simulink model "FeedBack_Linearization"  (R2021b)
(part 7 of 9)

et595 = ct{386};
et596 = ct{387};
et597 = ct{388};
et598 = ct{389};
et599 = ct{390};
et600 = ct{391};
et601 = ct{392};
et602 = ct{393};
et603 = ct{394};
et604 = ct{395};
et605 = ct{396};
et606 = ct{397};
et607 = ct{398};
et608 = ct{399};
et609 = ct{400};
et610 = ct{401};
et611 = ct{402};
et612 = ct{403};
et613 = ct{404};
et614 = ct{405};
et615 = ct{406};
et616 = ct{407};
et617 = ct{408};
et618 = ct{409};
et619 = ct{410};
et620 = ct{411};
et621 = ct{412};
et622 = ct{413};
et623 = ct{414};
et624 = ct{415};
et625 = ct{416};
et626 = ct{417};
et627 = ct{418};
et628 = ct{419};
et629 = ct{420};
et630 = ct{421};
et631 = ct{422};
et632 = ct{423};
et633 = ct{424};
et634 = ct{425};
et635 = ct{426};
et636 = ct{427};
et637 = ct{428};
et638 = ct{429};
et639 = ct{430};
et640 = ct{431};
et641 = ct{432};
et642 = ct{433};
et643 = ct{434};
et644 = ct{435};
et645 = ct{436};
et646 = ct{437};
et647 = ct{438};
et648 = ct{439};
et649 = ct{440};
et650 = ct{441};
et651 = ct{442};
et652 = ct{443};
et653 = ct{444};
et654 = ct{445};
et655 = ct{446};
et656 = ct{447};
t10 = ct{448};
t1001 = ct{449};
t1012 = ct{450};
t1015 = ct{451};
t1016 = ct{452};
t1017 = ct{453};
t1018 = ct{454};
t1020 = ct{455};
t1021 = ct{456};
t1022 = ct{457};
t1023 = ct{458};
t1024 = ct{459};
t1025 = ct{460};
t1034 = ct{461};
t1036 = ct{462};
t1040 = ct{463};
t1041 = ct{464};
t1051 = ct{465};
t1052 = ct{466};
t1053 = ct{467};
t1054 = ct{468};
t1055 = ct{469};
t1056 = ct{470};
t1059 = ct{471};
t1060 = ct{472};
t1066 = ct{473};
t1067 = ct{474};
t1069 = ct{475};
t107 = ct{476};
t1070 = ct{477};
t1072 = ct{478};
t1075 = ct{479};
t1077 = ct{480};
t1079 = ct{481};
t1081 = ct{482};
t1088 = ct{483};
t1093 = ct{484};
t1094 = ct{485};
t1096 = ct{486};
t1097 = ct{487};
t11 = ct{488};
t1110 = ct{489};
t1113 = ct{490};
t1114 = ct{491};
t1115 = ct{492};
t1123 = ct{493};
t1125 = ct{494};
t1126 = ct{495};
t1128 = ct{496};
t1130 = ct{497};
t1132 = ct{498};
t1136 = ct{499};
t1137 = ct{500};
t114 = ct{501};
t1159 = ct{502};
t1161 = ct{503};
t1172 = ct{504};
t1175 = ct{505};
t1178 = ct{506};
t1179 = ct{507};
t1189 = ct{508};
t1190 = ct{509};
t12 = ct{510};
t1206 = ct{511};
t1207 = ct{512};
t1209 = ct{513};
t1211 = ct{514};
t1212 = ct{515};
t1213 = ct{516};
t1214 = ct{517};
t1215 = ct{518};
t1218 = ct{519};
t1219 = ct{520};
t122 = ct{521};
t1220 = ct{522};
t1226 = ct{523};
t1231 = ct{524};
t1256 = ct{525};
t1267 = ct{526};
t1268 = ct{527};
t1269 = ct{528};
t1273 = ct{529};
t1286 = ct{530};
t1295 = ct{531};
t1296 = ct{532};
t1299 = ct{533};
t13 = ct{534};
t130 = ct{535};
t1304 = ct{536};
t1312 = ct{537};
t1313 = ct{538};
t1315 = ct{539};
t1329 = ct{540};
t1330 = ct{541};
t1339 = ct{542};
t1347 = ct{543};
t1350 = ct{544};
t1351 = ct{545};
t1352 = ct{546};
t1360 = ct{547};
t1368 = ct{548};
t1369 = ct{549};
t1374 = ct{550};
t1375 = ct{551};
t1386 = ct{552};
t1387 = ct{553};
t1389 = ct{554};
t139 = ct{555};
t1391 = ct{556};
t14 = ct{557};
t1424 = ct{558};
t1431 = ct{559};
t1435 = ct{560};
t1441 = ct{561};
t1456 = ct{562};
t1462 = ct{563};
t1467 = ct{564};
t1487 = ct{565};
t1489 = ct{566};
t149 = ct{567};
t1497 = ct{568};
t1498 = ct{569};
t15 = ct{570};
t1506 = ct{571};
t1515 = ct{572};
t1516 = ct{573};
t152 = ct{574};
t1526 = ct{575};
t1528 = ct{576};
t1529 = ct{577};
t1543 = ct{578};
t1546 = ct{579};
t1553 = ct{580};
t1554 = ct{581};
t1569 = ct{582};
t1574 = ct{583};
t1577 = ct{584};
t1578 = ct{585};
t1579 = ct{586};
t1581 = ct{587};
t1582 = ct{588};
t1591 = ct{589};
t160 = ct{590};
t1601 = ct{591};
t1603 = ct{592};
t1604 = ct{593};
t1605 = ct{594};
t1616 = ct{595};
t1622 = ct{596};
t1625 = ct{597};
t1633 = ct{598};
t1635 = ct{599};
t1636 = ct{600};
t1638 = ct{601};
t1643 = ct{602};
t1644 = ct{603};
t1648 = ct{604};
t1649 = ct{605};
t165 = ct{606};
t1654 = ct{607};
t1655 = ct{608};
t1657 = ct{609};
t1658 = ct{610};
t1660 = ct{611};
t1661 = ct{612};
t1662 = ct{613};
t1667 = ct{614};
t1668 = ct{615};
t1672 = ct{616};
t1675 = ct{617};
t1679 = ct{618};
t1681 = ct{619};
t1682 = ct{620};
t1685 = ct{621};
t1686 = ct{622};
t1687 = ct{623};
t1688 = ct{624};
t1697 = ct{625};
t17 = ct{626};
t1700 = ct{627};
t1701 = ct{628};
t1702 = ct{629};
t1707 = ct{630};
t1710 = ct{631};
t1711 = ct{632};
t1715 = ct{633};
t1717 = ct{634};
t1718 = ct{635};
t1719 = ct{636};
t1720 = ct{637};
t1721 = ct{638};
t1723 = ct{639};
t1726 = ct{640};
t1729 = ct{641};
t1734 = ct{642};
t1736 = ct{643};
t1738 = ct{644};
t1742 = ct{645};
t1745 = ct{646};
t1746 = ct{647};
t1748 = ct{648};
t1749 = ct{649};
t1750 = ct{650};
t1751 = ct{651};
t1753 = ct{652};
t1755 = ct{653};
t1760 = ct{654};
t1762 = ct{655};
t1765 = ct{656};
t1766 = ct{657};
t1769 = ct{658};
t1770 = ct{659};
t1771 = ct{660};
t1772 = ct{661};
t1774 = ct{662};
t1776 = ct{663};
t1778 = ct{664};
t1779 = ct{665};
t1791 = ct{666};
t1792 = ct{667};
t1795 = ct{668};
t1798 = ct{669};
t1799 = ct{670};
t180 = ct{671};
t1800 = ct{672};
t1801 = ct{673};
t1802 = ct{674};
t1804 = ct{675};
t1805 = ct{676};
t1806 = ct{677};
t1811 = ct{678};
t1812 = ct{679};
t1814 = ct{680};
t1816 = ct{681};
t1817 = ct{682};
t1819 = ct{683};
t182 = ct{684};
t1822 = ct{685};
t1823 = ct{686};
t1830 = ct{687};
t1836 = ct{688};
t1839 = ct{689};
t1840 = ct{690};
t1842 = ct{691};
t1843 = ct{692};
t1846 = ct{693};
t1849 = ct{694};
t1851 = ct{695};
t1852 = ct{696};
t1853 = ct{697};
t1856 = ct{698};
t1859 = ct{699};
t186 = ct{700};
t1860 = ct{701};
t1861 = ct{702};
t1863 = ct{703};
t1865 = ct{704};
t1866 = ct{705};
t1867 = ct{706};
t1872 = ct{707};
t1873 = ct{708};
t1874 = ct{709};
t1875 = ct{710};
t1876 = ct{711};
t1880 = ct{712};
t1881 = ct{713};
t1883 = ct{714};
t1886 = ct{715};
t1888 = ct{716};
t1889 = ct{717};
t189 = ct{718};
t1890 = ct{719};
t1893 = ct{720};
t1896 = ct{721};
t1898 = ct{722};
t1902 = ct{723};
t1905 = ct{724};
t1908 = ct{725};
t1911 = ct{726};
t1914 = ct{727};
t1917 = ct{728};
t1919 = ct{729};
t1924 = ct{730};
t1927 = ct{731};
t1928 = ct{732};
t1931 = ct{733};
t1932 = ct{734};
t1934 = ct{735};
t1940 = ct{736};
t1942 = ct{737};
t1950 = ct{738};
t1951 = ct{739};
t1953 = ct{740};
t1957 = ct{741};
t1959 = ct{742};
t1960 = ct{743};
t1962 = ct{744};
t1963 = ct{745};
t1969 = ct{746};
t1976 = ct{747};
t1985 = ct{748};
t1993 = ct{749};
t2 = ct{750};
t2000 = ct{751};
t2001 = ct{752};
t2002 = ct{753};
t2003 = ct{754};
t2006 = ct{755};
t2008 = ct{756};
t2010 = ct{757};
t2018 = ct{758};
t2022 = ct{759};
t2026 = ct{760};
t2035 = ct{761};
t2036 = ct{762};
t2041 = ct{763};
t2042 = ct{764};
t2044 = ct{765};
t2046 = ct{766};
t2051 = ct{767};
t2056 = ct{768};
t2058 = ct{769};
t2065 = ct{770};
t2066 = ct{771};
t2071 = ct{772};
t2072 = ct{773};
t2073 = ct{774};
t2074 = ct{775};
t2075 = ct{776};
t2076 = ct{777};
t208 = ct{778};
t2080 = ct{779};
t2081 = ct{780};
t2085 = ct{781};
t2088 = ct{782};
t2089 = ct{783};
t2090 = ct{784};
t2095 = ct{785};
t2096 = ct{786};
t2108 = ct{787};
t2109 = ct{788};
t2111 = ct{789};
t2115 = ct{790};
t2119 = ct{791};
t2125 = ct{792};
t2130 = ct{793};
t2139 = ct{794};
t2147 = ct{795};
t2148 = ct{796};
t2149 = ct{797};
t2151 = ct{798};
t2152 = ct{799};
t2163 = ct{800};
t2164 = ct{801};
t2165 = ct{802};
t2171 = ct{803};
t2173 = ct{804};
t2177 = ct{805};
t2179 = ct{806};
t2180 = ct{807};
t2181 = ct{808};
t2182 = ct{809};
t2183 = ct{810};
t2184 = ct{811};
t2187 = ct{812};
t2196 = ct{813};
t2198 = ct{814};
t2203 = ct{815};
t2205 = ct{816};
t2206 = ct{817};
t2207 = ct{818};
t2208 = ct{819};
t221 = ct{820};
t2212 = ct{821};
t2215 = ct{822};
t2217 = ct{823};
t2219 = ct{824};
t2220 = ct{825};
t2224 = ct{826};
t2227 = ct{827};
t2228 = ct{828};
t223 = ct{829};
t2231 = ct{830};
t2240 = ct{831};
t2246 = ct{832};
t2253 = ct{833};
t2256 = ct{834};
t2258 = ct{835};
t2259 = ct{836};
t2261 = ct{837};
t2262 = ct{838};
t2263 = ct{839};
t2264 = ct{840};
t2266 = ct{841};
t2269 = ct{842};
t2289 = ct{843};
t2296 = ct{844};
t23 = ct{845};
t230 = ct{846};
t2300 = ct{847};
t2301 = ct{848};
t2315 = ct{849};
t2323 = ct{850};
t2326 = ct{851};
t2330 = ct{852};
t234 = ct{853};
t2341 = ct{854};
t2343 = ct{855};
t235 = ct{856};
t2350 = ct{857};
t2351 = ct{858};
t2352 = ct{859};
t2356 = ct{860};
t2357 = ct{861};
t2359 = ct{862};
t236 = ct{863};
t2360 = ct{864};
t2363 = ct{865};
t2365 = ct{866};
t2369 = ct{867};
t237 = ct{868};
t2370 = ct{869};
t2372 = ct{870};
t2374 = ct{871};
t2375 = ct{872};
t2376 = ct{873};
t2379 = ct{874};
t238 = ct{875};
t2380 = ct{876};
t2382 = ct{877};
t2383 = ct{878};
t2384 = ct{879};
t2385 = ct{880};
t2387 = ct{881};
t2388 = ct{882};
t239 = ct{883};
t2392 = ct{884};
t2393 = ct{885};
t2395 = ct{886};
t2399 = ct{887};
t24 = ct{888};
t2400 = ct{889};
t2402 = ct{890};
t2404 = ct{891};
t2407 = ct{892};
t2411 = ct{893};
t2418 = ct{894};
t2429 = ct{895};
t243 = ct{896};
t2435 = ct{897};
t2439 = ct{898};
t244 = ct{899};
t2444 = ct{900};
t2445 = ct{901};
t2447 = ct{902};
t2455 = ct{903};
t2456 = ct{904};
t2460 = ct{905};
t2462 = ct{906};
t2463 = ct{907};
t2466 = ct{908};
t2467 = ct{909};
t2477 = ct{910};
t2482 = ct{911};
t2483 = ct{912};
t2488 = ct{913};
t2496 = ct{914};
t25 = ct{915};
t2501 = ct{916};
t2503 = ct{917};
t2507 = ct{918};
t2513 = ct{919};
t2514 = ct{920};
t2516 = ct{921};
t252 = ct{922};
t2521 = ct{923};
t2522 = ct{924};
t2523 = ct{925};
t253 = ct{926};
t2533 = ct{927};
t2536 = ct{928};
t2537 = ct{929};
t254 = ct{930};
t2541 = ct{931};
t2554 = ct{932};
t2558 = ct{933};
t2560 = ct{934};
t2561 = ct{935};
t2563 = ct{936};
t2569 = ct{937};
t2570 = ct{938};
t2571 = ct{939};
t2576 = ct{940};
t2581 = ct{941};
t2584 = ct{942};
t2585 = ct{943};
t2587 = ct{944};
t259 = ct{945};
t2590 = ct{946};
t2591 = ct{947};
t26 = ct{948};
t2601 = ct{949};
t2602 = ct{950};
t2604 = ct{951};
t2609 = ct{952};
t2610 = ct{953};
t2611 = ct{954};
t2612 = ct{955};
t2613 = ct{956};
t2614 = ct{957};
t2615 = ct{958};
t2617 = ct{959};
t2618 = ct{960};
t2620 = ct{961};
t2621 = ct{962};
t2624 = ct{963};
t2627 = ct{964};
t2631 = ct{965};
t2634 = ct{966};
t2635 = ct{967};
t2637 = ct{968};
t2638 = ct{969};
t2647 = ct{970};
t2648 = ct{971};
t2651 = ct{972};
t2652 = ct{973};
t2653 = ct{974};
t2654 = ct{975};
t2655 = ct{976};
t2656 = ct{977};
t2659 = ct{978};
t2661 = ct{979};
t2662 = ct{980};
t2663 = ct{981};
t2664 = ct{982};
t2667 = ct{983};
t2670 = ct{984};
t2671 = ct{985};
t2672 = ct{986};
t2674 = ct{987};
t2675 = ct{988};
t2677 = ct{989};
t2679 = ct{990};
t268 = ct{991};
t2684 = ct{992};
t2687 = ct{993};
t2689 = ct{994};
t269 = ct{995};
t2690 = ct{996};
t2691 = ct{997};
t2692 = ct{998};
t2693 = ct{999};
t2697 = ct{1000};
t2698 = ct{1001};
t2699 = ct{1002};
t27 = ct{1003};
t2700 = ct{1004};
t2701 = ct{1005};
t2703 = ct{1006};
t2707 = ct{1007};
t2708 = ct{1008};
t2710 = ct{1009};
t2711 = ct{1010};
t2714 = ct{1011};
t2720 = ct{1012};
t2721 = ct{1013};
t2722 = ct{1014};
t2723 = ct{1015};
t2726 = ct{1016};
t2727 = ct{1017};
t2728 = ct{1018};
t2729 = ct{1019};
t2732 = ct{1020};
t2734 = ct{1021};
t2735 = ct{1022};
t2737 = ct{1023};
t2738 = ct{1024};
t2739 = ct{1025};
t2740 = ct{1026};
t2741 = ct{1027};
t2742 = ct{1028};
t2743 = ct{1029};
t2744 = ct{1030};
t2747 = ct{1031};
t2751 = ct{1032};
t2753 = ct{1033};
t2754 = ct{1034};
t2756 = ct{1035};
t2765 = ct{1036};
t2781 = ct{1037};
t2783 = ct{1038};
t2788 = ct{1039};
t2789 = ct{1040};
t279 = ct{1041};
t2790 = ct{1042};
t2792 = ct{1043};
t2795 = ct{1044};
t2796 = ct{1045};
t2797 = ct{1046};
t2798 = ct{1047};
t2799 = ct{1048};
t28 = ct{1049};
t280 = ct{1050};
t2801 = ct{1051};
t2803 = ct{1052};
t2804 = ct{1053};
t2807 = ct{1054};
t2810 = ct{1055};
t2811 = ct{1056};
t2813 = ct{1057};
t2814 = ct{1058};
t2816 = ct{1059};
t2817 = ct{1060};
t2818 = ct{1061};
t2823 = ct{1062};
t2825 = ct{1063};
t2828 = ct{1064};
t2829 = ct{1065};
t2832 = ct{1066};
t2837 = ct{1067};
t2838 = ct{1068};
t2839 = ct{1069};
t284 = ct{1070};
t2840 = ct{1071};
t2841 = ct{1072};
t2842 = ct{1073};
t2844 = ct{1074};
t2854 = ct{1075};
t2857 = ct{1076};
t2861 = ct{1077};
t2864 = ct{1078};
t2868 = ct{1079};
t287 = ct{1080};
t2883 = ct{1081};
t2884 = ct{1082};
t2891 = ct{1083};
t29 = ct{1084};
t290 = ct{1085};
t2900 = ct{1086};
t2907 = ct{1087};
t2914 = ct{1088};
t2922 = ct{1089};
t2923 = ct{1090};
t2925 = ct{1091};
t293 = ct{1092};
t2930 = ct{1093};
t2931 = ct{1094};
t2935 = ct{1095};
t2936 = ct{1096};
t2939 = ct{1097};
t2941 = ct{1098};
t2942 = ct{1099};
t2943 = ct{1100};
t2944 = ct{1101};
t2945 = ct{1102};
t2946 = ct{1103};
t2948 = ct{1104};
t2949 = ct{1105};
t295 = ct{1106};
t2950 = ct{1107};
t2953 = ct{1108};
t2954 = ct{1109};
t2955 = ct{1110};
t2956 = ct{1111};
t2957 = ct{1112};
t296 = ct{1113};
t2960 = ct{1114};
t2961 = ct{1115};
t2962 = ct{1116};
t297 = ct{1117};
t2972 = ct{1118};
t2974 = ct{1119};
t298 = ct{1120};
t2989 = ct{1121};
t2991 = ct{1122};
t2996 = ct{1123};
t2997 = ct{1124};
t2998 = ct{1125};
t2999 = ct{1126};
t3 = ct{1127};
t30 = ct{1128};
t3008 = ct{1129};
t3009 = ct{1130};
t301 = ct{1131};
t3011 = ct{1132};
t3020 = ct{1133};
t3031 = ct{1134};
t3035 = ct{1135};
t3038 = ct{1136};
t3039 = ct{1137};
t3040 = ct{1138};
t3041 = ct{1139};
t3042 = ct{1140};
t3045 = ct{1141};
t3047 = ct{1142};
t3048 = ct{1143};
t3051 = ct{1144};
t3052 = ct{1145};
t3060 = ct{1146};
t3066 = ct{1147};
t3067 = ct{1148};
t3071 = ct{1149};
t3075 = ct{1150};
t3076 = ct{1151};
t3082 = ct{1152};
t3083 = ct{1153};
t3085 = ct{1154};
t3086 = ct{1155};
t3088 = ct{1156};
t3092 = ct{1157};
t3097 = ct{1158};
t3098 = ct{1159};
t3099 = ct{1160};
t31 = ct{1161};
t3104 = ct{1162};
t3107 = ct{1163};
t3112 = ct{1164};
t3113 = ct{1165};
t3120 = ct{1166};
t3121 = ct{1167};
t3122 = ct{1168};
t3124 = ct{1169};
t3126 = ct{1170};
t3128 = ct{1171};
t3130 = ct{1172};
t3131 = ct{1173};
t3132 = ct{1174};
t3133 = ct{1175};
t3140 = ct{1176};
t3141 = ct{1177};
t3142 = ct{1178};
t3143 = ct{1179};
t3148 = ct{1180};
t3152 = ct{1181};
t3153 = ct{1182};
t3154 = ct{1183};
t3155 = ct{1184};
t3159 = ct{1185};
t3161 = ct{1186};
t3162 = ct{1187};
t3163 = ct{1188};
t3165 = ct{1189};
t3166 = ct{1190};
t3168 = ct{1191};
t317 = ct{1192};
t3170 = ct{1193};
t3171 = ct{1194};
t3172 = ct{1195};
t3175 = ct{1196};
t3179 = ct{1197};
t318 = ct{1198};
t3181 = ct{1199};
t3186 = ct{1200};
t319 = ct{1201};
t3190 = ct{1202};
t3192 = ct{1203};
t3193 = ct{1204};
t3194 = ct{1205};
t3195 = ct{1206};
t3196 = ct{1207};
t32 = ct{1208};
t320 = ct{1209};
t3201 = ct{1210};
t3202 = ct{1211};
t3203 = ct{1212};
t3204 = ct{1213};
t3205 = ct{1214};
t3215 = ct{1215};
t3226 = ct{1216};
t3229 = ct{1217};
t3232 = ct{1218};
t3235 = ct{1219};
t3238 = ct{1220};
t3246 = ct{1221};
t3248 = ct{1222};
t3249 = ct{1223};
t3252 = ct{1224};
t3253 = ct{1225};
t3255 = ct{1226};
t3257 = ct{1227};
t3260 = ct{1228};
t3261 = ct{1229};
t3262 = ct{1230};
t3263 = ct{1231};
t3264 = ct{1232};
t3268 = ct{1233};
t3269 = ct{1234};
t3272 = ct{1235};
t3273 = ct{1236};
t3277 = ct{1237};
t3279 = ct{1238};
t3280 = ct{1239};
t3284 = ct{1240};
t3288 = ct{1241};
t3289 = ct{1242};
t329 = ct{1243};
t3290 = ct{1244};
t3291 = ct{1245};
t3292 = ct{1246};
t3293 = ct{1247};
t3294 = ct{1248};
t3295 = ct{1249};
t3296 = ct{1250};
t33 = ct{1251};
t330 = ct{1252};
t3301 = ct{1253};
t331 = ct{1254};
t3311 = ct{1255};
t3312 = ct{1256};
t3313 = ct{1257};
t3315 = ct{1258};
t3316 = ct{1259};
t3321 = ct{1260};
t3324 = ct{1261};
t3336 = ct{1262};
t3340 = ct{1263};
t3342 = ct{1264};
t3356 = ct{1265};
t3357 = ct{1266};
t3358 = ct{1267};
t3359 = ct{1268};
t3360 = ct{1269};
t3361 = ct{1270};
t3362 = ct{1271};
t3363 = ct{1272};
t3364 = ct{1273};
t3365 = ct{1274};
t3366 = ct{1275};
t3369 = ct{1276};
t3372 = ct{1277};
t3375 = ct{1278};
t3377 = ct{1279};
t3382 = ct{1280};
t3384 = ct{1281};
t3386 = ct{1282};
t3388 = ct{1283};
t3392 = ct{1284};
t3393 = ct{1285};
t3395 = ct{1286};
t3397 = ct{1287};
t3398 = ct{1288};
t34 = ct{1289};
t3400 = ct{1290};
t3402 = ct{1291};
t3403 = ct{1292};
t3406 = ct{1293};
t3407 = ct{1294};
t3411 = ct{1295};
t3413 = ct{1296};
t3414 = ct{1297};
t3417 = ct{1298};
t3418 = ct{1299};
t342 = ct{1300};
t3421 = ct{1301};
t3422 = ct{1302};
t3424 = ct{1303};
t3426 = ct{1304};
t3429 = ct{1305};
t3433 = ct{1306};
t3436 = ct{1307};
t3437 = ct{1308};
t3438 = ct{1309};
t3440 = ct{1310};
t3443 = ct{1311};
t3444 = ct{1312};
t3452 = ct{1313};
t346 = ct{1314};
t3460 = ct{1315};
t3468 = ct{1316};
t3470 = ct{1317};
t3476 = ct{1318};
t3479 = ct{1319};
t3480 = ct{1320};
t3481 = ct{1321};
t3482 = ct{1322};
t3483 = ct{1323};
t3486 = ct{1324};
t3488 = ct{1325};
t3489 = ct{1326};
t349 = ct{1327};
t3490 = ct{1328};
t3491 = ct{1329};
t3492 = ct{1330};
t3495 = ct{1331};
t3498 = ct{1332};
t35 = ct{1333};
t3502 = ct{1334};
t3504 = ct{1335};
t3506 = ct{1336};
t3514 = ct{1337};
t3526 = ct{1338};
t3527 = ct{1339};
t3528 = ct{1340};
t3535 = ct{1341};
t3536 = ct{1342};
t3537 = ct{1343};
t3538 = ct{1344};
t3540 = ct{1345};
t3542 = ct{1346};
t3544 = ct{1347};
t3546 = ct{1348};
t3547 = ct{1349};
t3551 = ct{1350};
t3555 = ct{1351};
t3556 = ct{1352};
t3559 = ct{1353};
t3561 = ct{1354};
t36 = ct{1355};
t3610 = ct{1356};
t3617 = ct{1357};
t3618 = ct{1358};
t3619 = ct{1359};
t3620 = ct{1360};
t3625 = ct{1361};
t3626 = ct{1362};
t3627 = ct{1363};
t3628 = ct{1364};
t3640 = ct{1365};
t3641 = ct{1366};
t3642 = ct{1367};
t3643 = ct{1368};
t3644 = ct{1369};
t3645 = ct{1370};
t3646 = ct{1371};
t3648 = ct{1372};
t3649 = ct{1373};
t3651 = ct{1374};
t3652 = ct{1375};
t3653 = ct{1376};
t3654 = ct{1377};
t3655 = ct{1378};
t3658 = ct{1379};
t3660 = ct{1380};
t3661 = ct{1381};
t3662 = ct{1382};
t3663 = ct{1383};
t3664 = ct{1384};
t3665 = ct{1385};
t3666 = ct{1386};
t3667 = ct{1387};
t3668 = ct{1388};
t3669 = ct{1389};
t3670 = ct{1390};
t3671 = ct{1391};
t3672 = ct{1392};
t3673 = ct{1393};
t3674 = ct{1394};
t3679 = ct{1395};
t3685 = ct{1396};
t37 = ct{1397};
t3720 = ct{1398};
t3751 = ct{1399};
t3776 = ct{1400};
t3779 = ct{1401};
t3780 = ct{1402};
t3781 = ct{1403};
t3782 = ct{1404};
t3783 = ct{1405};
t3784 = ct{1406};
t3786 = ct{1407};
t3788 = ct{1408};
t3789 = ct{1409};
t3790 = ct{1410};
t3796 = ct{1411};
t3798 = ct{1412};
t3811 = ct{1413};
t3812 = ct{1414};
t3816 = ct{1415};
t3818 = ct{1416};
t3820 = ct{1417};
t3821 = ct{1418};
t3823 = ct{1419};
t3824 = ct{1420};
t3825 = ct{1421};
t3826 = ct{1422};
t3828 = ct{1423};
t3829 = ct{1424};
t3833 = ct{1425};
t3835 = ct{1426};
t3838 = ct{1427};
t3839 = ct{1428};
t3840 = ct{1429};
t3841 = ct{1430};
t3842 = ct{1431};
t3843 = ct{1432};
t3844 = ct{1433};
t3845 = ct{1434};
t39 = ct{1435};
t4 = ct{1436};
t40 = ct{1437};
t431 = ct{1438};
t433 = ct{1439};
t436 = ct{1440};
t448 = ct{1441};
t45 = ct{1442};
t451 = ct{1443};
t452 = ct{1444};
t455 = ct{1445};
t456 = ct{1446};
t457 = ct{1447};
t458 = ct{1448};
t46 = ct{1449};
t460 = ct{1450};
t461 = ct{1451};
t463 = ct{1452};
t469 = ct{1453};
t49 = ct{1454};
t5 = ct{1455};
t50 = ct{1456};
t51 = ct{1457};
t512 = ct{1458};
t515 = ct{1459};
t516 = ct{1460};
t517 = ct{1461};
t518 = ct{1462};
t522 = ct{1463};
t523 = ct{1464};
t525 = ct{1465};
t527 = ct{1466};
t528 = ct{1467};
t529 = ct{1468};
t530 = ct{1469};
t535 = ct{1470};
t536 = ct{1471};
t537 = ct{1472};
t542 = ct{1473};
t547 = ct{1474};
t548 = ct{1475};
t55 = ct{1476};
t554 = ct{1477};
t567 = ct{1478};
t568 = ct{1479};
t569 = ct{1480};
t57 = ct{1481};
t570 = ct{1482};
t571 = ct{1483};
t572 = ct{1484};
t573 = ct{1485};
t574 = ct{1486};
t58 = ct{1487};
t580 = ct{1488};
t581 = ct{1489};
t583 = ct{1490};
t6 = ct{1491};
t600 = ct{1492};
t601 = ct{1493};
t602 = ct{1494};
t603 = ct{1495};
t604 = ct{1496};
t605 = ct{1497};
t606 = ct{1498};
t607 = ct{1499};
t608 = ct{1500};
t609 = ct{1501};
t61 = ct{1502};
t612 = ct{1503};
t613 = ct{1504};
t614 = ct{1505};
t615 = ct{1506};
t616 = ct{1507};
t617 = ct{1508};
t618 = ct{1509};
t619 = ct{1510};
t621 = ct{1511};
t624 = ct{1512};
t626 = ct{1513};
t629 = ct{1514};
t631 = ct{1515};
t632 = ct{1516};
t633 = ct{1517};
t634 = ct{1518};
t635 = ct{1519};
t637 = ct{1520};
t639 = ct{1521};
t640 = ct{1522};
t642 = ct{1523};
t643 = ct{1524};
t644 = ct{1525};
t646 = ct{1526};
t647 = ct{1527};
t648 = ct{1528};
t649 = ct{1529};
t650 = ct{1530};
t651 = ct{1531};
t652 = ct{1532};
t653 = ct{1533};
t654 = ct{1534};
t656 = ct{1535};
t657 = ct{1536};
t660 = ct{1537};
t661 = ct{1538};
t662 = ct{1539};
t663 = ct{1540};
t664 = ct{1541};
t665 = ct{1542};
t667 = ct{1543};
t67 = ct{1544};
t673 = ct{1545};
t676 = ct{1546};
t677 = ct{1547};
t678 = ct{1548};
t685 = ct{1549};
t687 = ct{1550};
t689 = ct{1551};
t69 = ct{1552};
t691 = ct{1553};
t692 = ct{1554};
t693 = ct{1555};
t694 = ct{1556};
t696 = ct{1557};
t697 = ct{1558};
t698 = ct{1559};
t7 = ct{1560};
t70 = ct{1561};
t702 = ct{1562};
t703 = ct{1563};
t704 = ct{1564};
t705 = ct{1565};
t708 = ct{1566};
t71 = ct{1567};
t72 = ct{1568};
t721 = ct{1569};
t725 = ct{1570};
t726 = ct{1571};
t729 = ct{1572};
t73 = ct{1573};
t730 = ct{1574};
t731 = ct{1575};
t735 = ct{1576};
t743 = ct{1577};
t754 = ct{1578};
t755 = ct{1579};
t756 = ct{1580};
t76 = ct{1581};
t760 = ct{1582};
t762 = ct{1583};
t77 = ct{1584};
t773 = ct{1585};
t774 = ct{1586};
t776 = ct{1587};
t777 = ct{1588};
t778 = ct{1589};
t786 = ct{1590};
t788 = ct{1591};
t79 = ct{1592};
t791 = ct{1593};
t792 = ct{1594};
t795 = ct{1595};
t796 = ct{1596};
t797 = ct{1597};
t8 = ct{1598};
t800 = ct{1599};
t805 = ct{1600};
t806 = ct{1601};
t813 = ct{1602};
t815 = ct{1603};
t817 = ct{1604};
t818 = ct{1605};
t819 = ct{1606};
t82 = ct{1607};
t827 = ct{1608};
t831 = ct{1609};
t835 = ct{1610};
t836 = ct{1611};
t838 = ct{1612};
t839 = ct{1613};
t84 = ct{1614};
t840 = ct{1615};
t841 = ct{1616};
t842 = ct{1617};
t843 = ct{1618};
t846 = ct{1619};
t847 = ct{1620};
t85 = ct{1621};
t853 = ct{1622};
t855 = ct{1623};
t857 = ct{1624};
t859 = ct{1625};
t86 = ct{1626};
t860 = ct{1627};
t863 = ct{1628};
t864 = ct{1629};
t866 = ct{1630};
t870 = ct{1631};
t871 = ct{1632};
t876 = ct{1633};
t877 = ct{1634};
t878 = ct{1635};
t88 = ct{1636};
t880 = ct{1637};
t881 = ct{1638};
t882 = ct{1639};
t884 = ct{1640};
t885 = ct{1641};
t888 = ct{1642};
t889 = ct{1643};
t89 = ct{1644};
t891 = ct{1645};
t896 = ct{1646};
t898 = ct{1647};
t899 = ct{1648};
t9 = ct{1649};
t90 = ct{1650};
t902 = ct{1651};
t907 = ct{1652};
t908 = ct{1653};
t91 = ct{1654};
t911 = ct{1655};
t92 = ct{1656};
t921 = ct{1657};
t926 = ct{1658};
t927 = ct{1659};
t928 = ct{1660};
t930 = ct{1661};
t932 = ct{1662};
t933 = ct{1663};
t935 = ct{1664};
t939 = ct{1665};
t940 = ct{1666};
t942 = ct{1667};
t948 = ct{1668};
t949 = ct{1669};
t952 = ct{1670};
t958 = ct{1671};
t959 = ct{1672};
t966 = ct{1673};
t969 = ct{1674};
t974 = ct{1675};
t975 = ct{1676};
t982 = ct{1677};
t983 = ct{1678};
t984 = ct{1679};
t987 = ct{1680};
t988 = ct{1681};
t992 = ct{1682};
t994 = ct{1683};
et657 = t1295.*t1823.*4.466636216449161e-20+t959.*t2163.*4.466636216449161e-20-t633.*t2816.*9.999999999999998e-6;
et658 = t831.*t2631.*(-9.999999999999998e-6)+t632.*t2832.*9.999999999999998e-6;
et659 = (t243-t786).*(t639-t1128-t2181+dq5.*t13.*(t86-t652)).*(-1.2e-4)-t1070.*(t90-t615).*4.466636216449161e-20;
et660 = t2149.*(t92-t663).*1.2e-4-t2610.*(t88-t617).*9.999999999999998e-6;
et661 = t2828.*(t252-t791).*1.2e-4+t2609.*(t653-t838).*1.2e-4;
et662 = -t3393+t3468-t2343.*(t884+t1578-t2180+t14.*(t639-t1128-t2181+dq5.*t13.*(t86-t652))).*2.900000000000001e-4+t2854.*(t1529+t15.*(t92-t663)).*2.9e-4;
et663 = t3470.*(t1386+t7.*(t88-t617)).*2.900000000000001e-4+t3312.*(t1745+t8.*(t252-t791)).*2.900000000000001e-4;
et664 = t1296.*t3336.*2.9e-4+t1649.*t3619.*2.9e-4;
et665 = t1654.*t3618.*(-2.9e-4)+t2601.*t3120.*2.9e-4;
et666 = t2654.*t3124.*2.9e-4-t2323.*t3617.*2.94e-3;
et667 = t2326.*t3620.*2.94e-3+t2576.*(t1755-t3128+t15.*(t284+t287+t290-t329-t805-t1951)+dq7.*t8.*(t252-t791)).*2.94e-3;
et668 = t2075.*(t958-t2263+dq7.*t1601+t15.*(t642+t896-t1137-t2220)).*(-2.94e-3)+t2074.*(t1036+t1771-t2690+t15.*(t755+t1012-t1905-t2692)).*2.900000000000001e-4;
et669 = t2627.*(t1034-t1750+t2691+t8.*(t755+t1012-t1905-t2692)).*2.94e-3-t2036.*(t631-t885+t1132-t2224).*2.900000000000001e-4;
et670 = t2429+t2672.*(t614+t13.*(t86-t652))-t940.*t2832+t959.*t2816+t2196.*(t90-t615)-t2659.*(t653-t838);
et671 = (-t2447-t2783-t2839+t2841+t3126+t3143+t3232+t2165.*(t92-t663).*1.2e-4+t2828.*(t653-t838).*1.2e-4).*(-1.0./2.0);
et672 = t1296.*(t1529+t15.*(t92-t663)).*(-1.089e-2)-t2075.*(t8.*(t92-t663)+t15.*(t621-t864)).*2.9e-4;
et673 = t1207.*t2036.*2.2e-4+t1654.*t2601.*1.089e-2;
et674 = t1649.*t2654.*(-1.089e-2)+t2074.*t2343.*2.2e-4;
et675 = t2323.*t2576.*(-2.9e-4)+t2326.*t2627.*2.9e-4;
et676 = (t1386+t7.*(t88-t617)).*(t1745+t8.*(t252-t791)).*2.2e-4;
et677 = t2944+t3186-t3205+t1649.*(t878-t1582+t2184+t7.*(t639-t1128-t2181+dq5.*t13.*(t86-t652))).*4.000000000000028e-5+t2196.*(t665+t7.*(t90-t615)).*2.81e-3;
et678 = t3104.*(t614+t13.*(t86-t652)).*(-5.0e-5)+t3099.*(t1386+t7.*(t88-t617)).*4.000000000000028e-5;
et679 = t1685.*t2816.*(-2.81e-3)+t1681.*t2832.*2.81e-3;
et680 = t2000.*t2610.*2.81e-3-t2035.*t2631.*2.81e-3;
et681 = (t243-t786).*(t884+t1578-t2180+t14.*(t639-t1128-t2181+dq5.*t13.*(t86-t652))).*5.0e-5-t3312.*(t252-t791).*5.0e-5;
et682 = t3098.*(t653-t838).*(-5.0e-5)+t817.*(t631-t885+t1132-t2224).*5.0e-5;
et683 = t1296.*(t642+t896-t1137-t2220).*(-4.000000000000028e-5)+t2074.*(t755+t1012-t1873-t2664).*4.000000000000028e-5;
et684 = t1654.*(t1487+t2219-t2864+dq6.*t7.*(t88-t617)).*4.000000000000028e-5;
et685 = (t3104.*(t614+t13.*(t86-t652))-(t243-t786).*(t884+t1578-t2180+t14.*(t639-t1128-t2181+dq5.*t13.*(t86-t652)))+t2854.*(t92-t663)+t3312.*(t252-t791)+t3098.*(t653-t838)-t817.*(t631-t885+t1132-t2224)).*(et230+et231).*(-1.0./2.0)+t3776.*(et232+et233).*3.38795-((t3618.*(t1745+t8.*(t252-t791))-t3313.*(t8.*(t92-t663)+t15.*(t621-t864))+t2036.*t3336-t2343.*t3619-t2576.*t3438+t2627.*(t1034-t1750+t2667+t8.*(t755+t1012-t1873-t2664))).*(et234+et235))./2.0;
et686 = t3610.*(et236+et237+et238+et239+et240+et241+et242+et243+et244).*(-1.0./2.0)-((t3342+t2343.*(t884+t1578-t2180+t14.*(t639-t1128-t2181+dq5.*t13.*(t86-t652)))-t3470.*(t1386+t7.*(t88-t617))-t3312.*(t1745+t8.*(t252-t791))-t2074.*(t1036+t1771-t2690+t15.*(t755+t1012-t1905-t2692))+t2036.*(t631-t885+t1132-t2224)).*(et245+et246))./2.0+et247.*et248;
et687 = t3820.*(t2000.*(t284+t287+t290-t329-t805-t1951)+t2035.*t2671-(t243-t786).*(t878-t1582+t2184+t7.*(t639-t1128-t2181+dq5.*t13.*(t86-t652)))+t2177.*(t621-t864)-t817.*(t642+t896-t1137-t2220)-(t252-t791).*(t1487+t2219-t2864+dq6.*t7.*(t88-t617))).*(-1.0./2.0)-(t3666.*(et249+et250+et251+et252+et253))./2.0-(t3364.*(et254+et255+et256+et257+et258))./2.0+et259.*et260;
et688 = t702.*(t24.*1.16152294893368e-19+t23.*t27.*1.16152294893368e-19+t26.*t27.*1.16152294893368e-19).*(-1.0./2.0)-(t3192.*(et261+et262+et263+et264+et265+et266+et267+et268))./2.0;
et689 = t3779.*(et269+et270).*(3.41e+2./1.0e+2)-t3786.*(et271+et272).*(3.41e+2./1.0e+2)-t3784.*(et273+et274).*(3.41e+2./1.0e+2)+(t3192.*(et275+et276+et277+et278+et279+et280+et281+et282+et283+et284+et285))./2.0-((t573.*t817+t831.*(t243-t786)+(t88-t617).*(t252-t791)).*(et286+et287+et288))./2.0-t3823.*(et289+et290).*3.38795-(et291+et292).*(t221.*(2.1e+1./5.0e+1)+t223.*(2.1e+1./5.0e+1)-t542+t547+t548-t554+t580+t581+t583+t800+t1424+t1726+t1856+t1898+t1934+t2042+t2198+t2231+t2253+t2558+t2581+t2587+t2602+t2991+t2997+t3066+t3075+t3082+t3495+t3498).*3.38795-(t1866.*(et293+et294+et295+et296+et297+et298+et299+et300+et301+et302+et303+et304+et305))./2.0;
et690 = (t1866.*(et306+et307+et308+et309+et310+et311+et312+et313))./2.0-((t3031+t2165.*(t92-t663)+t2828.*(t653-t838)).*(et314+et315+et316+et317+et318+et319+et320))./2.0-t3641.*(et321+et322).*2.61155-t3640.*(et323+et324).*2.61155+((t2854.*(t1529+t15.*(t92-t663))+t1296.*t3336+t1649.*t3619-t1654.*t3618+t2601.*t3120+t2654.*t3124).*(et325+et326))./2.0-t3796.*(et327+et328+et329).*3.5432e-1-(t3272.*(et330+et331+et332+et333+et334+et335+et336))./2.0+(t3476.*(t182+t23.*t72+t26.*t72))./2.0+(t624.*(t1736+t23.*t1717+t26.*t1717))./2.0+(t1025.*(t1751+t23.*t1723+t26.*t1723))./2.0+(t1256.*(t2018+t23.*t2010+t26.*t2010))./2.0;
et691 = t3821.*(et337+et338).*3.5432e-1+(t2384.*(et339+et340+et341+et342+et343+et344+et345+et346))./2.0-(t3826.*(-t573.*t574+t676.*t831+t677.*(t88-t617)))./2.0+(t3788.*(t2356-t607.*t2196+t633.*t2816+t831.*t2631-t632.*t2832+t2610.*(t88-t617)))./2.0-t3776.*(et347+et348).*3.38795+(t3841.*(t1649.*(t614+t13.*(t86-t652))+t1296.*(t92-t663)-t1654.*(t653-t838)))./2.0+(t3546.*(et349+et350+et351+et352+et353))./2.0-t3679.*(et354+et355).*2.61155+((-t2961+t3358+t3312.*(t653-t838)).*(et356+et357+et358+et359+et360+et361+et362+et363+et364))./2.0;
et692 = t3670.*(et365+et366+et367).*(3.41e+2./1.0e+2)-t3671.*(et368+et369+et370).*(3.41e+2./1.0e+2)+((t3124.*(t614+t13.*(t86-t652))+t1296.*t2196-t1654.*t2816+t1649.*t2832+t2854.*(t92-t663)+t3120.*(t653-t838)).*(et371+et372))./2.0-((-t940.*(t614+t13.*(t86-t652))+t959.*(t653-t838)+(t90-t615).*(t92-t663)).*(et373+et374+et375))./2.0;
et693 = t3672.*(t2.*t3.*3.9348e-1+t10.*t29.*2.25e-3-t10.*t31.*3.492e-2).*(-2.4552);
et694 = t3673.*(t3.*t9.*3.9348e-1+t10.*t32.*2.25e-3-t10.*t35.*3.492e-2).*2.4552-(t2533.*(et376+et377+et378+et379+et380+et381+et382+et383))./2.0+(t3783.*(et384+et385+et386+et387+et388))./2.0+((t859-t1791+t1066.*(t86-t652)).*(et389+et390+et391+et392+et393+et394+et395+et396+et397+et398+et399))./2.0;
et695 = t3372.*(et400+et401+et402+et403+et404).*(-1.0./2.0)-(t3838.*(et405+et406+et407+et408+et409))./2.0-((t859-t1791+t1066.*(t86-t652)).*(et410+et411+et412+et413+et414+et415+et416+et417))./2.0+(t2384.*(et418+et419+et420+et421+et422+et423+et424+et425+et426+et427+et428+et429+et430))./2.0-(t3828.*(et431+et432+et433+et434+et435))./2.0+((-t3113+t3418+t2654.*(t884+t1578-t2180+t14.*(t639-t1128-t2181+dq5.*t13.*(t86-t652)))).*(et436+et437+et438+et439+et440+et441+et442+et443))./2.0-(t3788.*(t2356-(t88-t617).*(t284+t287+t290-t329-t805-t1951)+t817.*t1070+t831.*t2671-t2147.*(t243-t786)-t2163.*(t252-t791)))./2.0;
et696 = (t1842+t632.*(t639-t1128-t2181+dq5.*t13.*(t86-t652))+t607.*t2165-t1206.*t1896-t1295.*t1852-t633.*t2828).*(et444+et445).*(-1.0./2.0)-t3790.*(et446+et447).*3.38795+(t3060.*(et448+et449+et450+et451+et452+et453+et454+et455))./2.0+((t2407+t2563+t3085-t3092-t3122+t2147.*(t639-t1128-t2181+dq5.*t13.*(t86-t652))).*(et456+et457+et458+et459+et460))./2.0-((t2056-t2360-t2788-t2807+t3051+t2962.*(t88-t617)).*(et461+et462+et463+et464+et465))./2.0;
et697 = t3641.*(t469+t530+t888.*2.0e-4+t899.*5.267999999999999e-2+t1299+t1347+t1350+t1351+t1389+t1391+t1431+t1441+t1543+t1546+t1605).*2.61155;
et698 = t3640.*(t535+t536+t880.*2.0e-4+t889.*5.267999999999999e-2+t1312+t1313+t1315+t1352+t1467+t1497+t1498+t1506+t1553+t1554+t1577).*2.61155+(t3272.*(et466+et467+et468+et469+et470+et471+et472))./2.0;
et699 = (t3313.*(t8.*(t92-t663)+t15.*(t621-t864))+t2323.*t3617-t2326.*t3620-t2576.*(t1755-t3128+t15.*(t284+t287+t290-t329-t805-t1951)+dq7.*t8.*(t252-t791))+t2075.*(t958-t2263+dq7.*t1601+t15.*(t642+t896-t1137-t2220))-t2627.*(t1034-t1750+t2691+t8.*(t755+t1012-t1905-t2692))).*(et473+et474).*(-1.0./2.0)+((t3140+t3489+t3720+t2832.*(t884+t1578-t2180+t14.*(t639-t1128-t2181+dq5.*t13.*(t86-t652)))+t3436.*(t92-t663)+t3685.*(t653-t838)).*(et475+et476+et477+et478+et479))./2.0-(t3789.*(et480+et481+et482+et483+et484+et485+et486+et487))./2.0;
et700 = (t2326.*(t884+t1578-t2180+t14.*(t639-t1128-t2181+dq5.*t13.*(t86-t652)))+t2854.*(t1529+t15.*(t92-t663))-t2323.*t3312+t2601.*t3098+t2654.*t3104-t2075.*(t631-t885+t1132-t2224)).*(et488+et489).*(-1.0./2.0)+(t3824.*(t572.*t632-t604.*t633+t10.*t11.*t607))./2.0+(t3782.*(et490+et491+et492+et493+et494+et495+et496+et497))./2.0+et498.*et499+et500.*et501+((t3377+t2074.*(t878-t1582+t2184+t7.*(t639-t1128-t2181+dq5.*t13.*(t86-t652)))+t1207.*(t642+t896-t1137-t2220)).*(et502+et503+et504+et505+et506+et507+et508+et509))./2.0;
et701 = (-t2961+t3358+t3312.*(t653-t838)).*(et510+et511+et512+et513+et514+et515+et516+et517+et518).*(-1.0./2.0)+(t3443.*(dq1.*t10.*t23+dq1.*t10.*t26))./2.0+((t607.*t827-t633.*t1206+t632.*t1295).*(et519+et520+et521))./2.0+t3798.*(et522+et523).*3.5432e-1-t3833.*(et524+et525).*3.5432e-1+((t2370-t2949+t2816.*(t88-t617)).*(et526+et527+et528+et529+et530+et531+et532+et533))./2.0;
et702 = t3818.*(-t2999+t1649.*(t878-t1582+t2184+t7.*(t639-t1128-t2181+dq5.*t13.*(t86-t652)))+t3099.*(t1386+t7.*(t88-t617))-t1296.*(t642+t896-t1137-t2220)+t2074.*(t755+t1012-t1873-t2664)+t1654.*(t1487+t2219-t2864+dq6.*t7.*(t88-t617))).*(-1.0./2.0)-(t3476.*(t182+t2.*t3.*t568+t9.*t10.*t567-t3.*t9.*t600+t2.*t10.*t601))./2.0-(t2756.*(et534+et535))./2.0-(t3825.*(t3.*t11.*t606+t10.*t35.*t815+t10.*t31.*(t86-t652)))./2.0;
et703 = (t2817+t3324+t3433.*(t614+t13.*(t86-t652))+t2832.*(t639-t1128-t2181+dq5.*t13.*(t86-t652))+t2974.*(t92-t663)+t3422.*(t653-t838)).*(et536+et537+et538+et539).*(-1.0./2.0)-(t3668.*(-t11.*t208+t107.*t604+t139.*t572+t114.*t604+t149.*t572+t301.*t572+t342.*t604+t4.*t11.*t69-t10.*t32.*t1040+t10.*t29.*t1066+dq3.*t3.*t10.*t25-dq3.*t3.*t10.*t28))./2.0-((t24+t23.*t27+t26.*t27).*(et540+et541+et542+et543+et544+et545))./2.0-((t3502+t3544-t3547+t2972.*(t621-t864)+t2196.*(t642+t896-t1137-t2220)+t2816.*(t1487+t2219-t2864+dq6.*t7.*(t88-t617))).*(et546+et547+et548+et549+et550))./2.0;
et704 = (t436-t448-t452+t460+t537+t796+t1097-t1644-t1875+t1890-t2065+t2205+t2227+t2523-t2537-t2560+t2989+t14.*(t639-t1128-t2181+dq5.*t13.*(t86-t652)).*2.019e-2+dq5.*t6.*(t86-t652).*2.75e-2).*(et551+et552).*(-3.38795)-(t3060.*(et553+et554+et555+et556+et557+et558+et559+et560+et561+et562+et563))./2.0;
et705 = t3842.*(t817.*(t621-t864)-t2000.*(t252-t791)+t2035.*(t243-t786)).*(-1.0./2.0)-(t2533.*(et564+et565+et566+et567+et568+et569+et570+et571+et572+et573+et574+et575+et576))./2.0-(t624.*(et577+et578+et579))./2.0+et580.*et581+et582.*et583+t3781.*(et584+et585).*2.61155+t3780.*(et586+et587).*2.61155-t3798.*(et588+et589).*3.5432e-1-(t3839.*(et590+et591+et592+et593+et594))./2.0+et595.*et596+(t3669.*(t234+t571.*t600+t568.*t605-t10.*t32.*t567-t10.*t29.*t601))./2.0+(t3667.*(-t10.*t569+t3.*t603+t9.*t10.*t818+t2.*t10.*t842-t3.*t9.*t1040+t2.*t3.*t1066))./2.0;
et706 = (t3668.*(t572.*t840+t604.*t841-t10.*t11.*t570+t3.*t11.*t602+t10.*t31.*t1020+t10.*t35.*t1067))./2.0+((-t3113+t3418+t2654.*(t884+t1578-t2180+t14.*(t639-t1128-t2181+dq5.*t13.*(t86-t652)))).*(et597+et598+et599+et600+et601+et602+et603+et604))./2.0-((t1880+t1206.*t1860+t940.*t2147+t1295.*t1823+t959.*t2163-t1070.*(t90-t615)).*(et605+et606))./2.0-(t1256.*(et607+et608+et609+et610))./2.0-(t3840.*(-t1207.*(t665+t7.*(t90-t615))+t1685.*(t1386+t7.*(t88-t617))+t1681.*t2074))./2.0-(t3845.*(t1207.*t2036+t2074.*t2343+(t1386+t7.*(t88-t617)).*(t1745+t8.*(t252-t791))))./2.0;
et707 = (t436-t448-t452+t460+t537+t796+t1097-t1644-t1875+t1890-t2065+t2205+t2227+t2523-t2537-t2560+t2989+t14.*(t639-t1128-t2181+dq5.*t13.*(t86-t652)).*2.019e-2+dq5.*t6.*(t86-t652).*2.75e-2).*(et611+et612).*3.38795-(t3440.*(t9.*t568+t2.*t600))./2.0+(t2943.*(et613+et614+et615+et616+et617))./2.0;
et708 = (t3377+t2074.*(t878-t1582+t2184+t7.*(t639-t1128-t2181+dq5.*t13.*(t86-t652)))+t1207.*(t642+t896-t1137-t2220)).*(et618+et619+et620+et621+et622+et623+et624+et625).*(-1.0./2.0)-t3796.*(et626+et627).*3.5432e-1+((t3342-(t1386+t7.*(t88-t617)).*(t1753+t2661+t3107-dq7.*t15.*(t252-t791))-t1649.*t3620+t1654.*t3617+t2074.*t3460+t1296.*(t958-t2263+dq7.*t1601+t15.*(t642+t896-t1137-t2220))).*(et628+et629))./2.0-((t2370-t2949+t2816.*(t88-t617)).*(et630+et631+et632+et633+et634+et635+et636+et637))./2.0-(t1025.*(et638+et639+et640))./2.0;
et709 = (t3811.*(-t10.*t29.*t572+t10.*t32.*t604+t3.*t4.*t10.*t11))./2.0-t3670.*(et641+et642).*(3.41e+2./1.0e+2)+t3671.*(et643+et644).*(3.41e+2./1.0e+2)-(t3667.*(t10.*t51.*-2.0+dq3.*t4.*t24+t10.*t23.*t51.*2.0+t10.*t26.*t51.*2.0+dq3.*t4.*t23.*t27+dq3.*t4.*t26.*t27))./2.0;
et710 = t3252.*(t10.*3.9348e-1-t3.*t4.*2.25e-3+t3.*t11.*3.492e-2).*2.4552+(t3782.*(et645+et646+et647+et648+et649+et650+et651+et652))./2.0+(t3843.*(t1296.*(t1529+t15.*(t92-t663))-t1654.*t2601+t1649.*t2654))./2.0;
et711 = (t3818.*(-t2999-t1681.*(t884+t1578-t2180+t14.*(t639-t1128-t2181+dq5.*t13.*(t86-t652)))+t3121.*(t1386+t7.*(t88-t617))+t1685.*t3312+(t665+t7.*(t90-t615)).*(t631-t885+t1132-t2224)+t2074.*(t755+t1012-t1905-t2692)))./2.0-(t3669.*(t234+t37.*t571+t46.*t605+t49.*t605+t186.*t571-dq3.*t11.*t27-t2.*t3.*t1020-t3.*t9.*t1067))./2.0+(t3844.*(t2075.*(t8.*(t92-t663)+t15.*(t621-t864))+t2323.*t2576-t2326.*t2627))./2.0-t3835.*(et653+et654).*3.5432e-1;
et712 = t3820.*(t2196.*(t665+t7.*(t90-t615))-t1685.*t2816+t1681.*t2832+t2000.*t2610-t2035.*t2631-t2177.*(t621-t864)).*(-1.0./2.0)-((t3031+t2165.*(t92-t663)+t2828.*(t653-t838)).*(et655+et656+et657+et658+et659+et660+et661))./2.0-(t3789.*(et662+et663+et664+et665+et666+et667+et668+et669))./2.0;
et713 = t2296.*(t24.*8.909980864224564e-21+t23.*t27.*8.909980864224564e-21+t26.*t27.*8.909980864224564e-21).*(-1.0./2.0)-(t3812.*(t11.*t24+t11.*t23.*t27+t11.*t26.*t27))./2.0;
et714 = t3816.*(t4.*t27+t3.*t9.*t571-t2.*t3.*t605).*(-1.0./2.0)-t3249.*(t2.*t3.*1.6669e-1-t2.*t10.*7.669999999999999e-3).*4.50275;
et715 = t3248.*(t3.*t9.*1.6669e-1-t9.*t10.*7.669999999999999e-3).*(-4.50275)+et670.*et671-(t3829.*(et672+et673+et674+et675+et676))./2.0-(t3610.*(et677+et678+et679+et680+et681+et682+et683+et684))./2.0;
et716 = t17.*cos(t1021).*sin(t1021).*1.2537630455875e-1;
et717 = -t3291+t3365.*2.900000000000001e-4+t3527+t3642+t3654-t3662-t3665+t2654.*(t884+t1578-t2180+t14.*(t639-t1128-t2181+dq5.*t13.*(t86-t652))).*2.9e-4;
et718 = t3336.*(t8.*(t92-t663)+t15.*(t621-t864)).*2.94e-3;
et719 = t731.*1.9738e-1+t756-t1051.*2.324e-2-t1054.*3.466000000000001e-2+t1081.*1.9738e-1;
et720 = t1883.*(-2.324e-2)+t8.*(t735-t1077).*3.466000000000001e-2;
et721 = t2392.*(t1386+t7.*(t88-t617)).*2.900000000000001e-4+t1655.*(t8.*(t92-t663)+t15.*(t621-t864)).*2.94e-3;
et722 = t1207.*t1686.*(-2.900000000000001e-4)+t1778.*t2601.*2.9e-4;
et723 = t1729.*t2654.*2.9e-4-t2074.*t2382.*2.900000000000001e-4;
et724 = t2383.*t2576.*2.94e-3+t2376.*t2627.*2.94e-3;
et725 = (t1529+t15.*(t92-t663)).*(t254-t729).*2.9e-4;
et726 = t2687.*(t614+t13.*(t86-t652)).*4.466636216449161e-20+t152.*t827.*2.840000000000012e-3;
et727 = t160.*t827.*2.840000000000012e-3+t165.*t827.*2.840000000000012e-3;
et728 = t678.*t1070.*(-1.0e-5)+t708.*t1206.*2.840000000000012e-3;
et729 = t637.*t1295.*2.840000000000012e-3-t1079.*t1206.*2.840000000000012e-3;
et730 = t1126.*t1295.*(-2.840000000000012e-3)-t573.*t1863.*1.0e-5;
et731 = t634.*t2196.*4.466636216449161e-20+t1023.*t2147.*1.0e-5;
et732 = t1022.*t2163.*(-1.0e-5)-t831.*t2707.*1.0e-5;
et733 = t1041.*t2816.*(-4.466636216449161e-20)-t1893.*(t92-t663).*4.466636216449161e-20+t2723.*(t88-t617).*1.0e-5;
et734 = t2832.*(t643-t662).*4.466636216449161e-20+t2722.*(t653-t838).*4.466636216449161e-20;
et735 = t12.*t572.*(t639-t1128-t2181+dq5.*t13.*(t86-t652)).*2.840000000000012e-3+t11.*t36.*t2165.*2.840000000000012e-3;
et736 = t12.*t604.*t2828.*2.840000000000012e-3;
et737 = t2687.*(t614+t13.*(t86-t652)).*1.2e-4+t152.*t827.*4.466636216449161e-20+t160.*t827.*4.466636216449161e-20;
et738 = t165.*t827.*4.466636216449161e-20+t678.*t1070.*9.999999999999998e-6+t708.*t1206.*4.466636216449161e-20;
et739 = t637.*t1295.*4.466636216449161e-20-t1079.*t1206.*4.466636216449161e-20-t1126.*t1295.*4.466636216449161e-20;
et740 = t573.*t1863.*9.999999999999998e-6+t634.*t2196.*1.2e-4;
et741 = t1023.*t2147.*(-9.999999999999998e-6)+t1022.*t2163.*9.999999999999998e-6;
et742 = t831.*t2707.*9.999999999999998e-6-t1041.*t2816.*1.2e-4;
et743 = t1893.*(t92-t663).*(-1.2e-4)-t2723.*(t88-t617).*9.999999999999998e-6;
et744 = t2832.*(t643-t662).*1.2e-4+t2722.*(t653-t838).*1.2e-4;
et745 = t12.*t572.*(t639-t1128-t2181+dq5.*t13.*(t86-t652)).*4.466636216449161e-20+t11.*t36.*t2165.*4.466636216449161e-20+t12.*t604.*t2828.*4.466636216449161e-20;
et746 = -t3289+t3365.*2.2e-4+t3526+t3644+t3655-t3661-t3664+t2654.*(t884+t1578-t2180+t14.*(t639-t1128-t2181+dq5.*t13.*(t86-t652))).*1.089e-2;
et747 = t3336.*(t8.*(t92-t663)+t15.*(t621-t864)).*2.9e-4;
et748 = t2393+t2411+t3.*t602.*7.000000000000001e-5+t567.*t604.*7.000000000000022e-5;
et749 = t572.*t601.*(-7.000000000000022e-5)-t605.*t1020.*7.299999999999999e-4;
et750 = t571.*t1067.*7.299999999999999e-4-t572.*t1066.*7.299999999999999e-4;
et751 = t604.*t1040.*(-7.299999999999999e-4)-dq2.*t11.*t27.*7.000000000000022e-5;
et752 = t10.*t11.*t569.*7.299999999999999e-4-t4.*t10.*t602.*7.299999999999999e-4;
et753 = t2638+t2652+t40.*t606.*1.11e-3-t67.*t606.*1.11e-3;
et754 = t122.*t573.*4.988e-2+t130.*t573.*4.988e-2;
et755 = t180.*t573.*(-4.988e-2)+t626.*t831.*4.988e-2;
et756 = t604.*t1079.*2.24e-3+t572.*t1126.*2.24e-3;
et757 = t831.*t1115.*4.988e-2-t5.*t2350.*4.988e-2;
et758 = t5.*t2369.*4.988e-2-t571.*t2164.*1.11e-3;
et759 = t605.*t2148.*1.11e-3-t667.*(t88-t617).*4.988e-2;
et760 = t1075.*(t88-t617).*(-4.988e-2)-dq4.*t5.*t608.*1.12e-3;
et761 = dq4.*t5.*t635.*(-1.12e-3)-t10.*t28.*t55.*2.24e-3;
et762 = t4.*t10.*t1069.*1.11e-3-t11.*t34.*t1070.*4.988e-2;
et763 = dq4.*t5.*t27.*t28.*(-1.12e-3)-dq3.*t4.*t11.*t12.*t27.*2.24e-3;
et764 = (t1819+t1840+t602.*t606-t604.*t1075-t572.*t1115+t11.*t34.*t569).*(t2388+t2445.*1.11e-3-t2467+t2496-t2693-t2798+t2810+t2829+t1066.*(t86-t652).*1.144e-2);
et765 = -1.0./2.0;
et766 = t525+t528+t529-t855.*1.9738e-1+t1648+t1816+t1817+t1836+t1874.*2.324e-2+t1876.*3.466000000000001e-2+t1919.*1.9738e-1+t1969+t1985;
et767 = t2613.*(-3.466000000000001e-2)+t2615.*2.324e-2;
et768 = t236+t237+t239+t463+t516+t518+t1772+t1962-t1976+t2173-t2614-t2637-t2647+t3009+dq7.*t1601.*2.324e-2+t15.*(t642+t896-t1137-t2220).*2.324e-2+dq7.*t8.*(t92-t663).*3.466000000000001e-2;
et769 = dq7.*t15.*(t621-t864).*3.466000000000001e-2;
et770 = t762.*(-2.019e-2)-t774.*4.9e-4+t778.*2.75e-2+t795+t1113.*2.75e-2;
et771 = t1114.*2.019e-2+t1125.*4.9e-4+t1231+t1643+t1746+t1762+t1766+t2066+t2076+t2115+t2741.*4.9e-4-t2742.*2.019e-2;
et772 = -t3196-t3253-t3262+t3406+t3452+t2074.*(t878-t1582+t2184+t7.*(t639-t1128-t2181+dq5.*t13.*(t86-t652))).*3.0e-5+t2196.*(t621-t864).*5.0e-5;
et773 = t3312.*(t653-t838).*5.000000000000004e-4+t1207.*(t642+t896-t1137-t2220).*3.0e-5;
et774 = t2601.*(t813+t1088+t2739+t7.*(t708-t1079)).*1.089e-2+t2376.*(t884+t1578-t2180+t14.*(t639-t1128-t2181+dq5.*t13.*(t86-t652))).*1.089e-2;
et775 = t2585.*(t1529+t15.*(t92-t663)).*(-1.089e-2)-t3504.*(t1386+t7.*(t88-t617)).*2.2e-4;
et776 = t3086.*(t8.*(t92-t663)+t15.*(t621-t864)).*2.9e-4+t1207.*t3076.*2.2e-4;
et777 = t1686.*t3336.*(-2.9e-4)-t1729.*t3620.*2.2e-4;
et778 = t1778.*t3617.*(-2.2e-4)+t2074.*t3488.*2.2e-4;
et779 = t2383.*t3312.*1.089e-2-t2654.*t3133.*1.089e-2;
et780 = t2382.*t3619.*2.9e-4+t2392.*t3618.*2.9e-4;
et781 = t2576.*t3514.*2.9e-4+t2627.*t3490.*2.9e-4;
et782 = (t254-t729).*(t958-t2263+dq7.*t1601+t15.*(t642+t896-t1137-t2220)).*2.2e-4+t1655.*(t631-t885+t1132-t2224).*1.089e-2;
et783 = t2382.*(t884+t1578-t2180+t14.*(t639-t1128-t2181+dq5.*t13.*(t86-t652))).*2.2e-4-t3506.*(t1386+t7.*(t88-t617)).*2.2e-4;
et784 = t2654.*(-t689+t704+t1159+t1212-t2700).*(-1.089e-2)+(t8.*(t92-t663)+t15.*(t621-t864)).*(t806+t1015-t1917+t2670).*2.9e-4;
et785 = t1207.*t3097.*2.2e-4-t1729.*t3619.*1.089e-2;
et786 = t1778.*t3618.*(-1.089e-2)+t2074.*t3486.*2.2e-4;
et787 = t2392.*t3312.*2.2e-4+t2601.*t3165.*1.089e-2;
et788 = t2376.*t3620.*2.9e-4+t2383.*t3617.*2.9e-4;
et789 = t1655.*(t958-t2263+dq7.*t1601+t15.*(t642+t896-t1137-t2220)).*2.9e-4-t3336.*(t254-t729).*1.089e-2;
et790 = t1686.*(t631-t885+t1132-t2224).*2.2e-4+t2576.*(t1059+t1889-t2744-t3193).*2.9e-4;
et791 = t2627.*(t1060+t1859-t2729+t8.*(-t694+t777+t1161+t1215+t2699)).*2.9e-4+(t1529+t15.*(t92-t663)).*(t295+t297+t298-t331-t760-t1953).*1.089e-2;
et792 = t608.*7.000000000000022e-5+t635.*7.000000000000022e-5;
et793 = t27.*t28.*7.000000000000022e-5-t3.*t4.*t10.*4.999999999999997e-5;
et794 = t9.*t10.*t571.*4.999999999999997e-5-t2.*t10.*t605.*4.999999999999997e-5;
et795 = t1023.*(t884+t1578-t2180+t14.*(t639-t1128-t2181+dq5.*t13.*(t86-t652))).*5.0e-5;
et796 = t1729.*(t878-t1582+t2184+t7.*(t639-t1128-t2181+dq5.*t13.*(t86-t652))).*4.000000000000028e-5-t3133.*(t614+t13.*(t86-t652)).*5.0e-5;
et797 = t2832.*(t650+t7.*(t643-t662)).*2.81e-3+(t653-t838).*(t813+t1088+t2739+t7.*(t708-t1079)).*5.0e-5;
et798 = (t1386+t7.*(t88-t617)).*(t776+t1093-t2737+t14.*(t708-t1079)).*(-4.000000000000028e-5)+t898.*t2196.*2.81e-3;
et799 = t1207.*t2584.*(-4.000000000000028e-5)+t1022.*t3312.*5.0e-5;
et800 = t2000.*t2721.*(-2.81e-3)-t2035.*t2714.*2.81e-3;
et801 = t2074.*(t696+t1094-t2697+t14.*(t637-t1126)).*4.000000000000028e-5-t1830.*(t621-t864).*2.81e-3;
et802 = t2585.*(t92-t663).*(-5.0e-5)+t2816.*(t735-t1077).*2.81e-3;
et803 = t678.*(t631-t885+t1132-t2224).*5.0e-5-t1778.*(t1487+t2219-t2864+dq6.*t7.*(t88-t617)).*4.000000000000028e-5;
et804 = (t254-t729).*(t642+t896-t1137-t2220).*(-4.000000000000028e-5);
et805 = -t3289+t3365.*2.2e-4+t3526+t3644+t3655-t3661-t3664+t2654.*(t884+t1578-t2180+t14.*(t639-t1128-t2181+dq5.*t13.*(t86-t652))).*1.089e-2;
et806 = t3336.*(t8.*(t92-t663)+t15.*(t621-t864)).*2.9e-4;
et807 = t2341+t2445.*4.988e-2-t2463-t2612+t2624-t2796+t2813+t2900+t1066.*(t86-t652).*1.11e-3;
et808 = (t122.*t573+t130.*t573+t346.*t573+t626.*t831+t831.*t1115-t5.*t2350+t5.*t2369-t667.*(t88-t617)-t1075.*(t88-t617)-t11.*t34.*t1070)./2.0;
et809 = t2677-t2679-t602.*t606.*8.8e-4-t573.*t843.*1.12e-3;
et810 = t604.*t1075.*8.8e-4+t572.*t1115.*8.8e-4;
et811 = t12.*t2351.*(-1.12e-3)-t831.*t1770.*1.12e-3;
et812 = t571.*t2163.*3.844e-2-t605.*t2147.*3.844e-2+t12.*t2814;
et813 = t572.*(t637-t1126).*3.844e-2+t604.*(t708-t1079).*3.844e-2;
et814 = t1748.*(t88-t617).*1.12e-3-t11.*t34.*t569.*8.8e-4;
et815 = t10.*t11.*t819.*3.844e-2+t4.*t10.*t1070.*3.844e-2;
et816 = t11.*t36.*t1069.*1.12e-3;
et817 = t604.*t1079.*-2.0-t572.*t1126.*2.0+dq4.*t5.*t608+dq4.*t5.*t635+t10.*t28.*t55.*2.0+dq4.*t5.*t27.*t28+dq3.*t4.*t11.*t12.*t27.*2.0;
et818 = (t2365+t2445.*1.12e-3-t2456+t2536-t2653-t2789+t2803+t2868+t1066.*(t86-t652).*8.8e-4).*(-1.0./2.0);
et819 = t2701-t2703-t602.*t606.*1.144e-2-t573.*t843.*1.11e-3;
et820 = t604.*t1075.*1.144e-2+t572.*t1115.*1.144e-2;
et821 = t12.*t2351.*(-1.11e-3)+t12.*t2372.*1.11e-3;
et822 = t831.*t1770.*(-1.11e-3)+t571.*t2163.*8.8e-4;
et823 = t605.*t2147.*(-8.8e-4)+t572.*(t637-t1126).*8.8e-4;
et824 = t604.*(t708-t1079).*8.8e-4+t1748.*(t88-t617).*1.11e-3;
et825 = t11.*t34.*t569.*(-1.144e-2)+t10.*t11.*t819.*8.8e-4;
et826 = t4.*t10.*t1070.*8.8e-4+t11.*t36.*t1069.*1.11e-3;
et827 = t2679+t2684+t40.*t606.*8.8e-4-t67.*t606.*8.8e-4;
et828 = t122.*t573.*1.12e-3+t130.*t573.*1.12e-3;
et829 = t180.*t573.*(-1.12e-3)+t626.*t831.*1.12e-3;
et830 = t604.*t1079.*7.688e-2+t572.*t1126.*7.688e-2;
et831 = t831.*t1115.*1.12e-3-t5.*t2350.*1.12e-3;
et832 = t571.*t2164.*(-8.8e-4)+t605.*t2148.*8.8e-4+t5.*t2813;
et833 = t667.*(t88-t617).*(-1.12e-3)-t1075.*(t88-t617).*1.12e-3;
et834 = dq4.*t5.*t608.*(-3.844e-2)-dq4.*t5.*t635.*3.844e-2;
et835 = t10.*t28.*t55.*(-7.688e-2)+t4.*t10.*t1069.*8.8e-4;
et836 = t11.*t34.*t1070.*(-1.12e-3)-dq4.*t5.*t27.*t28.*3.844e-2;
et837 = dq3.*t4.*t11.*t12.*t27.*(-7.688e-2);
et838 = t2687.*(t614+t13.*(t86-t652)).*(-9.999999999999998e-6)+t152.*t827.*1.0e-5;
et839 = t160.*t827.*1.0e-5+t165.*t827.*1.0e-5;
et840 = t678.*t1070.*(-2.769999999999999e-3)+t708.*t1206.*1.0e-5;
et841 = t637.*t1295.*1.0e-5-t1079.*t1206.*1.0e-5;
et842 = t1126.*t1295.*(-1.0e-5)-t573.*t1863.*2.769999999999999e-3;
et843 = t634.*t2196.*(-9.999999999999998e-6)+t1023.*t2147.*2.769999999999999e-3;
et844 = t1022.*t2163.*(-2.769999999999999e-3)-t831.*t2707.*2.769999999999999e-3;
et845 = t1041.*t2816.*9.999999999999998e-6+t1893.*(t92-t663).*9.999999999999998e-6;
et846 = t2723.*(t88-t617).*2.769999999999999e-3-t2832.*(t643-t662).*9.999999999999998e-6;
et847 = t2722.*(t653-t838).*(-9.999999999999998e-6)+t12.*t572.*(t639-t1128-t2181+dq5.*t13.*(t86-t652)).*1.0e-5;
et848 = t11.*t36.*t2165.*1.0e-5+t12.*t604.*t2828.*1.0e-5;
et849 = t2601.*(t813+t1088+t2739+t7.*(t708-t1079)).*2.9e-4+t2376.*(t884+t1578-t2180+t14.*(t639-t1128-t2181+dq5.*t13.*(t86-t652))).*2.9e-4;
et850 = t2585.*(t1529+t15.*(t92-t663)).*(-2.9e-4)-t3504.*(t1386+t7.*(t88-t617)).*2.900000000000001e-4;
et851 = t3086.*(t8.*(t92-t663)+t15.*(t621-t864)).*2.94e-3+t1207.*t3076.*2.900000000000001e-4;
et852 = t1686.*t3336.*(-2.94e-3)-t1729.*t3620.*2.900000000000001e-4;
et853 = t1778.*t3617.*(-2.900000000000001e-4)+t2074.*t3488.*2.900000000000001e-4;
et854 = t2383.*t3312.*2.9e-4-t2654.*t3133.*2.9e-4;
et855 = t2382.*t3619.*2.94e-3+t2392.*t3618.*2.94e-3;
et856 = t2576.*t3514.*2.94e-3+t2627.*t3490.*2.94e-3;
et857 = (t254-t729).*(t958-t2263+dq7.*t1601+t15.*(t642+t896-t1137-t2220)).*2.900000000000001e-4+t1655.*(t631-t885+t1132-t2224).*2.9e-4;
et858 = t2382.*(t884+t1578-t2180+t14.*(t639-t1128-t2181+dq5.*t13.*(t86-t652))).*2.900000000000001e-4-t3506.*(t1386+t7.*(t88-t617)).*2.900000000000001e-4;
et859 = t2654.*(-t689+t704+t1159+t1212-t2700).*(-2.9e-4)+(t8.*(t92-t663)+t15.*(t621-t864)).*(t806+t1015-t1917+t2670).*2.94e-3;
et860 = t1207.*t3097.*2.900000000000001e-4-t1729.*t3619.*2.9e-4;
et861 = t1778.*t3618.*(-2.9e-4)+t2074.*t3486.*2.900000000000001e-4;
et862 = t2392.*t3312.*2.900000000000001e-4+t2601.*t3165.*2.9e-4;
et863 = t2376.*t3620.*2.94e-3+t2383.*t3617.*2.94e-3;
et864 = t1655.*(t958-t2263+dq7.*t1601+t15.*(t642+t896-t1137-t2220)).*2.94e-3-t3336.*(t254-t729).*2.9e-4;
et865 = t1686.*(t631-t885+t1132-t2224).*2.900000000000001e-4+t2576.*(t1059+t1889-t2744-t3193).*2.94e-3;
et866 = t2627.*(t1060+t1859-t2729+t8.*(-t694+t777+t1161+t1215+t2699)).*2.94e-3+(t1529+t15.*(t92-t663)).*(t295+t297+t298-t331-t760-t1953).*2.9e-4;
et867 = t2402+t2435+t3.*t602.*4.999999999999997e-5-t567.*t604.*2.19e-3;
et868 = t572.*t601.*2.19e-3+t605.*t1020.*7.000000000000022e-5;
et869 = t571.*t1067.*(-7.000000000000022e-5)+t572.*t1066.*7.000000000000022e-5;
et870 = t604.*t1040.*7.000000000000022e-5+dq2.*t11.*t27.*2.19e-3;
et871 = t10.*t11.*t569.*(-7.000000000000022e-5)+t4.*t10.*t602.*7.000000000000022e-5;
et872 = t1023.*(t884+t1578-t2180+t14.*(t639-t1128-t2181+dq5.*t13.*(t86-t652))).*5.000000000000004e-4;
et873 = t1729.*(t878-t1582+t2184+t7.*(t639-t1128-t2181+dq5.*t13.*(t86-t652))).*(-3.0e-5)-t3133.*(t614+t13.*(t86-t652)).*5.000000000000004e-4;
et874 = t2832.*(t650+t7.*(t643-t662)).*5.0e-5+(t653-t838).*(t813+t1088+t2739+t7.*(t708-t1079)).*5.000000000000004e-4;
et875 = (t1386+t7.*(t88-t617)).*(t776+t1093-t2737+t14.*(t708-t1079)).*3.0e-5+t898.*t2196.*5.0e-5;
et876 = t1207.*t2584.*3.0e-5+t1022.*t3312.*5.000000000000004e-4;
et877 = t2000.*t2721.*(-5.0e-5)-t2035.*t2714.*5.0e-5;
et878 = t2074.*(t696+t1094-t2697+t14.*(t637-t1126)).*(-3.0e-5)-t1830.*(t621-t864).*5.0e-5;
et879 = t2585.*(t92-t663).*(-5.000000000000004e-4)+t2816.*(t735-t1077).*5.0e-5;
et880 = t678.*(t631-t885+t1132-t2224).*5.000000000000004e-4+t1778.*(t1487+t2219-t2864+dq6.*t7.*(t88-t617)).*3.0e-5;
et881 = (t254-t729).*(t642+t896-t1137-t2220).*3.0e-5;
et882 = t573.*t678.*2.769999999999999e-3+t831.*t1023.*2.769999999999999e-3;
et883 = (t614+t13.*(t86-t652)).*(t643-t662).*9.999999999999998e-6+t634.*(t92-t663).*9.999999999999998e-6;
et884 = t1022.*(t88-t617).*(-2.769999999999999e-3)-t1041.*(t653-t838).*9.999999999999998e-6;
et885 = t11.*t36.*t827.*1.0e-5+t12.*t604.*t1206.*1.0e-5;
et886 = t12.*t572.*t1295.*1.0e-5;
et887 = t2392.*(t1386+t7.*(t88-t617)).*2.2e-4+t1655.*(t8.*(t92-t663)+t15.*(t621-t864)).*2.9e-4;
et888 = t1207.*t1686.*(-2.2e-4)+t1778.*t2601.*1.089e-2;
et889 = t1729.*t2654.*1.089e-2-t2074.*t2382.*2.2e-4;
et890 = t2383.*t2576.*2.9e-4+t2376.*t2627.*2.9e-4;
et891 = (t1529+t15.*(t92-t663)).*(t254-t729).*1.089e-2;
et892 = t293.*2.75e-2+t295.*2.019e-2+t296.*2.75e-2+t297.*2.019e-2;
et893 = t298.*2.019e-2+t317.*4.9e-4+t318.*4.9e-4+t320.*4.9e-4;
et894 = t330.*(-2.75e-2)+t525+t528+t529+t1267+t1268+t1304+t1360+t1435+t1591+t1765+t1774+t1950.*4.9e-4-t1953.*2.019e-2;
et895 = t2765+t2818-t2907+t3067+t3215+t3235-t3238-t3246+t3268-t3273+t3375+t3551-t3555+t3433.*(t614+t13.*(t86-t652)).*1.2e-4+t2147.*(t639-t1128-t2181+dq5.*t13.*(t86-t652)).*4.466636216449161e-20;
et896 = t2832.*(t639-t1128-t2181+dq5.*t13.*(t86-t652)).*1.2e-4+t2974.*(t92-t663).*1.2e-4;
et897 = t3422.*(t653-t838).*1.2e-4;
et898 = t689.*(-1.9738e-1)-t743+t1159.*1.9738e-1+t1212.*1.9738e-1+t1273+t1814+t1859.*3.466000000000001e-2+t2071-t2089;
et899 = t2700.*(-1.9738e-1)-t2728.*2.324e-2-t2729.*3.466000000000001e-2-t3148.*2.324e-2;
et900 = t8.*(-t694+t777+t1161+t1215+t2699).*3.466000000000001e-2+dq7.*t8.*(t650+t7.*(t643-t662)).*2.324e-2;
et901 = t795+t1231+t1851+t2088+t2095+t2151+t2395+t2399+t2738.*2.324e-2+t2739.*1.9738e-1+t2740.*3.466000000000001e-2;
et902 = t8.*(t776+t1093-t2737+t14.*(t708-t1079)).*3.466000000000001e-2-t15.*(t776+t1093-t2737+t14.*(t708-t1079)).*2.324e-2+t7.*(t708-t1079).*1.9738e-1;
et903 = t2689.*(t614+t13.*(t86-t652)).*1.2e-4+t1023.*(t639-t1128-t2181+dq5.*t13.*(t86-t652)).*1.2e-4;
et904 = t819.*t827.*4.466636216449161e-20+t634.*t1070.*4.466636216449161e-20+t573.*t1830.*9.999999999999998e-6;
et905 = t678.*t2165.*(-1.2e-4)+t1041.*t2163.*4.466636216449161e-20;
et906 = t831.*t2714.*9.999999999999998e-6+t1022.*t2828.*1.2e-4;
et907 = t1865.*(t92-t663).*(-1.2e-4)+t1206.*(t708-t1079).*4.466636216449161e-20;
et908 = t1295.*(t637-t1126).*4.466636216449161e-20-t2721.*(t88-t617).*9.999999999999998e-6+t2147.*(t643-t662).*4.466636216449161e-20;
et909 = t2720.*(t653-t838).*1.2e-4-t11.*t36.*t2196.*9.999999999999998e-6;
et910 = t12.*t572.*t2832.*(-9.999999999999998e-6)-t12.*t604.*t2816.*9.999999999999998e-6;
et911 = t254.*1.9738e-1+t269-t729.*1.9738e-1+t788.*2.324e-2+t792.*3.466000000000001e-2;
et912 = t974.*3.466000000000001e-2-t975.*2.324e-2;
et913 = -t3196-t3253-t3262+t3406+t3452+t2074.*(t878-t1582+t2184+t7.*(t639-t1128-t2181+dq5.*t13.*(t86-t652))).*3.0e-5+t2196.*(t621-t864).*5.0e-5;
et914 = t3312.*(t653-t838).*5.000000000000004e-4+t1207.*(t642+t896-t1137-t2220).*3.0e-5;
et915 = t1729.*(t614+t13.*(t86-t652)).*3.0e-5-t2074.*(t650+t7.*(t643-t662)).*2.32e-3;
et916 = t898.*t1207.*2.32e-3-t1022.*t2000.*4.000000000000028e-5;
et917 = t1023.*t2035.*(-4.000000000000028e-5)+(t1386+t7.*(t88-t617)).*(t735-t1077).*2.32e-3;
et918 = t678.*(t621-t864).*(-4.000000000000028e-5)+t1778.*(t653-t838).*3.0e-5;
et919 = (t92-t663).*(t254-t729).*3.0e-5;
et920 = t1023.*(t884+t1578-t2180+t14.*(t639-t1128-t2181+dq5.*t13.*(t86-t652))).*3.0e-5;
et921 = t1729.*(t878-t1582+t2184+t7.*(t639-t1128-t2181+dq5.*t13.*(t86-t652))).*(-2.32e-3)-t3133.*(t614+t13.*(t86-t652)).*3.0e-5;
et922 = t2832.*(t650+t7.*(t643-t662)).*(-4.000000000000028e-5)+(t653-t838).*(t813+t1088+t2739+t7.*(t708-t1079)).*3.0e-5;
et923 = (t1386+t7.*(t88-t617)).*(t776+t1093-t2737+t14.*(t708-t1079)).*2.32e-3-t898.*t2196.*4.000000000000028e-5;
et924 = t1207.*t2584.*2.32e-3+t1022.*t3312.*3.0e-5;
et925 = t2000.*t2721.*4.000000000000028e-5+t2035.*t2714.*4.000000000000028e-5;
et926 = t2074.*(t696+t1094-t2697+t14.*(t637-t1126)).*(-2.32e-3)+t1830.*(t621-t864).*4.000000000000028e-5;
et927 = t2585.*(t92-t663).*(-3.0e-5)-t2816.*(t735-t1077).*4.000000000000028e-5;
et928 = t678.*(t631-t885+t1132-t2224).*3.0e-5+t1778.*(t1487+t2219-t2864+dq6.*t7.*(t88-t617)).*2.32e-3;
et929 = (t254-t729).*(t642+t896-t1137-t2220).*2.32e-3;
et930 = t2689.*(t614+t13.*(t86-t652)).*(-9.999999999999998e-6)-t1023.*(t639-t1128-t2181+dq5.*t13.*(t86-t652)).*9.999999999999998e-6;
et931 = t819.*t827.*1.0e-5+t634.*t1070.*1.0e-5;
et932 = t573.*t1830.*(-2.769999999999999e-3)+t678.*t2165.*9.999999999999998e-6;
et933 = t1041.*t2163.*1.0e-5-t831.*t2714.*2.769999999999999e-3;
et934 = t1022.*t2828.*(-9.999999999999998e-6)+t1865.*(t92-t663).*9.999999999999998e-6;
et935 = t1206.*(t708-t1079).*1.0e-5+t1295.*(t637-t1126).*1.0e-5;
et936 = t2721.*(t88-t617).*2.769999999999999e-3+t2147.*(t643-t662).*1.0e-5;
et937 = t2720.*(t653-t838).*(-9.999999999999998e-6)+t11.*t36.*t2196.*2.769999999999999e-3;
et938 = t12.*t572.*t2832.*2.769999999999999e-3+t12.*t604.*t2816.*2.769999999999999e-3;
et939 = t762.*1.9738e-1+t795-t1114.*1.9738e-1+t1231+t1851+t2088+t2095+t2151+t2395+t2399+t2742.*1.9738e-1+t2743.*2.324e-2;
et940 = t2744.*3.466000000000001e-2+t3193.*3.466000000000001e-2-t3194.*2.324e-2;
et941 = t573.*t678.*1.0e-5+t831.*t1023.*1.0e-5;
et942 = (t614+t13.*(t86-t652)).*(t643-t662).*(-4.466636216449161e-20)-t634.*(t92-t663).*4.466636216449161e-20;
et943 = t1022.*(t88-t617).*(-1.0e-5)+t1041.*(t653-t838).*4.466636216449161e-20;
et944 = t11.*t36.*t827.*2.840000000000012e-3+t12.*t604.*t1206.*2.840000000000012e-3;
et945 = t12.*t572.*t1295.*2.840000000000012e-3;
et946 = t1819+t1840+t40.*t606+t189.*t606-t571.*t2164+t605.*t2148+t4.*t10.*t1069;
et947 = (t2388+t2445.*1.11e-3-t2467+t2496-t2693-t2798+t2810+t2829+t1066.*(t86-t652).*1.144e-2)./2.0;
et948 = t279.*5.000000000000001e-5+t280.*5.000000000000001e-5+t293.*2.37e-3+t296.*2.37e-3;
et949 = t319.*(-5.000000000000001e-5)-t330.*2.37e-3+t1175+t1178+t1179+t1189+t1190+t1286+t1339+t1368+t1369+t1456+t1569;
et950 = t1729.*(t614+t13.*(t86-t652)).*5.000000000000004e-4-t2074.*(t650+t7.*(t643-t662)).*3.0e-5;
et951 = t898.*t1207.*3.0e-5+t1022.*t2000.*5.0e-5;
et952 = t1023.*t2035.*5.0e-5+(t1386+t7.*(t88-t617)).*(t735-t1077).*3.0e-5;
et953 = t678.*(t621-t864).*5.0e-5+t1778.*(t653-t838).*5.000000000000004e-4;
et954 = (t92-t663).*(t254-t729).*5.000000000000004e-4;
et955 = t2635-t2638-t602.*t606.*1.11e-3-t573.*t843.*4.988e-2;
et956 = t604.*t1075.*1.11e-3+t572.*t1115.*1.11e-3;
et957 = t12.*t2351.*(-4.988e-2)+t12.*t2372.*4.988e-2;
et958 = t831.*t1770.*(-4.988e-2)+t571.*t2163.*1.12e-3;
et959 = t605.*t2147.*(-1.12e-3)+t572.*(t637-t1126).*1.12e-3;
et960 = t604.*(t708-t1079).*1.12e-3+t1748.*(t88-t617).*4.988e-2;
et961 = t11.*t34.*t569.*(-1.11e-3)+t10.*t11.*t819.*1.12e-3;
et962 = t4.*t10.*t1070.*1.12e-3+t11.*t36.*t1069.*4.988e-2;
et963 = (t614+t13.*(t86-t652)).*(-t689+t704+t1159+t1212-t2700).*5.0e-5-t1023.*(t878-t1582+t2184+t7.*(t639-t1128-t2181+dq5.*t13.*(t86-t652))).*2.81e-3;
et964 = t3166.*(t1386+t7.*(t88-t617)).*4.000000000000028e-5-(t92-t663).*(t295+t297+t298-t331-t760-t1953).*5.0e-5;
et965 = t1207.*t2634.*4.000000000000028e-5+t1729.*t2832.*5.0e-5;
et966 = t1778.*t2816.*5.0e-5+t2000.*t2723.*2.81e-3;
et967 = t2035.*t2707.*2.81e-3+t2196.*(t254-t729).*5.0e-5;
et968 = t1863.*(t621-t864).*2.81e-3-t3165.*(t653-t838).*5.0e-5;
et969 = t3312.*(t735-t1077).*4.000000000000028e-5-t678.*(t642+t896-t1137-t2220).*2.81e-3;
et970 = t898.*(t631-t885+t1132-t2224).*(-4.000000000000028e-5)+t1022.*(t1487+t2219-t2864+dq6.*t7.*(t88-t617)).*2.81e-3;
et971 = t2074.*(-t694+t777+t1161+t1215+t2699).*4.000000000000028e-5+(t650+t7.*(t643-t662)).*(t884+t1578-t2180+t14.*(t639-t1128-t2181+dq5.*t13.*(t86-t652))).*4.000000000000028e-5;
et972 = t12.*t608.*3.844e-2+t12.*t635.*3.844e-2;
et973 = t571.*t815.*8.8e-4-t605.*(t86-t652).*8.8e-4;
et974 = t12.*t27.*t28.*3.844e-2-t11.*t34.*t573.*1.12e-3;
et975 = t4.*t10.*t606.*(-8.8e-4)+t5.*t572.*t831.*1.12e-3;
et976 = t5.*t604.*(t88-t617).*(-1.12e-3);
et977 = t2703+t2708+t40.*t606.*1.144e-2-t67.*t606.*1.144e-2;
et978 = t122.*t573.*1.11e-3+t130.*t573.*1.11e-3;
et979 = t180.*t573.*(-1.11e-3)+t626.*t831.*1.11e-3;
et980 = t604.*t1079.*1.76e-3+t572.*t1126.*1.76e-3;
et981 = t831.*t1115.*1.11e-3-t5.*t2350.*1.11e-3;
et982 = t5.*t2369.*1.11e-3-t571.*t2164.*1.144e-2;
et983 = t605.*t2148.*1.144e-2-t667.*(t88-t617).*1.11e-3;
et984 = t1075.*(t88-t617).*(-1.11e-3)-dq4.*t5.*t608.*8.8e-4;
et985 = dq4.*t5.*t635.*(-8.8e-4)-t10.*t28.*t55.*1.76e-3;
et986 = t4.*t10.*t1069.*1.144e-2-t11.*t34.*t1070.*1.11e-3;
et987 = dq4.*t5.*t27.*t28.*(-8.8e-4)-dq3.*t4.*t11.*t12.*t27.*1.76e-3;
et988 = (t614+t13.*(t86-t652)).*(-t689+t704+t1159+t1212-t2700).*5.000000000000004e-4-t1023.*(t878-t1582+t2184+t7.*(t639-t1128-t2181+dq5.*t13.*(t86-t652))).*5.0e-5;
et989 = t3166.*(t1386+t7.*(t88-t617)).*(-3.0e-5)-(t92-t663).*(t295+t297+t298-t331-t760-t1953).*5.000000000000004e-4;
et990 = t1207.*t2634.*(-3.0e-5)+t1729.*t2832.*5.000000000000004e-4;
et991 = t1778.*t2816.*5.000000000000004e-4+t2000.*t2723.*5.0e-5;
et992 = t2035.*t2707.*5.0e-5+t2196.*(t254-t729).*5.000000000000004e-4;
et993 = t1863.*(t621-t864).*5.0e-5-t3165.*(t653-t838).*5.000000000000004e-4;
et994 = t3312.*(t735-t1077).*(-3.0e-5)-t678.*(t642+t896-t1137-t2220).*5.0e-5;
et995 = t898.*(t631-t885+t1132-t2224).*3.0e-5+t1022.*(t1487+t2219-t2864+dq6.*t7.*(t88-t617)).*5.0e-5;
et996 = t2074.*(-t694+t777+t1161+t1215+t2699).*(-3.0e-5)-(t650+t7.*(t643-t662)).*(t884+t1578-t2180+t14.*(t639-t1128-t2181+dq5.*t13.*(t86-t652))).*3.0e-5;
et997 = t573.*t678.*(-9.999999999999998e-6)-t831.*t1023.*9.999999999999998e-6;
et998 = (t614+t13.*(t86-t652)).*(t643-t662).*(-1.2e-4)-t634.*(t92-t663).*1.2e-4;
et999 = t1022.*(t88-t617).*9.999999999999998e-6+t1041.*(t653-t838).*1.2e-4;
et1000 = t11.*t36.*t827.*4.466636216449161e-20+t12.*t604.*t1206.*4.466636216449161e-20+t12.*t572.*t1295.*4.466636216449161e-20;
et1001 = t84.*(-2.75e-2)+t253.*2.75e-2+t254.*2.019e-2+t259.*4.9e-4-t269;
et1002 = t725.*4.9e-4-t729.*2.019e-2;
et1003 = t2404+t2439+t3.*t602.*2.23e-3-t567.*t604.*4.999999999999997e-5;
et1004 = t572.*t601.*4.999999999999997e-5-t605.*t1020.*7.000000000000001e-5;
et1005 = t571.*t1067.*7.000000000000001e-5-t572.*t1066.*7.000000000000001e-5;
et1006 = t604.*t1040.*(-7.000000000000001e-5)+dq2.*t11.*t27.*4.999999999999997e-5;
et1007 = t10.*t11.*t569.*7.000000000000001e-5-t4.*t10.*t602.*7.000000000000001e-5;
et1008 = t613.*2.75e-2+t730.*2.75e-2+t731.*2.019e-2+t735.*4.9e-4-t756;
et1009 = t1077.*(-4.9e-4)+t1081.*2.019e-2;
et1010 = (t614+t13.*(t86-t652)).*(-t689+t704+t1159+t1212-t2700).*(-3.0e-5)-t1023.*(t878-t1582+t2184+t7.*(t639-t1128-t2181+dq5.*t13.*(t86-t652))).*4.000000000000028e-5;
et1011 = t3166.*(t1386+t7.*(t88-t617)).*2.32e-3+(t92-t663).*(t295+t297+t298-t331-t760-t1953).*3.0e-5;
et1012 = t1207.*t2634.*2.32e-3-t1729.*t2832.*3.0e-5;
et1013 = t1778.*t2816.*(-3.0e-5)+t2000.*t2723.*4.000000000000028e-5;
et1014 = t2035.*t2707.*4.000000000000028e-5-t2196.*(t254-t729).*3.0e-5;
et1015 = t1863.*(t621-t864).*4.000000000000028e-5+t3165.*(t653-t838).*3.0e-5;
et1016 = t3312.*(t735-t1077).*2.32e-3-t678.*(t642+t896-t1137-t2220).*4.000000000000028e-5;
et1017 = t898.*(t631-t885+t1132-t2224).*(-2.32e-3)+t1022.*(t1487+t2219-t2864+dq6.*t7.*(t88-t617)).*4.000000000000028e-5;
et1018 = t2074.*(-t694+t777+t1161+t1215+t2699).*2.32e-3+(t650+t7.*(t643-t662)).*(t884+t1578-t2180+t14.*(t639-t1128-t2181+dq5.*t13.*(t86-t652))).*2.32e-3;
et1019 = t1729.*(t614+t13.*(t86-t652)).*5.0e-5+t2074.*(t650+t7.*(t643-t662)).*4.000000000000028e-5;
et1020 = t898.*t1207.*(-4.000000000000028e-5)+t1022.*t2000.*2.81e-3;
et1021 = t1023.*t2035.*2.81e-3-(t1386+t7.*(t88-t617)).*(t735-t1077).*4.000000000000028e-5;
et1022 = t678.*(t621-t864).*2.81e-3+t1778.*(t653-t838).*5.0e-5;
et1023 = (t92-t663).*(t254-t729).*5.0e-5;
et1024 = -t3294+t3365.*7.950000000000001e-3+t3528+t3648+t3658-t3660-t3663+t2654.*(t884+t1578-t2180+t14.*(t639-t1128-t2181+dq5.*t13.*(t86-t652))).*2.2e-4;
et1025 = t3336.*(t8.*(t92-t663)+t15.*(t621-t864)).*2.900000000000001e-4;
et1026 = -t795+t1172-t1643+t1719+t1742-t1762-t1804.*2.75e-2+t2051-t2066+t2090-t2737.*4.9e-4+t2739.*2.019e-2+t7.*(t708-t1079).*2.019e-2;
et1027 = t14.*(t708-t1079).*4.9e-4;
et1028 = t2601.*(t813+t1088+t2739+t7.*(t708-t1079)).*2.2e-4+t2376.*(t884+t1578-t2180+t14.*(t639-t1128-t2181+dq5.*t13.*(t86-t652))).*2.2e-4;
et1029 = t2585.*(t1529+t15.*(t92-t663)).*(-2.2e-4)-t3504.*(t1386+t7.*(t88-t617)).*7.950000000000001e-3;
et1030 = t3086.*(t8.*(t92-t663)+t15.*(t621-t864)).*2.900000000000001e-4+t1207.*t3076.*7.950000000000001e-3;
et1031 = t1686.*t3336.*(-2.900000000000001e-4)-t1729.*t3620.*7.950000000000001e-3;
et1032 = t1778.*t3617.*(-7.950000000000001e-3)+t2074.*t3488.*7.950000000000001e-3;
et1033 = t2383.*t3312.*2.2e-4-t2654.*t3133.*2.2e-4;
et1034 = t2382.*t3619.*2.900000000000001e-4+t2392.*t3618.*2.900000000000001e-4;
et1035 = t2576.*t3514.*2.900000000000001e-4+t2627.*t3490.*2.900000000000001e-4;
et1036 = (t254-t729).*(t958-t2263+dq7.*t1601+t15.*(t642+t896-t1137-t2220)).*7.950000000000001e-3+t1655.*(t631-t885+t1132-t2224).*2.2e-4;
et1037 = t2382.*(t884+t1578-t2180+t14.*(t639-t1128-t2181+dq5.*t13.*(t86-t652))).*7.950000000000001e-3-t3506.*(t1386+t7.*(t88-t617)).*7.950000000000001e-3;
et1038 = t2654.*(-t689+t704+t1159+t1212-t2700).*(-2.2e-4)+(t8.*(t92-t663)+t15.*(t621-t864)).*(t806+t1015-t1917+t2670).*2.900000000000001e-4;
et1039 = t1207.*t3097.*7.950000000000001e-3-t1729.*t3619.*2.2e-4;
et1040 = t1778.*t3618.*(-2.2e-4)+t2074.*t3486.*7.950000000000001e-3;
et1041 = t2392.*t3312.*7.950000000000001e-3+t2601.*t3165.*2.2e-4;
et1042 = t2376.*t3620.*2.900000000000001e-4+t2383.*t3617.*2.900000000000001e-4;
et1043 = t1655.*(t958-t2263+dq7.*t1601+t15.*(t642+t896-t1137-t2220)).*2.900000000000001e-4-t3336.*(t254-t729).*2.2e-4;
et1044 = t1686.*(t631-t885+t1132-t2224).*7.950000000000001e-3+t2576.*(t1059+t1889-t2744-t3193).*2.900000000000001e-4;
et1045 = t2627.*(t1060+t1859-t2729+t8.*(-t694+t777+t1161+t1215+t2699)).*2.900000000000001e-4+(t1529+t15.*(t92-t663)).*(t295+t297+t298-t331-t760-t1953).*2.2e-4;
et1046 = -t3294+t3365.*7.950000000000001e-3+t3528+t3648+t3658-t3660-t3663+t2654.*(t884+t1578-t2180+t14.*(t639-t1128-t2181+dq5.*t13.*(t86-t652))).*2.2e-4;
et1047 = t3336.*(t8.*(t92-t663)+t15.*(t621-t864)).*2.900000000000001e-4;
et1048 = t2689.*(t614+t13.*(t86-t652))+t1023.*(t639-t1128-t2181+dq5.*t13.*(t86-t652))-t678.*t2165+t1022.*t2828-t1865.*(t92-t663)+t2720.*(t653-t838);
et1049 = (-t2447-t2783-t2839+t2841+t3126+t3143+t3232+t2165.*(t92-t663).*1.2e-4+t2828.*(t653-t838).*1.2e-4)./2.0;
et1050 = t2689.*(t614+t13.*(t86-t652)).*4.466636216449161e-20+t1023.*(t639-t1128-t2181+dq5.*t13.*(t86-t652)).*4.466636216449161e-20;
et1051 = t819.*t827.*2.840000000000012e-3+t634.*t1070.*2.840000000000012e-3;
et1052 = t573.*t1830.*(-1.0e-5)-t678.*t2165.*4.466636216449161e-20;
et1053 = t1041.*t2163.*2.840000000000012e-3-t831.*t2714.*1.0e-5;
et1054 = t1022.*t2828.*4.466636216449161e-20-t1865.*(t92-t663).*4.466636216449161e-20;
et1055 = t1206.*(t708-t1079).*2.840000000000012e-3+t1295.*(t637-t1126).*2.840000000000012e-3;
et1056 = t2721.*(t88-t617).*1.0e-5+t2147.*(t643-t662).*2.840000000000012e-3;
et1057 = t2720.*(t653-t838).*4.466636216449161e-20+t11.*t36.*t2196.*1.0e-5;
et1058 = t12.*t572.*t2832.*1.0e-5+t12.*t604.*t2816.*1.0e-5;
et1059 = t647.*(-1.9738e-1)-t687+t1052.*2.324e-2+t1055.*3.466000000000001e-2+t1849.*2.324e-2;
et1060 = t8.*(t650+t7.*(t643-t662)).*(-3.466000000000001e-2)+t14.*(t643-t662).*1.9738e-1;
et1061 = t2392.*(t1386+t7.*(t88-t617)).*7.950000000000001e-3+t1655.*(t8.*(t92-t663)+t15.*(t621-t864)).*2.900000000000001e-4;
et1062 = t1207.*t1686.*(-7.950000000000001e-3)+t1778.*t2601.*2.2e-4;
et1063 = t1729.*t2654.*2.2e-4-t2074.*t2382.*7.950000000000001e-3;
et1064 = t2383.*t2576.*2.900000000000001e-4+t2376.*t2627.*2.900000000000001e-4;
et1065 = (t1529+t15.*(t92-t663)).*(t254-t729).*2.2e-4;
et1066 = -t2844-t2914-t2922+t3052+t3229-t3264+t3269+t3280-t3284+t3295+t3301+t3369+t3556-t3559+t3433.*(t614+t13.*(t86-t652)).*9.999999999999998e-6;
et1067 = t2832.*(t639-t1128-t2181+dq5.*t13.*(t86-t652)).*9.999999999999998e-6+t2974.*(t92-t663).*9.999999999999998e-6;
et1068 = t3422.*(t653-t838).*9.999999999999998e-6;
et1069 = -t2711+t2801-t2954+t2956-t3179+t3181+t2165.*(t92-t663).*4.466636216449161e-20+t2816.*(t88-t617).*1.0e-5;
et1070 = t2828.*(t653-t838).*4.466636216449161e-20;
et1071 = t743-t1273+t1822+t2089+t2096+t2152+t2385+t2387+t2698.*1.9738e-1+t2726.*2.324e-2+t2727.*3.466000000000001e-2;
et1072 = t8.*(t696+t1094-t2697+t14.*(t637-t1126)).*3.466000000000001e-2-t15.*(t696+t1094-t2697+t14.*(t637-t1126)).*2.324e-2+t7.*(t637-t1126).*1.9738e-1;
et1073 = t689.*(-2.019e-2)-t694.*4.9e-4+t703.*2.75e-2+t743+t1159.*2.019e-2;
et1074 = t1161.*4.9e-4+t1211.*2.75e-2+t1212.*2.019e-2+t1215.*4.9e-4+t1330+t1679-t1688-t1701+t1715-t2008;
et1075 = t2699.*4.9e-4-t2700.*2.019e-2;
et1076 = t608.*7.000000000000001e-5+t635.*7.000000000000001e-5;
et1077 = t27.*t28.*7.000000000000001e-5+t3.*t4.*t10.*2.23e-3;
et1078 = t9.*t10.*t571.*(-2.23e-3)+t2.*t10.*t605.*2.23e-3;
et1079 = t12.*t608.*8.8e-4+t12.*t635.*8.8e-4;
et1080 = t571.*t815.*1.144e-2-t605.*(t86-t652).*1.144e-2;
et1081 = t12.*t27.*t28.*8.8e-4-t11.*t34.*t573.*1.11e-3;
et1082 = t4.*t10.*t606.*(-1.144e-2)+t5.*t572.*t831.*1.11e-3;
et1083 = t5.*t604.*(t88-t617).*(-1.11e-3);
et1084 = t743+t1159.*2.019e-2+t1161.*4.9e-4+t1330+t1679-t1688-t1701+t1715+t1801.*2.75e-2-t2008+t2697.*4.9e-4;
et1085 = t2698.*(-2.019e-2)-t7.*(t637-t1126).*2.019e-2-t14.*(t637-t1126).*4.9e-4;
et1086 = -t3291+t3365.*2.900000000000001e-4+t3527+t3642+t3654-t3662-t3665+t2654.*(t884+t1578-t2180+t14.*(t639-t1128-t2181+dq5.*t13.*(t86-t652))).*2.9e-4;
et1087 = t3336.*(t8.*(t92-t663)+t15.*(t621-t864)).*2.94e-3;
et1088 = t84.*(-2.37e-3)+t91.*5.000000000000001e-5+t244.*5.000000000000001e-5+t253.*2.37e-3;
et1089 = t11.*t36.*(-1.8866e-1);
et1090 = t643.*5.000000000000001e-5+t646.*2.37e-3+t654.*2.37e-3-t662.*5.000000000000001e-5;
et1091 = t12.*t572.*(-1.8866e-1);
et1092 = t613.*2.37e-3-t618.*5.000000000000001e-5+t726.*5.000000000000001e-5+t730.*2.37e-3;
et1093 = t12.*t604.*(-1.8866e-1);
et1094 = t608.*7.299999999999999e-4+t635.*7.299999999999999e-4;
et1095 = t27.*t28.*7.299999999999999e-4+t3.*t4.*t10.*7.000000000000001e-5;
et1096 = t9.*t10.*t571.*(-7.000000000000001e-5)+t2.*t10.*t605.*7.000000000000001e-5;
et1097 = t2003-t2402-t2435+t10.*t57.*4.999999999999997e-5-t4.*t69.*4.999999999999997e-5;
et1098 = t45.*t571.*4.999999999999997e-5+t50.*t571.*4.999999999999997e-5;
et1099 = t39.*t605.*(-4.999999999999997e-5)+t61.*t605.*4.999999999999997e-5;
et1100 = t572.*t1066.*(-1.400000000000004e-4)-t604.*t1040.*1.400000000000004e-4;
et1101 = dq2.*t3.*t10.*t28.*1.400000000000004e-4+dq3.*t4.*t11.*t27.*1.400000000000004e-4;
et1102 = t295.*(-1.9738e-1)-t297.*1.9738e-1-t298.*1.9738e-1+t525+t528+t529+t1648+t1816+t1817+t1836+t1911.*2.324e-2;
et1103 = t1917.*3.466000000000001e-2+t1953.*1.9738e-1+t1969+t1985+t2662.*2.324e-2-t2670.*3.466000000000001e-2;
et1104 = t236+t237+t239+t463+t516+t518+t1772+t1962-t1976+t2173-t2614-t2637-t2647+t3009+dq7.*t1601.*2.324e-2+t15.*(t642+t896-t1137-t2220).*2.324e-2+dq7.*t8.*(t92-t663).*3.466000000000001e-2;
et1105 = dq7.*t15.*(t621-t864).*3.466000000000001e-2;
et1106 = t208.*2.23e-3-t2404-t2439+t10.*t57.*2.23e-3;
et1107 = t4.*t69.*(-2.23e-3)+t45.*t571.*2.23e-3;
et1108 = t50.*t571.*2.23e-3-t39.*t605.*2.23e-3;
et1109 = t61.*t605.*2.23e-3+t572.*t1066.*1.4e-4;
et1110 = t604.*t1040.*1.4e-4-dq2.*t3.*t10.*t28.*1.4e-4;
et1111 = dq3.*t4.*t11.*t27.*(-1.4e-4);
et1112 = -t451-t455-t458+t855.*2.019e-2+t857.*4.9e-4+t902.*2.75e-2+t1267+t1268+t1304+t1360+t1435+t1591+t1765+t1774+t1914.*4.9e-4;
et1113 = t1919.*(-2.019e-2);
et1114 = t646.*2.75e-2+t647.*2.019e-2+t650.*4.9e-4+t654.*2.75e-2-t687;
et1115 = t7.*(t643-t662).*4.9e-4-t14.*(t643-t662).*2.019e-2;
et1116 = t12.*t608.*1.12e-3+t12.*t635.*1.12e-3;
et1117 = t571.*t815.*1.11e-3-t605.*(t86-t652).*1.11e-3;
et1118 = t12.*t27.*t28.*1.12e-3-t11.*t34.*t573.*4.988e-2;
et1119 = t4.*t10.*t606.*(-1.11e-3)+t5.*t572.*t831.*4.988e-2;
et1120 = t5.*t604.*(t88-t617).*(-4.988e-2);
et1121 = t571.*t2163-t605.*t2147+t572.*(t637-t1126)+t604.*(t708-t1079)+t10.*t11.*t819+t4.*t10.*t1070;
et1122 = (t2365+t2445.*1.12e-3-t2456+t2536-t2653-t2789+t2803+t2868+t1066.*(t86-t652).*8.8e-4)./2.0;
et1123 = t208.*7.000000000000001e-5+t2400+t2418+t10.*t57.*7.000000000000001e-5;
et1124 = t4.*t69.*(-7.000000000000001e-5)+t45.*t571.*7.000000000000001e-5;
et1125 = t50.*t571.*7.000000000000001e-5-t39.*t605.*7.000000000000001e-5;
et1126 = t61.*t605.*7.000000000000001e-5+t572.*t1066.*1.46e-3;
et1127 = t604.*t1040.*1.46e-3-dq2.*t3.*t10.*t28.*1.46e-3;
et1128 = dq3.*t4.*t11.*t27.*(-1.46e-3);
et1129 = t2891+t2923+t2941+t3011-t3226+t3277-t3279-t3292+t3296-t3311+t3363+t3479.*1.0e-5+t3561+t3433.*(t614+t13.*(t86-t652)).*4.466636216449161e-20;
et1130 = t2147.*(t639-t1128-t2181+dq5.*t13.*(t86-t652)).*2.840000000000012e-3+t2832.*(t639-t1128-t2181+dq5.*t13.*(t86-t652)).*4.466636216449161e-20;
et1131 = t2974.*(t92-t663).*4.466636216449161e-20+t3422.*(t653-t838).*4.466636216449161e-20;
et1132 = t573.*t843+t12.*t2351-t12.*t2372+t831.*t1770-t1748.*(t88-t617)-t11.*t36.*t1069;
et1133 = (t2341+t2445.*4.988e-2-t2463-t2612+t2624-t2796+t2813+t2900+t1066.*(t86-t652).*1.11e-3).*(-1.0./2.0);
et1134 = -t2711+t2801-t2954+t2956-t3179+t3181+t2165.*(t92-t663).*4.466636216449161e-20+t2816.*(t88-t617).*1.0e-5;
et1135 = t2828.*(t653-t838).*4.466636216449161e-20;
et1136 = t2687.*(t614+t13.*(t86-t652))+t634.*t2196-t1041.*t2816-t1893.*(t92-t663)+t2832.*(t643-t662)+t2722.*(t653-t838);
et1137 = (-t2447-t2783-t2839+t2841+t3126+t3143+t3232+t2165.*(t92-t663).*1.2e-4+t2828.*(t653-t838).*1.2e-4).*(-1.0./2.0);
et1138 = t3668.*(t572.*t1066.*2.0+t604.*t1040.*2.0-dq2.*t3.*t10.*t28.*2.0-dq3.*t4.*t11.*t27.*2.0).*(-1.0./2.0)+(t3818.*(-t1729.*(t878-t1582+t2184+t7.*(t639-t1128-t2181+dq5.*t13.*(t86-t652)))+(t1386+t7.*(t88-t617)).*(t776+t1093-t2737+t14.*(t708-t1079))+t1207.*t2584-t2074.*(t696+t1094-t2697+t14.*(t637-t1126))+t1778.*(t1487+t2219-t2864+dq6.*t7.*(t88-t617))+(t254-t729).*(t642+t896-t1137-t2220)))./2.0;
et1139 = ((t8.*(t92-t663)+t15.*(t621-t864)).*(t806+t1015-t1917+t2670)+t2376.*t3620+t2383.*t3617+t1655.*(t958-t2263+dq7.*t1601+t15.*(t642+t896-t1137-t2220))+t2576.*(t1059+t1889-t2744-t3193)+t2627.*(t1060+t1859-t2729+t8.*(-t694+t777+t1161+t1215+t2699))).*(et717+et718).*(-1.0./2.0)+t3833.*(et719+et720).*3.5432e-1+(t3839.*(et721+et722+et723+et724+et725))./2.0+(t3272.*(et726+et727+et728+et729+et730+et731+et732+et733+et734+et735+et736))./2.0-((t3031+t2165.*(t92-t663)+t2828.*(t653-t838)).*(et737+et738+et739+et740+et741+et742+et743+et744+et745))./2.0;
et1140 = ((t2654.*(-t689+t704+t1159+t1212-t2700)+t1729.*t3619+t1778.*t3618-t2601.*t3165+t3336.*(t254-t729)-(t1529+t15.*(t92-t663)).*(t295+t297+t298-t331-t760-t1953)).*(et746+et747))./2.0+(t2533.*(et748+et749+et750+et751+et752))./2.0-(t3788.*(t678.*t1070+t573.*t1863-t1023.*t2147+t1022.*t2163+t831.*t2707-t2723.*(t88-t617)))./2.0+(t3192.*(et753+et754+et755+et756+et757+et758+et759+et760+et761+et762+et763))./2.0+(t3843.*(t1778.*t2601+t1729.*t2654+(t1529+t15.*(t92-t663)).*(t254-t729)))./2.0;
et1141 = t3820.*(t2832.*(t650+t7.*(t643-t662))+t898.*t2196-t2000.*t2721-t2035.*t2714-t1830.*(t621-t864)+t2816.*(t735-t1077)).*(-1.0./2.0)+et764.*et765+(et766+et767).*(et768+et769).*3.5432e-1-t3776.*(et770+et771).*3.38795+(((t614+t13.*(t86-t652)).*(-t689+t704+t1159+t1212-t2700)-(t92-t663).*(t295+t297+t298-t331-t760-t1953)+t1729.*t2832+t1778.*t2816+t2196.*(t254-t729)-t3165.*(t653-t838)).*(et772+et773))./2.0;
et1142 = ((-t3113+t3418+t2654.*(t884+t1578-t2180+t14.*(t639-t1128-t2181+dq5.*t13.*(t86-t652)))).*(et774+et775+et776+et777+et778+et779+et780+et781+et782))./2.0-((-t3113+t3418+t2654.*(t884+t1578-t2180+t14.*(t639-t1128-t2181+dq5.*t13.*(t86-t652)))).*(et783+et784+et785+et786+et787+et788+et789+et790+et791))./2.0-(t2943.*(et792+et793+et794))./2.0;
et1143 = t3671.*(t1603+t1672+t1682+t1707+t1721+t1799.*5.000000000000001e-5+t1801.*2.37e-3+t2001+t2022+t2026).*(-3.41e+2./1.0e+2);
et1144 = t3670.*(t1636+t1638+t1675+t1711+t1769+t1800.*5.000000000000001e-5+t1804.*2.37e-3+t2002+t2041+t2130).*(3.41e+2./1.0e+2)-(t3842.*(t1022.*t2000+t1023.*t2035+t678.*(t621-t864)))./2.0-(t3610.*(et795+et796+et797+et798+et799+et800+et801+et802+et803+et804))./2.0;
et1145 = ((t2601.*(t813+t1088+t2739+t7.*(t708-t1079))+t2376.*(t884+t1578-t2180+t14.*(t639-t1128-t2181+dq5.*t13.*(t86-t652)))-t2585.*(t1529+t15.*(t92-t663))+t2383.*t3312-t2654.*t3133+t1655.*(t631-t885+t1132-t2224)).*(et805+et806))./2.0+et807.*et808-(t3060.*(et809+et810+et811+et812+et813+et814+et815+et816))./2.0+et817.*et818+((t859-t1791+t1066.*(t86-t652)).*(et819+et820+et821+et822+et823+et824+et825+et826))./2.0-(t3060.*(et827+et828+et829+et830+et831+et832+et833+et834+et835+et836+et837))./2.0-((t2370-t2949+t2816.*(t88-t617)).*(et838+et839+et840+et841+et842+et843+et844+et845+et846+et847+et848))./2.0-(t3789.*(et849+et850+et851+et852+et853+et854+et855+et856+et857))./2.0;
et1146 = (t3789.*(et858+et859+et860+et861+et862+et863+et864+et865+et866))./2.0+(t1866.*(et867+et868+et869+et870+et871))./2.0+((-t2961+t3358+t3312.*(t653-t838)).*(et872+et873+et874+et875+et876+et877+et878+et879+et880+et881))./2.0+(t3783.*(et882+et883+et884+et885+et886))./2.0+(t3829.*(et887+et888+et889+et890+et891))./2.0-t3674.*(et892+et893+et894).*3.38795-(((t614+t13.*(t86-t652)).*(t643-t662)+t634.*(t92-t663)-t1041.*(t653-t838)).*(et895+et896+et897))./2.0;
et1147 = t3252.*(t4.*t10.*3.492e-2+t10.*t11.*2.25e-3).*2.4552+t3798.*(et898+et899+et900).*3.5432e-1+t3796.*(et901+et902).*3.5432e-1+((t3031+t2165.*(t92-t663)+t2828.*(t653-t838)).*(et903+et904+et905+et906+et907+et908+et909+et910))./2.0+t3821.*(et911+et912).*3.5432e-1;
et1148 = ((t1023.*(t884+t1578-t2180+t14.*(t639-t1128-t2181+dq5.*t13.*(t86-t652)))-t3133.*(t614+t13.*(t86-t652))+(t653-t838).*(t813+t1088+t2739+t7.*(t708-t1079))+t1022.*t3312-t2585.*(t92-t663)+t678.*(t631-t885+t1132-t2224)).*(et913+et914))./2.0+(t3828.*(et915+et916+et917+et918+et919))./2.0+((t3377+t2074.*(t878-t1582+t2184+t7.*(t639-t1128-t2181+dq5.*t13.*(t86-t652)))+t1207.*(t642+t896-t1137-t2220)).*(et920+et921+et922+et923+et924+et925+et926+et927+et928+et929))./2.0;
et1149 = t3679.*(t4.*t10.*(-3.818e-2)+t11.*t34.*2.0e-4+t11.*t36.*5.267999999999999e-2).*2.61155+((t2370-t2949+t2816.*(t88-t617)).*(et930+et931+et932+et933+et934+et935+et936+et937+et938))./2.0-(t3811.*(t608+t635+t27.*t28))./2.0+(t3667.*(t1072+t1214+t3.*t602))./2.0;
et1150 = t3781.*(t35.*3.818e-2-t73.*3.818e-2+t5.*t572.*2.0e-4+t12.*t572.*5.267999999999999e-2).*2.61155;
et1151 = t3780.*(t31.*3.818e-2+t77.*3.818e-2+t5.*t604.*2.0e-4+t12.*t604.*5.267999999999999e-2).*(-2.61155);
et1152 = t3812.*(t3.*t4.*t10-t9.*t10.*t571+t2.*t10.*t605).*(-1.0./2.0)-t3796.*(et939+et940).*3.5432e-1+((t2407+t2563+t3085-t3092-t3122+t2147.*(t639-t1128-t2181+dq5.*t13.*(t86-t652))).*(et941+et942+et943+et944+et945))./2.0+et946.*et947+t3628.*(et948+et949).*(3.41e+2./1.0e+2)-(t3669.*(-t567.*t604+t572.*t601+dq2.*t11.*t27))./2.0-(t3788.*(-t573.*t1830-t831.*t2714+t2721.*(t88-t617)+t11.*t36.*t2196+t12.*t572.*t2832+t12.*t604.*t2816))./2.0;
et1153 = ((t3140+t3489+t3720+t2832.*(t884+t1578-t2180+t14.*(t639-t1128-t2181+dq5.*t13.*(t86-t652)))+t3436.*(t92-t663)+t3685.*(t653-t838)).*(et950+et951+et952+et953+et954))./2.0+(t3192.*(et955+et956+et957+et958+et959+et960+et961+et962))./2.0-(t3610.*(et963+et964+et965+et966+et967+et968+et969+et970+et971))./2.0+(t3841.*(t1729.*(t614+t13.*(t86-t652))+t1778.*(t653-t838)+(t92-t663).*(t254-t729)))./2.0+(t3824.*(t12.*t608+t12.*t635+t12.*t27.*t28))./2.0+(t3666.*(et972+et973+et974+et975+et976))./2.0+((t859-t1791+t1066.*(t86-t652)).*(et977+et978+et979+et980+et981+et982+et983+et984+et985+et986+et987))./2.0;
et1154 = ((-t2961+t3358+t3312.*(t653-t838)).*(et988+et989+et990+et991+et992+et993+et994+et995+et996))./2.0+((t2817+t3324+t3433.*(t614+t13.*(t86-t652))+t2832.*(t639-t1128-t2181+dq5.*t13.*(t86-t652))+t2974.*(t92-t663)+t3422.*(t653-t838)).*(et997+et998+et999+et1000))./2.0+t3790.*(et1001+et1002).*3.38795-(t2384.*(et1003+et1004+et1005+et1006+et1007))./2.0;
et1155 = t3628.*(t891.*5.000000000000001e-5+t902.*2.37e-3+t1175+t1178+t1179+t1189+t1190+t1286+t1339+t1368+t1369+t1456+t1569).*(-3.41e+2./1.0e+2)-(et1008+et1009).*(t221.*(2.1e+1./5.0e+1)+t223.*(2.1e+1./5.0e+1)-t542+t547+t548-t554+t580+t581+t583+t800+t1424+t1726+t1856+t1898+t1934+t2042+t2198+t2231+t2253+t2558+t2581+t2587+t2602+t2991+t2997+t3066+t3075+t3082+t3495+t3498).*3.38795-(t3826.*(t11.*t34.*t573-t5.*t572.*t831+t5.*t604.*(t88-t617)))./2.0;
et1156 = (t3377+t2074.*(t878-t1582+t2184+t7.*(t639-t1128-t2181+dq5.*t13.*(t86-t652)))+t1207.*(t642+t896-t1137-t2220)).*(et1010+et1011+et1012+et1013+et1014+et1015+et1016+et1017+et1018).*(-1.0./2.0)-((t3502+t3544-t3547+t2972.*(t621-t864)+t2196.*(t642+t896-t1137-t2220)+t2816.*(t1487+t2219-t2864+dq6.*t7.*(t88-t617))).*(et1019+et1020+et1021+et1022+et1023))./2.0-((t2382.*(t884+t1578-t2180+t14.*(t639-t1128-t2181+dq5.*t13.*(t86-t652)))-t3506.*(t1386+t7.*(t88-t617))+t1207.*t3097+t2074.*t3486+t2392.*t3312+t1686.*(t631-t885+t1132-t2224)).*(et1024+et1025))./2.0;
C = ft_10({dq5,dq6,dq7,et1026,et1027,et1028,et1029,et1030,et1031,et1032,et1033,et1034,et1035,et1036,et1037,et1038,et1039,et1040,et1041,et1042,et1043,et1044,et1045,et1046,et1047,et1048,et1049,et1050,et1051,et1052,et1053,et1054,et1055,et1056,et1057,et1058,et1059,et1060,et1061,et1062,et1063,et1064,et1065,et1066,et1067,et1068,et1069,et1070,et1071,et1072,et1073,et1074,et1075,et1076,et1077,et1078,et1079,et1080,et1081,et1082,et1083,et1084,et1085,et1086,et1087,et1088,et1089,et1090,et1091,et1092,et1093,et1094,et1095,et1096,et1097,et1098,et1099,et1100,et1101,et1102,et1103,et1104,et1105,et1106,et1107,et1108,et1109,et1110,et1111,et1112,et1113,et1114,et1115,et1116,et1117,et1118,et1119,et1120,et1121,et1122,et1123,et1124,et1125,et1126,et1127,et1128,et1129,et1130,et1131,et1132,et1133,et1134,et1135,et1136,et1137,et1138,et1139,et1140,et1141,et1142,et1143,et1144,et1145,et1146,et1147,et1148,et1149,et1150,et1151,et1152,et1153,et1154,et1155,et1156,et217,et218,et219,et220,et221,et222,et223,et224,et225,et226,et227,et228,et229,et685,et686,et687,et688,et689,et690,et691,et692,et693,et694,et695,et696,et697,et698,et699,et700,et701,et702,et703,et704,et705,et706,et707,et708,et709,et710,et711,et712,et713,et714,et715,et716,t10,t1001,t1016,t1017,t1018,t1020,t1022,t1023,t1024,t1040,t1041,t1053,t1056,t1066,t1067,t1069,t1070,t1072,t1077,t1079,t1096,t1097,t11,t1110,t1113,t1123,t1126,t1128,t1130,t1132,t1136,t1137,t1161,t12,t1206,t1207,t1209,t1211,t1213,t1214,t1215,t1218,t1219,t1220,t1226,t1269,t1295,t13,t1329,t1374,t1375,t1386,t1387,t14,t1424,t1462,t1487,t1489,t15,t1515,t1516,t152,t1526,t1528,t1529,t1574,t1578,t1579,t1581,t1582,t160,t1601,t1603,t1604,t1616,t1622,t1625,t1633,t1635,t1636,t1638,t1644,t165,t1655,t1657,t1658,t1660,t1661,t1662,t1667,t1668,t1672,t1675,t1682,t1686,t1687,t1697,t1700,t1702,t1707,t1710,t1711,t1718,t1720,t1721,t1726,t1729,t1734,t1738,t1749,t1760,t1769,t1772,t1776,t1778,t1779,t1791,t1792,t1795,t1798,t1802,t1805,t1806,t1811,t1812,t1839,t1843,t1846,t1853,t1856,t1861,t1863,t1866,t1867,t1872,t1875,t1881,t1886,t1888,t1890,t1898,t1902,t1908,t1924,t1927,t1928,t1931,t1932,t1934,t1940,t1942,t1957,t1959,t1960,t1962,t1963,t1976,t1993,t2000,t2001,t2002,t2006,t2022,t2026,t2035,t2041,t2042,t2044,t2046,t2056,t2058,t2065,t2072,t2073,t2074,t208,t2080,t2081,t2085,t2108,t2109,t2111,t2119,t2125,t2130,t2139,t2147,t2148,t2163,t2164,t2165,t2171,t2173,t2179,t2180,t2181,t2182,t2183,t2184,t2187,t2196,t2198,t2203,t2205,t2206,t2207,t2208,t221,t2212,t2215,t2217,t2219,t2220,t2224,t2227,t2228,t223,t2231,t2240,t2246,t2253,t2256,t2258,t2259,t2261,t2262,t2263,t2264,t2266,t2269,t2289,t230,t2300,t2301,t2315,t2330,t2341,t235,t2352,t2357,t2359,t236,t2360,t2363,t2365,t237,t2370,t2372,t2374,t2375,t2376,t2379,t238,t2380,t2382,t2383,t2384,t2388,t239,t2392,t2407,t2444,t2445,t2447,t2455,t2456,t2460,t2462,t2463,t2466,t2467,t2477,t2482,t2483,t2488,t2496,t2501,t2503,t2507,t2513,t2514,t2516,t2521,t2522,t2523,t2533,t2536,t2537,t254,t2541,t2554,t2558,t2560,t2561,t2563,t2569,t2570,t2571,t2576,t2581,t2587,t2590,t2591,t2601,t2602,t2604,t2611,t2612,t2614,t2617,t2618,t2620,t2621,t2624,t2627,t2634,t2637,t2647,t2648,t2651,t2653,t2654,t2655,t2656,t2663,t2674,t2675,t268,t2693,t2699,t2707,t2710,t2711,t2723,t2732,t2734,t2735,t2747,t2751,t2753,t2754,t2765,t2781,t2783,t2788,t2789,t2790,t2792,t2795,t2796,t2797,t2798,t2799,t2801,t2803,t2804,t2807,t2810,t2811,t2813,t2814,t2816,t2817,t2818,t2823,t2825,t2828,t2829,t2832,t2837,t2838,t2839,t2840,t2841,t2842,t2844,t2857,t2861,t2864,t2868,t2883,t2884,t2891,t29,t2900,t2907,t2914,t2922,t2923,t2925,t2930,t2931,t2935,t2936,t2939,t2941,t2942,t2945,t2946,t2948,t2949,t2950,t2953,t2954,t2955,t2956,t2957,t2960,t2961,t2962,t2972,t2974,t2989,t2991,t2996,t2997,t2998,t30,t3008,t3009,t3011,t3020,t3031,t3035,t3038,t3039,t3040,t3041,t3042,t3045,t3047,t3048,t3051,t3052,t3060,t3066,t3067,t3071,t3075,t3076,t3082,t3083,t3085,t3086,t3088,t3092,t31,t3112,t3113,t3122,t3126,t3130,t3131,t3132,t3140,t3141,t3142,t3143,t3152,t3153,t3154,t3155,t3159,t3161,t3162,t3163,t3166,t3168,t3170,t3171,t3172,t3175,t3179,t3181,t3190,t3192,t3195,t3196,t32,t3201,t3202,t3203,t3204,t3215,t3226,t3229,t3232,t3235,t3238,t3246,t3253,t3255,t3257,t3260,t3261,t3262,t3263,t3264,t3268,t3269,t3272,t3273,t3277,t3279,t3280,t3284,t3288,t3289,t3290,t3291,t3292,t3293,t3294,t3295,t3296,t33,t3301,t3311,t3312,t3315,t3316,t3321,t3324,t3336,t3340,t3356,t3357,t3358,t3359,t3360,t3361,t3362,t3363,t3364,t3365,t3366,t3369,t3372,t3375,t3377,t3382,t3384,t3386,t3388,t3392,t3395,t3397,t3398,t3400,t3402,t3403,t3406,t3407,t3411,t3413,t3414,t3417,t3418,t3421,t3422,t3424,t3426,t3429,t3433,t3436,t3437,t3444,t3452,t3479,t3480,t3481,t3482,t3483,t3488,t3489,t349,t3490,t3491,t3492,t3495,t3498,t35,t3502,t3504,t3514,t3526,t3527,t3528,t3535,t3536,t3537,t3538,t3540,t3542,t3544,t3546,t3547,t3551,t3555,t3556,t3559,t3561,t36,t3610,t3617,t3618,t3619,t3620,t3625,t3626,t3627,t3642,t3643,t3644,t3645,t3646,t3648,t3649,t3651,t3652,t3653,t3654,t3655,t3658,t3660,t3661,t3662,t3663,t3664,t3665,t3666,t3667,t3668,t3670,t3671,t3672,t3673,t3674,t3679,t3685,t3720,t3751,t3776,t3779,t3780,t3781,t3782,t3783,t3784,t3786,t3788,t3789,t3790,t3796,t3798,t3818,t3820,t3821,t3823,t3824,t3825,t3826,t3828,t3829,t3833,t3835,t3838,t3839,t3840,t3841,t3842,t3843,t3844,t3845,t39,t4,t431,t433,t436,t448,t45,t452,t456,t457,t460,t461,t463,t50,t51,t512,t515,t516,t517,t518,t522,t523,t527,t537,t542,t547,t548,t554,t569,t57,t571,t572,t573,t58,t580,t581,t583,t6,t602,t604,t605,t606,t609,t61,t612,t614,t616,t617,t619,t621,t629,t631,t634,t637,t639,t640,t642,t643,t644,t648,t649,t650,t651,t652,t653,t656,t657,t660,t661,t662,t663,t664,t673,t678,t685,t69,t691,t692,t693,t694,t697,t698,t7,t70,t703,t705,t708,t71,t721,t729,t73,t735,t754,t76,t77,t773,t777,t778,t79,t796,t797,t8,t800,t815,t819,t82,t827,t831,t835,t836,t838,t839,t846,t847,t85,t853,t859,t86,t860,t863,t864,t866,t870,t871,t876,t877,t878,t88,t881,t882,t884,t885,t89,t896,t898,t907,t908,t911,t92,t921,t926,t927,t928,t930,t932,t933,t935,t939,t942,t948,t949,t952,t958,t966,t969,t982,t983,t984,t987,t988,t992,t994});
end
function C = ft_10(ct)
dq5 = ct{1};
dq6 = ct{2};
dq7 = ct{3};
et1026 = ct{4};
et1027 = ct{5};
et1028 = ct{6};
et1029 = ct{7};
et1030 = ct{8};
et1031 = ct{9};
et1032 = ct{10};
et1033 = ct{11};
et1034 = ct{12};
et1035 = ct{13};
et1036 = ct{14};
et1037 = ct{15};
et1038 = ct{16};
et1039 = ct{17};
et1040 = ct{18};
et1041 = ct{19};
et1042 = ct{20};
et1043 = ct{21};
et1044 = ct{22};
et1045 = ct{23};
et1046 = ct{24};
et1047 = ct{25};
et1048 = ct{26};
et1049 = ct{27};
et1050 = ct{28};
et1051 = ct{29};
et1052 = ct{30};
et1053 = ct{31};
et1054 = ct{32};
et1055 = ct{33};
et1056 = ct{34};
et1057 = ct{35};
et1058 = ct{36};
et1059 = ct{37};
et1060 = ct{38};
et1061 = ct{39};
et1062 = ct{40};
et1063 = ct{41};
et1064 = ct{42};
et1065 = ct{43};
et1066 = ct{44};
et1067 = ct{45};
et1068 = ct{46};
et1069 = ct{47};
et1070 = ct{48};
et1071 = ct{49};
et1072 = ct{50};
et1073 = ct{51};
et1074 = ct{52};
et1075 = ct{53};
et1076 = ct{54};
et1077 = ct{55};
et1078 = ct{56};
et1079 = ct{57};
et1080 = ct{58};
et1081 = ct{59};
et1082 = ct{60};
et1083 = ct{61};
et1084 = ct{62};
et1085 = ct{63};
et1086 = ct{64};
et1087 = ct{65};
et1088 = ct{66};
et1089 = ct{67};
et1090 = ct{68};
et1091 = ct{69};
et1092 = ct{70};
et1093 = ct{71};
et1094 = ct{72};
et1095 = ct{73};
et1096 = ct{74};
et1097 = ct{75};
et1098 = ct{76};
et1099 = ct{77};
et1100 = ct{78};
et1101 = ct{79};
et1102 = ct{80};
et1103 = ct{81};
et1104 = ct{82};
et1105 = ct{83};
et1106 = ct{84};
et1107 = ct{85};
et1108 = ct{86};
et1109 = ct{87};
et1110 = ct{88};
et1111 = ct{89};
et1112 = ct{90};
et1113 = ct{91};
et1114 = ct{92};
et1115 = ct{93};
et1116 = ct{94};
et1117 = ct{95};
et1118 = ct{96};
et1119 = ct{97};
et1120 = ct{98};
et1121 = ct{99};
et1122 = ct{100};
et1123 = ct{101};
et1124 = ct{102};
et1125 = ct{103};
et1126 = ct{104};
et1127 = ct{105};
et1128 = ct{106};
et1129 = ct{107};
et1130 = ct{108};
et1131 = ct{109};
et1132 = ct{110};
et1133 = ct{111};
et1134 = ct{112};
et1135 = ct{113};
et1136 = ct{114};
et1137 = ct{115};
et1138 = ct{116};
et1139 = ct{117};
et1140 = ct{118};
et1141 = ct{119};
et1142 = ct{120};
et1143 = ct{121};
et1144 = ct{122};
et1145 = ct{123};
et1146 = ct{124};
et1147 = ct{125};
et1148 = ct{126};
et1149 = ct{127};
et1150 = ct{128};
et1151 = ct{129};
et1152 = ct{130};
et1153 = ct{131};
et1154 = ct{132};
et1155 = ct{133};
et1156 = ct{134};
et217 = ct{135};
et218 = ct{136};
et219 = ct{137};
et220 = ct{138};
et221 = ct{139};
et222 = ct{140};
et223 = ct{141};
et224 = ct{142};
et225 = ct{143};
et226 = ct{144};
et227 = ct{145};
et228 = ct{146};
et229 = ct{147};
et685 = ct{148};
et686 = ct{149};
et687 = ct{150};
et688 = ct{151};
et689 = ct{152};
et690 = ct{153};
et691 = ct{154};
et692 = ct{155};
et693 = ct{156};
et694 = ct{157};
et695 = ct{158};
et696 = ct{159};
et697 = ct{160};
et698 = ct{161};
et699 = ct{162};
et700 = ct{163};
et701 = ct{164};
et702 = ct{165};
et703 = ct{166};
et704 = ct{167};
et705 = ct{168};
et706 = ct{169};
et707 = ct{170};
et708 = ct{171};
et709 = ct{172};
et710 = ct{173};
et711 = ct{174};
et712 = ct{175};
et713 = ct{176};
et714 = ct{177};
et715 = ct{178};
et716 = ct{179};
t10 = ct{180};
t1001 = ct{181};
t1016 = ct{182};
t1017 = ct{183};
t1018 = ct{184};
t1020 = ct{185};
t1022 = ct{186};
t1023 = ct{187};
t1024 = ct{188};
t1040 = ct{189};
t1041 = ct{190};
t1053 = ct{191};
t1056 = ct{192};
t1066 = ct{193};
t1067 = ct{194};
t1069 = ct{195};
t1070 = ct{196};
t1072 = ct{197};
t1077 = ct{198};
t1079 = ct{199};
t1096 = ct{200};
t1097 = ct{201};
t11 = ct{202};
t1110 = ct{203};
t1113 = ct{204};
t1123 = ct{205};
t1126 = ct{206};
t1128 = ct{207};
t1130 = ct{208};
t1132 = ct{209};
t1136 = ct{210};
t1137 = ct{211};
t1161 = ct{212};
t12 = ct{213};
t1206 = ct{214};
t1207 = ct{215};
t1209 = ct{216};
t1211 = ct{217};
t1213 = ct{218};
t1214 = ct{219};
t1215 = ct{220};
t1218 = ct{221};
t1219 = ct{222};
t1220 = ct{223};
t1226 = ct{224};
t1269 = ct{225};
t1295 = ct{226};
t13 = ct{227};
t1329 = ct{228};
t1374 = ct{229};
t1375 = ct{230};
t1386 = ct{231};
t1387 = ct{232};
t14 = ct{233};
t1424 = ct{234};
t1462 = ct{235};
t1487 = ct{236};
t1489 = ct{237};
t15 = ct{238};
t1515 = ct{239};
t1516 = ct{240};
t152 = ct{241};
t1526 = ct{242};
t1528 = ct{243};
t1529 = ct{244};
t1574 = ct{245};
t1578 = ct{246};
t1579 = ct{247};
t1581 = ct{248};
t1582 = ct{249};
t160 = ct{250};
t1601 = ct{251};
t1603 = ct{252};
t1604 = ct{253};
t1616 = ct{254};
t1622 = ct{255};
t1625 = ct{256};
t1633 = ct{257};
t1635 = ct{258};
t1636 = ct{259};
t1638 = ct{260};
t1644 = ct{261};
t165 = ct{262};
t1655 = ct{263};
t1657 = ct{264};
t1658 = ct{265};
t1660 = ct{266};
t1661 = ct{267};
t1662 = ct{268};
t1667 = ct{269};
t1668 = ct{270};
t1672 = ct{271};
t1675 = ct{272};
t1682 = ct{273};
t1686 = ct{274};
t1687 = ct{275};
t1697 = ct{276};
t1700 = ct{277};
t1702 = ct{278};
t1707 = ct{279};
t1710 = ct{280};
t1711 = ct{281};
t1718 = ct{282};
t1720 = ct{283};
t1721 = ct{284};
t1726 = ct{285};
t1729 = ct{286};
t1734 = ct{287};
t1738 = ct{288};
t1749 = ct{289};
t1760 = ct{290};
t1769 = ct{291};
t1772 = ct{292};
t1776 = ct{293};
t1778 = ct{294};
t1779 = ct{295};
t1791 = ct{296};
t1792 = ct{297};
t1795 = ct{298};
t1798 = ct{299};
t1802 = ct{300};
t1805 = ct{301};
t1806 = ct{302};
t1811 = ct{303};
t1812 = ct{304};
t1839 = ct{305};
t1843 = ct{306};
t1846 = ct{307};
t1853 = ct{308};
t1856 = ct{309};
t1861 = ct{310};
t1863 = ct{311};
t1866 = ct{312};
t1867 = ct{313};
t1872 = ct{314};
t1875 = ct{315};
t1881 = ct{316};
t1886 = ct{317};
t1888 = ct{318};
t1890 = ct{319};
t1898 = ct{320};
t1902 = ct{321};
t1908 = ct{322};
t1924 = ct{323};
t1927 = ct{324};
t1928 = ct{325};
t1931 = ct{326};
t1932 = ct{327};
t1934 = ct{328};
t1940 = ct{329};
t1942 = ct{330};
t1957 = ct{331};
t1959 = ct{332};
t1960 = ct{333};
t1962 = ct{334};
t1963 = ct{335};
t1976 = ct{336};
t1993 = ct{337};
t2000 = ct{338};
t2001 = ct{339};
t2002 = ct{340};
t2006 = ct{341};
t2022 = ct{342};
t2026 = ct{343};
t2035 = ct{344};
t2041 = ct{345};
t2042 = ct{346};
t2044 = ct{347};
t2046 = ct{348};
t2056 = ct{349};
t2058 = ct{350};
t2065 = ct{351};
t2072 = ct{352};
t2073 = ct{353};
t2074 = ct{354};
t208 = ct{355};
t2080 = ct{356};
t2081 = ct{357};
t2085 = ct{358};
t2108 = ct{359};
t2109 = ct{360};
t2111 = ct{361};
t2119 = ct{362};
t2125 = ct{363};
t2130 = ct{364};
t2139 = ct{365};
t2147 = ct{366};
t2148 = ct{367};
t2163 = ct{368};
t2164 = ct{369};
t2165 = ct{370};
t2171 = ct{371};
t2173 = ct{372};
t2179 = ct{373};
t2180 = ct{374};
t2181 = ct{375};
t2182 = ct{376};
t2183 = ct{377};
t2184 = ct{378};
t2187 = ct{379};
t2196 = ct{380};
t2198 = ct{381};
t2203 = ct{382};
t2205 = ct{383};
t2206 = ct{384};
t2207 = ct{385};
t2208 = ct{386};
t221 = ct{387};
t2212 = ct{388};
t2215 = ct{389};
t2217 = ct{390};
t2219 = ct{391};
t2220 = ct{392};
t2224 = ct{393};
t2227 = ct{394};
t2228 = ct{395};
t223 = ct{396};
t2231 = ct{397};
t2240 = ct{398};
t2246 = ct{399};
t2253 = ct{400};
t2256 = ct{401};
t2258 = ct{402};
t2259 = ct{403};
t2261 = ct{404};
t2262 = ct{405};
t2263 = ct{406};
t2264 = ct{407};
t2266 = ct{408};
t2269 = ct{409};
t2289 = ct{410};
t230 = ct{411};
t2300 = ct{412};
t2301 = ct{413};
t2315 = ct{414};
t2330 = ct{415};
t2341 = ct{416};
t235 = ct{417};
t2352 = ct{418};
t2357 = ct{419};
t2359 = ct{420};
t236 = ct{421};
t2360 = ct{422};
t2363 = ct{423};
t2365 = ct{424};
t237 = ct{425};
t2370 = ct{426};
t2372 = ct{427};
t2374 = ct{428};
t2375 = ct{429};
t2376 = ct{430};
t2379 = ct{431};
t238 = ct{432};
t2380 = ct{433};
t2382 = ct{434};
t2383 = ct{435};
t2384 = ct{436};
t2388 = ct{437};
t239 = ct{438};
t2392 = ct{439};
t2407 = ct{440};
t2444 = ct{441};
t2445 = ct{442};
t2447 = ct{443};
t2455 = ct{444};
t2456 = ct{445};
t2460 = ct{446};
t2462 = ct{447};
t2463 = ct{448};
t2466 = ct{449};
t2467 = ct{450};
t2477 = ct{451};
t2482 = ct{452};
t2483 = ct{453};
t2488 = ct{454};
t2496 = ct{455};
t2501 = ct{456};
t2503 = ct{457};
t2507 = ct{458};
t2513 = ct{459};
t2514 = ct{460};
t2516 = ct{461};
t2521 = ct{462};
t2522 = ct{463};
t2523 = ct{464};
t2533 = ct{465};
t2536 = ct{466};
t2537 = ct{467};
t254 = ct{468};
t2541 = ct{469};
t2554 = ct{470};
t2558 = ct{471};
t2560 = ct{472};
t2561 = ct{473};
t2563 = ct{474};
t2569 = ct{475};
t2570 = ct{476};
t2571 = ct{477};
t2576 = ct{478};
t2581 = ct{479};
t2587 = ct{480};
t2590 = ct{481};
t2591 = ct{482};
t2601 = ct{483};
t2602 = ct{484};
t2604 = ct{485};
t2611 = ct{486};
t2612 = ct{487};
t2614 = ct{488};
t2617 = ct{489};
t2618 = ct{490};
t2620 = ct{491};
t2621 = ct{492};
t2624 = ct{493};
t2627 = ct{494};
t2634 = ct{495};
t2637 = ct{496};
t2647 = ct{497};
t2648 = ct{498};
t2651 = ct{499};
t2653 = ct{500};
t2654 = ct{501};
t2655 = ct{502};
t2656 = ct{503};
t2663 = ct{504};
t2674 = ct{505};
t2675 = ct{506};
t268 = ct{507};
t2693 = ct{508};
t2699 = ct{509};
t2707 = ct{510};
t2710 = ct{511};
t2711 = ct{512};
t2723 = ct{513};
t2732 = ct{514};
t2734 = ct{515};
t2735 = ct{516};
t2747 = ct{517};
t2751 = ct{518};
t2753 = ct{519};
t2754 = ct{520};
t2765 = ct{521};
t2781 = ct{522};
t2783 = ct{523};
t2788 = ct{524};
t2789 = ct{525};
t2790 = ct{526};
t2792 = ct{527};
t2795 = ct{528};
t2796 = ct{529};
t2797 = ct{530};
t2798 = ct{531};
t2799 = ct{532};
t2801 = ct{533};
t2803 = ct{534};
t2804 = ct{535};
t2807 = ct{536};
t2810 = ct{537};
t2811 = ct{538};
t2813 = ct{539};
t2814 = ct{540};
t2816 = ct{541};
t2817 = ct{542};
t2818 = ct{543};
t2823 = ct{544};
t2825 = ct{545};
t2828 = ct{546};
t2829 = ct{547};
t2832 = ct{548};
t2837 = ct{549};
t2838 = ct{550};
t2839 = ct{551};
t2840 = ct{552};
t2841 = ct{553};
t2842 = ct{554};
t2844 = ct{555};
t2857 = ct{556};
t2861 = ct{557};
t2864 = ct{558};
t2868 = ct{559};
t2883 = ct{560};
t2884 = ct{561};
t2891 = ct{562};
t29 = ct{563};
t2900 = ct{564};
t2907 = ct{565};
t2914 = ct{566};
t2922 = ct{567};
t2923 = ct{568};
t2925 = ct{569};
t2930 = ct{570};
t2931 = ct{571};
t2935 = ct{572};
t2936 = ct{573};
t2939 = ct{574};
t2941 = ct{575};
t2942 = ct{576};
t2945 = ct{577};
t2946 = ct{578};
t2948 = ct{579};
t2949 = ct{580};
t2950 = ct{581};
t2953 = ct{582};
t2954 = ct{583};
t2955 = ct{584};
t2956 = ct{585};
t2957 = ct{586};
t2960 = ct{587};
t2961 = ct{588};
t2962 = ct{589};
t2972 = ct{590};
t2974 = ct{591};
t2989 = ct{592};
t2991 = ct{593};
t2996 = ct{594};
t2997 = ct{595};
t2998 = ct{596};
t30 = ct{597};
t3008 = ct{598};
t3009 = ct{599};
t3011 = ct{600};
t3020 = ct{601};
t3031 = ct{602};
t3035 = ct{603};
t3038 = ct{604};
t3039 = ct{605};
t3040 = ct{606};
t3041 = ct{607};
t3042 = ct{608};
t3045 = ct{609};
t3047 = ct{610};
t3048 = ct{611};
t3051 = ct{612};
t3052 = ct{613};
t3060 = ct{614};
t3066 = ct{615};
t3067 = ct{616};
t3071 = ct{617};
t3075 = ct{618};
t3076 = ct{619};
t3082 = ct{620};
t3083 = ct{621};
t3085 = ct{622};
t3086 = ct{623};
t3088 = ct{624};
t3092 = ct{625};
t31 = ct{626};
t3112 = ct{627};
t3113 = ct{628};
t3122 = ct{629};
t3126 = ct{630};
t3130 = ct{631};
t3131 = ct{632};
t3132 = ct{633};
t3140 = ct{634};
t3141 = ct{635};
t3142 = ct{636};
t3143 = ct{637};
t3152 = ct{638};
t3153 = ct{639};
t3154 = ct{640};
t3155 = ct{641};
t3159 = ct{642};
t3161 = ct{643};
t3162 = ct{644};
t3163 = ct{645};
t3166 = ct{646};
t3168 = ct{647};
t3170 = ct{648};
t3171 = ct{649};
t3172 = ct{650};
t3175 = ct{651};
t3179 = ct{652};
t3181 = ct{653};
t3190 = ct{654};
t3192 = ct{655};
t3195 = ct{656};
t3196 = ct{657};
t32 = ct{658};
t3201 = ct{659};
t3202 = ct{660};
t3203 = ct{661};
t3204 = ct{662};
t3215 = ct{663};
t3226 = ct{664};
t3229 = ct{665};
t3232 = ct{666};
t3235 = ct{667};
t3238 = ct{668};
t3246 = ct{669};
t3253 = ct{670};
t3255 = ct{671};
t3257 = ct{672};
t3260 = ct{673};
t3261 = ct{674};
t3262 = ct{675};
t3263 = ct{676};
t3264 = ct{677};
t3268 = ct{678};
t3269 = ct{679};
t3272 = ct{680};
t3273 = ct{681};
t3277 = ct{682};
t3279 = ct{683};
t3280 = ct{684};
t3284 = ct{685};
t3288 = ct{686};
t3289 = ct{687};
t3290 = ct{688};
t3291 = ct{689};
t3292 = ct{690};
t3293 = ct{691};
t3294 = ct{692};
t3295 = ct{693};
t3296 = ct{694};
t33 = ct{695};
t3301 = ct{696};
t3311 = ct{697};
t3312 = ct{698};
t3315 = ct{699};
t3316 = ct{700};
t3321 = ct{701};
t3324 = ct{702};
t3336 = ct{703};
t3340 = ct{704};
t3356 = ct{705};
t3357 = ct{706};
t3358 = ct{707};
t3359 = ct{708};
t3360 = ct{709};
t3361 = ct{710};
t3362 = ct{711};
t3363 = ct{712};
t3364 = ct{713};
t3365 = ct{714};
t3366 = ct{715};
t3369 = ct{716};
t3372 = ct{717};
t3375 = ct{718};
t3377 = ct{719};
t3382 = ct{720};
t3384 = ct{721};
t3386 = ct{722};
t3388 = ct{723};
t3392 = ct{724};
t3395 = ct{725};
t3397 = ct{726};
t3398 = ct{727};
t3400 = ct{728};
t3402 = ct{729};
t3403 = ct{730};
t3406 = ct{731};
t3407 = ct{732};
t3411 = ct{733};
t3413 = ct{734};
t3414 = ct{735};
t3417 = ct{736};
t3418 = ct{737};
t3421 = ct{738};
t3422 = ct{739};
t3424 = ct{740};
t3426 = ct{741};
t3429 = ct{742};
t3433 = ct{743};
t3436 = ct{744};
t3437 = ct{745};
t3444 = ct{746};
t3452 = ct{747};
t3479 = ct{748};
t3480 = ct{749};
t3481 = ct{750};
t3482 = ct{751};
t3483 = ct{752};
t3488 = ct{753};
t3489 = ct{754};
t349 = ct{755};
t3490 = ct{756};
t3491 = ct{757};
t3492 = ct{758};
t3495 = ct{759};
t3498 = ct{760};
t35 = ct{761};
t3502 = ct{762};
t3504 = ct{763};
t3514 = ct{764};
t3526 = ct{765};
t3527 = ct{766};
t3528 = ct{767};
t3535 = ct{768};
t3536 = ct{769};
t3537 = ct{770};
t3538 = ct{771};
t3540 = ct{772};
t3542 = ct{773};
t3544 = ct{774};
t3546 = ct{775};
t3547 = ct{776};
t3551 = ct{777};
t3555 = ct{778};
t3556 = ct{779};
t3559 = ct{780};
t3561 = ct{781};
t36 = ct{782};
t3610 = ct{783};
t3617 = ct{784};
t3618 = ct{785};
t3619 = ct{786};
t3620 = ct{787};
t3625 = ct{788};
t3626 = ct{789};
t3627 = ct{790};
t3642 = ct{791};
t3643 = ct{792};
t3644 = ct{793};
t3645 = ct{794};
t3646 = ct{795};
t3648 = ct{796};
t3649 = ct{797};
t3651 = ct{798};
t3652 = ct{799};
t3653 = ct{800};
t3654 = ct{801};
t3655 = ct{802};
t3658 = ct{803};
t3660 = ct{804};
t3661 = ct{805};
t3662 = ct{806};
t3663 = ct{807};
t3664 = ct{808};
t3665 = ct{809};
t3666 = ct{810};
t3667 = ct{811};
t3668 = ct{812};
t3670 = ct{813};
t3671 = ct{814};
t3672 = ct{815};
t3673 = ct{816};
t3674 = ct{817};
t3679 = ct{818};
t3685 = ct{819};
t3720 = ct{820};
t3751 = ct{821};
t3776 = ct{822};
t3779 = ct{823};
t3780 = ct{824};
t3781 = ct{825};
t3782 = ct{826};
t3783 = ct{827};
t3784 = ct{828};
t3786 = ct{829};
t3788 = ct{830};
t3789 = ct{831};
t3790 = ct{832};
t3796 = ct{833};
t3798 = ct{834};
t3818 = ct{835};
t3820 = ct{836};
t3821 = ct{837};
t3823 = ct{838};
t3824 = ct{839};
t3825 = ct{840};
t3826 = ct{841};
t3828 = ct{842};
t3829 = ct{843};
t3833 = ct{844};
t3835 = ct{845};
t3838 = ct{846};
t3839 = ct{847};
t3840 = ct{848};
t3841 = ct{849};
t3842 = ct{850};
t3843 = ct{851};
t3844 = ct{852};
t3845 = ct{853};
t39 = ct{854};
t4 = ct{855};
t431 = ct{856};
t433 = ct{857};
t436 = ct{858};
t448 = ct{859};
t45 = ct{860};
t452 = ct{861};
t456 = ct{862};
t457 = ct{863};
t460 = ct{864};
t461 = ct{865};
t463 = ct{866};
t50 = ct{867};
t51 = ct{868};
t512 = ct{869};
t515 = ct{870};
t516 = ct{871};
t517 = ct{872};
t518 = ct{873};
t522 = ct{874};
t523 = ct{875};
t527 = ct{876};
t537 = ct{877};
t542 = ct{878};
t547 = ct{879};
t548 = ct{880};
t554 = ct{881};
t569 = ct{882};
t57 = ct{883};
t571 = ct{884};
t572 = ct{885};
t573 = ct{886};
t58 = ct{887};
t580 = ct{888};
t581 = ct{889};
t583 = ct{890};
t6 = ct{891};
t602 = ct{892};
t604 = ct{893};
t605 = ct{894};
t606 = ct{895};
t609 = ct{896};
t61 = ct{897};
t612 = ct{898};
t614 = ct{899};
t616 = ct{900};
t617 = ct{901};
t619 = ct{902};
t621 = ct{903};
t629 = ct{904};
t631 = ct{905};
t634 = ct{906};
t637 = ct{907};
t639 = ct{908};
t640 = ct{909};
t642 = ct{910};
t643 = ct{911};
t644 = ct{912};
t648 = ct{913};
t649 = ct{914};
t650 = ct{915};
t651 = ct{916};
t652 = ct{917};
t653 = ct{918};
t656 = ct{919};
t657 = ct{920};
t660 = ct{921};
t661 = ct{922};
t662 = ct{923};
t663 = ct{924};
t664 = ct{925};
t673 = ct{926};
t678 = ct{927};
t685 = ct{928};
t69 = ct{929};
t691 = ct{930};
t692 = ct{931};
t693 = ct{932};
t694 = ct{933};
t697 = ct{934};
t698 = ct{935};
t7 = ct{936};
t70 = ct{937};
t703 = ct{938};
t705 = ct{939};
t708 = ct{940};
t71 = ct{941};
t721 = ct{942};
t729 = ct{943};
t73 = ct{944};
t735 = ct{945};
t754 = ct{946};
t76 = ct{947};
t77 = ct{948};
t773 = ct{949};
t777 = ct{950};
t778 = ct{951};
t79 = ct{952};
t796 = ct{953};
t797 = ct{954};
t8 = ct{955};
t800 = ct{956};
t815 = ct{957};
t819 = ct{958};
t82 = ct{959};
t827 = ct{960};
t831 = ct{961};
t835 = ct{962};
t836 = ct{963};
t838 = ct{964};
t839 = ct{965};
t846 = ct{966};
t847 = ct{967};
t85 = ct{968};
t853 = ct{969};
t859 = ct{970};
t86 = ct{971};
t860 = ct{972};
t863 = ct{973};
t864 = ct{974};
t866 = ct{975};
t870 = ct{976};
t871 = ct{977};
t876 = ct{978};
t877 = ct{979};
t878 = ct{980};
t88 = ct{981};
t881 = ct{982};
t882 = ct{983};
t884 = ct{984};
t885 = ct{985};
t89 = ct{986};
t896 = ct{987};
t898 = ct{988};
t907 = ct{989};
t908 = ct{990};
t911 = ct{991};
t92 = ct{992};
t921 = ct{993};
t926 = ct{994};
t927 = ct{995};
t928 = ct{996};
t930 = ct{997};
t932 = ct{998};
t933 = ct{999};
t935 = ct{1000};
t939 = ct{1001};
t942 = ct{1002};
t948 = ct{1003};
t949 = ct{1004};
t952 = ct{1005};
t958 = ct{1006};
t966 = ct{1007};
t969 = ct{1008};
t982 = ct{1009};
t983 = ct{1010};
t984 = ct{1011};
t987 = ct{1012};
t988 = ct{1013};
t992 = ct{1014};
t994 = ct{1015};
et1157 = t3818.*(t3166.*(t1386+t7.*(t88-t617))+t1207.*t2634+t3312.*(t735-t1077)-t898.*(t631-t885+t1132-t2224)+t2074.*(-t694+t777+t1161+t1215+t2699)+(t650+t7.*(t643-t662)).*(t884+t1578-t2180+t14.*(t639-t1128-t2181+dq5.*t13.*(t86-t652)))).*(-1.0./2.0);
et1158 = t3671.*(t693.*5.000000000000001e-5+t703.*2.37e-3+t1209.*5.000000000000001e-5+t1211.*2.37e-3+t1603+t1672+t1682+t1707+t1721+t2001+t2022+t2026).*(3.41e+2./1.0e+2);
et1159 = t3670.*(t773.*5.000000000000001e-5+t778.*2.37e-3+t1110.*5.000000000000001e-5+t1113.*2.37e-3+t1636+t1638+t1675+t1711+t1769+t2002+t2041+t2130).*(-3.41e+2./1.0e+2);
et1160 = t3672.*(t32.*2.25e-3-t35.*3.492e-2+t73.*3.492e-2+t76.*2.25e-3).*(-2.4552);
et1161 = t3673.*(t29.*(-2.25e-3)+t31.*3.492e-2+t77.*3.492e-2+t85.*2.25e-3).*2.4552-t3776.*(et1026+et1027).*3.38795;
et1162 = (t3782.*(et1028+et1029+et1030+et1031+et1032+et1033+et1034+et1035+et1036))./2.0-(t3782.*(et1037+et1038+et1039+et1040+et1041+et1042+et1043+et1044+et1045))./2.0-((t3504.*(t1386+t7.*(t88-t617))-t1207.*t3076+t1729.*t3620+t1778.*t3617-t2074.*t3488-(t254-t729).*(t958-t2263+dq7.*t1601+t15.*(t642+t896-t1137-t2220))).*(et1046+et1047))./2.0+et1048.*et1049-(t3272.*(et1050+et1051+et1052+et1053+et1054+et1055+et1056+et1057+et1058))./2.0-(t3825.*(-t571.*t815+t605.*(t86-t652)+t4.*t10.*t606))./2.0+t3835.*(et1059+et1060).*3.5432e-1+(t3838.*(et1061+et1062+et1063+et1064+et1065))./2.0-((t573.*t678+t831.*t1023-t1022.*(t88-t617)).*(et1066+et1067+et1068))./2.0;
et1163 = (et1069+et1070).*(t152.*t827+t160.*t827+t165.*t827+t708.*t1206+t637.*t1295-t1079.*t1206-t1126.*t1295+t12.*t572.*(t639-t1128-t2181+dq5.*t13.*(t86-t652))+t11.*t36.*t2165+t12.*t604.*t2828).*(-1.0./2.0)+t3798.*(et1071+et1072).*3.5432e-1;
et1164 = (et1073+et1074+et1075).*(t436-t448-t452+t460+t537+t796+t1097-t1644-t1875+t1890-t2065+t2205+t2227+t2523-t2537-t2560+t2989+t14.*(t639-t1128-t2181+dq5.*t13.*(t86-t652)).*2.019e-2+dq5.*t6.*(t86-t652).*2.75e-2).*3.38795-(t3364.*(et1076+et1077+et1078))./2.0-(t3546.*(et1079+et1080+et1081+et1082+et1083))./2.0;
et1165 = (et1084+et1085).*(t436-t448-t452+t460+t537+t796+t1097-t1644-t1875+t1890-t2065+t2205+t2227+t2523-t2537-t2560+t2989+t14.*(t639-t1128-t2181+dq5.*t13.*(t86-t652)).*2.019e-2+dq5.*t6.*(t86-t652).*2.75e-2).*(-3.38795);
et1166 = ((t3086.*(t8.*(t92-t663)+t15.*(t621-t864))-t1686.*t3336+t2382.*t3619+t2392.*t3618+t2576.*t3514+t2627.*t3490).*(et1086+et1087))./2.0+(t3668.*(t605.*t1020-t571.*t1067+t572.*t1066+t604.*t1040-t10.*t11.*t569+t4.*t10.*t602))./2.0-t3779.*(et1088+et1089).*(3.41e+2./1.0e+2)+t3786.*(et1090+et1091).*(3.41e+2./1.0e+2)-t3784.*(et1092+et1093).*(3.41e+2./1.0e+2)-(t3372.*(et1094+et1095+et1096))./2.0+(t1866.*(et1097+et1098+et1099+et1100+et1101))./2.0-(et1102+et1103).*(et1104+et1105).*3.5432e-1-(t2384.*(et1106+et1107+et1108+et1109+et1110+et1111))./2.0+t3674.*(et1112+et1113).*3.38795;
et1167 = t3845.*(-t2392.*(t1386+t7.*(t88-t617))+t1207.*t1686+t2074.*t2382).*(-1.0./2.0)+t3823.*(et1114+et1115).*3.38795+((t2056-t2360-t2788-t2807+t3051+t2962.*(t88-t617)).*(et1116+et1117+et1118+et1119+et1120))./2.0-(t3820.*(-t1023.*(t878-t1582+t2184+t7.*(t639-t1128-t2181+dq5.*t13.*(t86-t652)))+t2000.*t2723+t2035.*t2707+t1863.*(t621-t864)-t678.*(t642+t896-t1137-t2220)+t1022.*(t1487+t2219-t2864+dq6.*t7.*(t88-t617))))./2.0+et1121.*et1122+(t2533.*(et1123+et1124+et1125+et1126+et1127+et1128))./2.0;
et1168 = (t3844.*(t1655.*(t8.*(t92-t663)+t15.*(t621-t864))+t2383.*t2576+t2376.*t2627))./2.0+((t11.*t36.*t827+t12.*t604.*t1206+t12.*t572.*t1295).*(et1129+et1130+et1131))./2.0+et1132.*et1133+(t3840.*(-t2074.*(t650+t7.*(t643-t662))+t898.*t1207+(t1386+t7.*(t88-t617)).*(t735-t1077)))./2.0+((t819.*t827+t634.*t1070+t1041.*t2163+t1206.*(t708-t1079)+t1295.*(t637-t1126)+t2147.*(t643-t662)).*(et1134+et1135))./2.0+(t3667.*(t208-t1072-t1214+t10.*t57-t4.*t69+t45.*t571+t50.*t571-t39.*t605+t61.*t605))./2.0+et1136.*et1137;
et1169 = t2315.*(t1386+t7.*(t88-t617)).*2.2e-4+t1207.*t1697.*2.2e-4;
et1170 = t1700.*t2601.*1.089e-2+t1776.*t2654.*1.089e-2;
et1171 = t2289.*t2576.*(-2.9e-4)-t2330.*t2627.*2.9e-4;
et1172 = (t1529+t15.*(t92-t663)).*(t648-t657).*(-1.089e-2)-(t8.*(t92-t663)+t15.*(t621-t864)).*(t651-t1053).*2.9e-4;
et1173 = t2074.*(t908+t15.*(t921+t14.*(t86-t652))).*2.2e-4;
et1174 = t268+t685+t836.*1.9738e-1-t969.*2.324e-2+t1792.*3.466000000000001e-2-t1795.*2.324e-2;
et1175 = t6.*t14.*(t88-t617).*(-1.9738e-1)-t13.*t15.*(t88-t617).*3.466000000000001e-2;
et1176 = t1791.*(-1.12e-3)+t2462-t2797+t2814+t51.*t606.*1.12e-3;
et1177 = t58.*t606.*1.12e-3+t573.*t1070.*9.976e-2;
et1178 = t831.*t2147.*(-9.976e-2)+t1066.*(t86-t652).*1.12e-3;
et1179 = t2163.*(t88-t617).*(-9.976e-2);
et1180 = t2710-t2955+t2957-t882.*(t614+t13.*(t86-t652)).*4.466636216449161e-20+t2179.*(t614+t13.*(t86-t652)).*4.466636216449161e-20;
et1181 = t573.*t1136.*2.0e-5+t6.*t2370.*4.466636216449161e-20;
et1182 = t606.*t2165.*2.840000000000012e-3-t6.*t2949.*4.466636216449161e-20;
et1183 = t831.*t2182.*(-2.0e-5)+t815.*t2828.*2.840000000000012e-3;
et1184 = (t86-t652).*(t639-t1128-t2181+dq5.*t13.*(t86-t652)).*(-2.840000000000012e-3)+t629.*(t92-t663).*4.466636216449161e-20;
et1185 = t1130.*(t92-t663).*4.466636216449161e-20-t2217.*(t88-t617).*2.0e-5;
et1186 = t2212.*(t653-t838).*(-4.466636216449161e-20)-dq5.*t6.*t609.*1.0e-5;
et1187 = dq5.*t6.*t846.*(-1.0e-5)-dq5.*t6.*t847.*1.0e-5;
et1188 = t6.*t2816.*(t88-t617).*4.466636216449161e-20+dq5.*t13.*(t88-t617).*(t653-t838).*4.466636216449161e-20;
et1189 = -t2711+t2801-t2954+t2956-t3179+t3181+t2165.*(t92-t663).*4.466636216449161e-20+t2816.*(t88-t617).*1.0e-5;
et1190 = t2828.*(t653-t838).*4.466636216449161e-20;
et1191 = t2466-t2799+t2811-t569.*t573.*1.144e-2+t573.*t1070.*1.11e-3;
et1192 = t606.*t1069.*1.11e-3-t831.*t1066.*1.144e-2;
et1193 = t831.*t2147.*(-1.11e-3)+t815.*t2164.*1.11e-3;
et1194 = t1040.*(t88-t617).*1.144e-2-t2163.*(t88-t617).*1.11e-3;
et1195 = t2148.*(t86-t652).*1.11e-3;
et1196 = t461+t515+t517+t797+t1096+t1867+t1928+t1931+t1932+t1940+t2513.*2.019e-2+t2522+t2541+t2561-t7.*(t882-t2179).*4.9e-4;
et1197 = (t436-t448-t452+t460+t537+t796+t1097-t1644-t1875+t1890-t2065+t2205+t2227+t2523-t2537-t2560+t2989+t14.*(t639-t1128-t2181+dq5.*t13.*(t86-t652)).*2.019e-2+dq5.*t6.*(t86-t652).*2.75e-2).*(-3.38795);
et1198 = t609.*4.988e-2+t846.*4.988e-2;
et1199 = t847.*4.988e-2-t604.*t815.*1.12e-3;
et1200 = t572.*(t86-t652).*1.12e-3-t10.*t11.*t606.*1.12e-3;
et1201 = t230+t431+t644.*4.9e-4-t648.*2.019e-2+t657.*2.019e-2+t664.*4.9e-4;
et1202 = t13.*t573.*2.75e-2;
et1203 = t235+t349+t456+t457+t512-t1734+t1760-t1798+t1805.*1.9738e-1-t1812-t1861.*3.466000000000001e-2-t2073-t2085+t2171-t2747.*3.466000000000001e-2;
et1204 = t2751.*2.324e-2-t8.*(t640-t1136).*2.324e-2;
et1205 = t236+t237+t239+t463+t516+t518+t1772+t1962-t1976+t2173-t2614-t2637-t2647+t3009+dq7.*t1601.*2.324e-2+t15.*(t642+t896-t1137-t2220).*2.324e-2+dq7.*t8.*(t92-t663).*3.466000000000001e-2;
et1206 = dq7.*t15.*(t621-t864).*3.466000000000001e-2;
et1207 = t1218-t1791+t2357+t2372+t51.*t606+t58.*t606+t1066.*(t86-t652);
et1208 = (t2365+t2445.*1.12e-3-t2456+t2536-t2653-t2789+t2803+t2868+t1066.*(t86-t652).*8.8e-4).*(-1.0./2.0);
et1209 = t461+t515+t517+t797+t1096+t1886.*2.324e-2+t1888.*3.466000000000001e-2+t1942-t1959+t1993+t2482.*2.324e-2+t2483.*3.466000000000001e-2;
et1210 = t2513.*(-1.9738e-1)-t2617+t8.*(t932+t942+t2215+t7.*(t882-t2179)).*3.466000000000001e-2-t15.*(t932+t942+t2215+t7.*(t882-t2179)).*2.324e-2;
et1211 = dq6.*t14.*(t86-t652).*1.9738e-1;
et1212 = -t268-t685+t836.*2.019e-2+t839.*4.9e-4+t966.*4.9e-4+t13.*(t88-t617).*2.75e-2;
et1213 = t6.*t14.*(t88-t617).*(-2.019e-2);
et1214 = -t2674+t2931-t2935-t882.*(t614+t13.*(t86-t652)).*9.999999999999998e-6+t2179.*(t614+t13.*(t86-t652)).*9.999999999999998e-6;
et1215 = t573.*t1136.*(-5.539999999999998e-3)-t606.*t2165.*1.0e-5+t6.*t2783;
et1216 = t6.*t2949.*(-9.999999999999998e-6)+t831.*t2182.*5.539999999999998e-3+t6.*t3130;
et1217 = t815.*t2828.*(-1.0e-5)+(t86-t652).*(t639-t1128-t2181+dq5.*t13.*(t86-t652)).*1.0e-5;
et1218 = t629.*(t92-t663).*9.999999999999998e-6+t1130.*(t92-t663).*9.999999999999998e-6;
et1219 = t2217.*(t88-t617).*5.539999999999998e-3-t2212.*(t653-t838).*9.999999999999998e-6;
et1220 = dq5.*t6.*t609.*2.769999999999999e-3+dq5.*t6.*t846.*2.769999999999999e-3;
et1221 = dq5.*t6.*t847.*2.769999999999999e-3+dq5.*t13.*(t88-t617).*(t653-t838).*9.999999999999998e-6;
et1222 = t3132.*(t1386+t7.*(t88-t617)).*(-3.0e-5)+t877.*t2035.*5.0e-5;
et1223 = t948.*t2000.*(-5.0e-5)+t1207.*t2734.*3.0e-5;
et1224 = t2000.*t2217.*(-5.0e-5)+t2035.*t2182.*5.0e-5;
et1225 = t1700.*t2816.*5.000000000000004e-4+t1776.*t2832.*5.000000000000004e-4;
et1226 = t1738.*t3312.*(-3.0e-5)-(t614+t13.*(t86-t652)).*(t927-t935-t2183+t2206+dq6.*t14.*(t86-t652)).*5.000000000000004e-4;
et1227 = t640.*(t621-t864).*5.0e-5-t1136.*(t621-t864).*5.0e-5;
et1228 = t2735.*(t92-t663).*(-5.000000000000004e-4)-t2196.*(t648-t657).*5.000000000000004e-4;
et1229 = t3161.*(t653-t838).*5.000000000000004e-4+t1024.*(t631-t885+t1132-t2224).*3.0e-5;
et1230 = t2074.*(-t928+t984+t992+t2187+t2240).*(-3.0e-5)+(t921+t14.*(t86-t652)).*(t884+t1578-t2180+t14.*(t639-t1128-t2181+dq5.*t13.*(t86-t652))).*3.0e-5;
et1231 = t13.*t573.*(t642+t896-t1137-t2220).*5.0e-5+t13.*(t88-t617).*(t1487+t2219-t2864+dq6.*t7.*(t88-t617)).*5.0e-5;
et1232 = t13.*t831.*(t878-t1582+t2184+t7.*(t639-t1128-t2181+dq5.*t13.*(t86-t652))).*5.0e-5;
et1233 = -t2710+t2955-t2957-t573.*t1130.*2.840000000000012e-3-t13.*t2359.*4.466636216449161e-20;
et1234 = t606.*t2196.*(-1.0e-5)-t13.*t2953.*4.466636216449161e-20;
et1235 = t831.*t2179.*2.840000000000012e-3+t831.*t2460.*1.0e-5;
et1236 = t815.*t2816.*(-1.0e-5)+(t614+t13.*(t86-t652)).*(t882-t2179).*4.466636216449161e-20;
et1237 = t573.*(t640-t1136).*1.0e-5-t1749.*(t92-t663).*4.466636216449161e-20;
et1238 = t2212.*(t88-t617).*2.840000000000012e-3+t2488.*(t88-t617).*1.0e-5;
et1239 = t2832.*(t86-t652).*1.0e-5+t2477.*(t653-t838).*4.466636216449161e-20;
et1240 = t13.*t831.*(t639-t1128-t2181+dq5.*t13.*(t86-t652)).*4.466636216449161e-20;
et1241 = t522+t523+t527+t721+t982.*2.324e-2+t1269+t1957+t1960+t1963+t2006+t2258.*1.9738e-1+t2259.*2.324e-2+t2261.*3.466000000000001e-2+t2375+t2379+t2655;
et1242 = t3154.*(-3.466000000000001e-2)+t3155.*2.324e-2+t15.*t948.*3.466000000000001e-2-dq5.*t13.*t14.*(t88-t617).*1.9738e-1;
et1243 = t609.*1.11e-3+t846.*1.11e-3;
et1244 = t847.*1.11e-3-t604.*t815.*8.8e-4;
et1245 = t572.*(t86-t652).*8.8e-4-t10.*t11.*t606.*8.8e-4;
et1246 = t13.*t609.*2.769999999999999e-3+t13.*t846.*2.769999999999999e-3;
et1247 = t13.*t847.*2.769999999999999e-3-t606.*t827.*1.0e-5;
et1248 = t815.*t1206.*(-1.0e-5)+t1295.*(t86-t652).*1.0e-5;
et1249 = t6.*(t88-t617).*(t653-t838).*(-9.999999999999998e-6)+t6.*t831.*(t614+t13.*(t86-t652)).*9.999999999999998e-6;
et1250 = t6.*t573.*(t92-t663).*(-9.999999999999998e-6);
et1251 = t2444-t2840+t2842+t573.*t1130.*4.466636216449161e-20+t13.*t2359.*1.2e-4;
et1252 = t606.*t2196.*(-9.999999999999998e-6)+t13.*t2953.*1.2e-4;
et1253 = t831.*t2179.*(-4.466636216449161e-20)+t831.*t2460.*9.999999999999998e-6-t815.*t2816.*9.999999999999998e-6;
et1254 = (t614+t13.*(t86-t652)).*(t882-t2179).*(-1.2e-4)+t573.*(t640-t1136).*9.999999999999998e-6;
et1255 = t1749.*(t92-t663).*1.2e-4-t2212.*(t88-t617).*4.466636216449161e-20;
et1256 = t2488.*(t88-t617).*9.999999999999998e-6+t2832.*(t86-t652).*9.999999999999998e-6;
et1257 = t2477.*(t653-t838).*(-1.2e-4)-t13.*t831.*(t639-t1128-t2181+dq5.*t13.*(t86-t652)).*1.2e-4;
et1258 = -t2674+t2931-t2935-t573.*t1130.*1.0e-5+t13.*t2781-t606.*t2196.*2.769999999999999e-3;
et1259 = t13.*t2953.*9.999999999999998e-6+t831.*t2179.*1.0e-5+t13.*t3142;
et1260 = t831.*t2460.*2.769999999999999e-3-t815.*t2816.*2.769999999999999e-3;
et1261 = (t614+t13.*(t86-t652)).*(t882-t2179).*(-9.999999999999998e-6)+t573.*(t640-t1136).*2.769999999999999e-3;
et1262 = t1749.*(t92-t663).*9.999999999999998e-6+t2212.*(t88-t617).*1.0e-5;
et1263 = t2488.*(t88-t617).*2.769999999999999e-3+t2832.*(t86-t652).*2.769999999999999e-3;
et1264 = t2477.*(t653-t838).*(-9.999999999999998e-6);
et1265 = t2601.*(t853+t983+t2264+t2503).*1.089e-2+t2330.*(t884+t1578-t2180+t14.*(t639-t1128-t2181+dq5.*t13.*(t86-t652))).*1.089e-2;
et1266 = t3426.*(t1386+t7.*(t88-t617)).*(-2.2e-4)+t3163.*(t8.*(t92-t663)+t15.*(t621-t864)).*2.9e-4;
et1267 = t1207.*t3162.*2.2e-4-t1697.*t3336.*2.9e-4;
et1268 = t1700.*t3617.*2.2e-4+t1776.*t3620.*2.2e-4;
et1269 = t2289.*t3312.*1.089e-2+t2654.*t3168.*1.089e-2;
et1270 = t2315.*t3618.*(-2.9e-4)-t2576.*t3437.*2.9e-4;
et1271 = t2627.*(t933+t1888+t2483+t8.*(t932+t942+t2215+t7.*(t882-t2179))).*2.9e-4+(t1529+t15.*(t92-t663)).*(t673+t692-t1123-t1805).*1.089e-2;
et1272 = (t648-t657).*(t958-t2263+dq7.*t1601+t15.*(t642+t896-t1137-t2220)).*2.2e-4+t3619.*(t908+t15.*(t921+t14.*(t86-t652))).*2.9e-4;
et1273 = (t651-t1053).*(t631-t885+t1132-t2224).*1.089e-2+t2074.*(t939+t1853-t2482+t15.*(t932+t942+t2215+t7.*(t882-t2179))).*2.2e-4;
et1274 = -t3294+t3365.*7.950000000000001e-3+t3528+t3648+t3658-t3660-t3663+t2654.*(t884+t1578-t2180+t14.*(t639-t1128-t2181+dq5.*t13.*(t86-t652))).*2.2e-4;
et1275 = t3336.*(t8.*(t92-t663)+t15.*(t621-t864)).*2.900000000000001e-4;
et1276 = -t3196-t3253-t3262+t3406+t3452+t2074.*(t878-t1582+t2184+t7.*(t639-t1128-t2181+dq5.*t13.*(t86-t652))).*3.0e-5+t2196.*(t621-t864).*5.0e-5;
et1277 = t3312.*(t653-t838).*5.000000000000004e-4+t1207.*(t642+t896-t1137-t2220).*3.0e-5;
et1278 = t13.*t609.*1.0e-5+t13.*t846.*1.0e-5;
et1279 = t13.*t847.*1.0e-5-t606.*t827.*2.840000000000012e-3;
et1280 = t815.*t1206.*(-2.840000000000012e-3)+t1295.*(t86-t652).*2.840000000000012e-3;
et1281 = t6.*(t88-t617).*(t653-t838).*4.466636216449161e-20-t6.*t831.*(t614+t13.*(t86-t652)).*4.466636216449161e-20+t6.*t573.*(t92-t663).*4.466636216449161e-20;
et1282 = t2315.*(t1386+t7.*(t88-t617)).*7.950000000000001e-3+t1207.*t1697.*7.950000000000001e-3;
et1283 = t1700.*t2601.*2.2e-4+t1776.*t2654.*2.2e-4;
et1284 = t2289.*t2576.*(-2.900000000000001e-4)-t2330.*t2627.*2.900000000000001e-4;
et1285 = (t1529+t15.*(t92-t663)).*(t648-t657).*(-2.2e-4)-(t8.*(t92-t663)+t15.*(t621-t864)).*(t651-t1053).*2.900000000000001e-4;
et1286 = t2074.*(t908+t15.*(t921+t14.*(t86-t652))).*7.950000000000001e-3;
et1287 = t2735.*(t1529+t15.*(t92-t663)).*(-1.089e-2)-t3429.*(t1386+t7.*(t88-t617)).*2.2e-4;
et1288 = t3141.*(t8.*(t92-t663)+t15.*(t621-t864)).*2.9e-4+t1207.*t3159.*2.2e-4;
et1289 = t1700.*t3618.*1.089e-2+t1776.*t3619.*1.089e-2;
et1290 = t2315.*t3312.*(-2.2e-4)+t2601.*t3161.*1.089e-2;
et1291 = t2289.*t3617.*2.9e-4+t2330.*t3620.*2.9e-4;
et1292 = t2627.*t3444.*2.9e-4-t3336.*(t648-t657).*1.089e-2;
et1293 = (t908+t15.*(t921+t14.*(t86-t652))).*(t884+t1578-t2180+t14.*(t639-t1128-t2181+dq5.*t13.*(t86-t652))).*2.2e-4;
et1294 = t2654.*(t927-t935-t2183+t2206+dq6.*t14.*(t86-t652)).*(-1.089e-2);
et1295 = (t651-t1053).*(t958-t2263+dq7.*t1601+t15.*(t642+t896-t1137-t2220)).*2.9e-4-t2576.*(t987+t1806+t2261-t3154+t15.*t948).*2.9e-4;
et1296 = t1697.*(t631-t885+t1132-t2224).*2.2e-4-t2074.*(t926+t988+t1886+t2207+t15.*(-t928+t984+t992+t2187+t2240)).*2.2e-4;
et1297 = t3132.*(t1386+t7.*(t88-t617)).*2.32e-3+t877.*t2035.*4.000000000000028e-5;
et1298 = t948.*t2000.*(-4.000000000000028e-5)-t1207.*t2734.*2.32e-3;
et1299 = t2000.*t2217.*(-4.000000000000028e-5)+t2035.*t2182.*4.000000000000028e-5;
et1300 = t1700.*t2816.*(-3.0e-5)-t1776.*t2832.*3.0e-5;
et1301 = t1738.*t3312.*2.32e-3+(t614+t13.*(t86-t652)).*(t927-t935-t2183+t2206+dq6.*t14.*(t86-t652)).*3.0e-5;
et1302 = t640.*(t621-t864).*4.000000000000028e-5-t1136.*(t621-t864).*4.000000000000028e-5;
et1303 = t2735.*(t92-t663).*3.0e-5+t2196.*(t648-t657).*3.0e-5;
et1304 = t3161.*(t653-t838).*(-3.0e-5)-t1024.*(t631-t885+t1132-t2224).*2.32e-3;
et1305 = t2074.*(-t928+t984+t992+t2187+t2240).*2.32e-3-(t921+t14.*(t86-t652)).*(t884+t1578-t2180+t14.*(t639-t1128-t2181+dq5.*t13.*(t86-t652))).*2.32e-3;
et1306 = t13.*t573.*(t642+t896-t1137-t2220).*4.000000000000028e-5+t13.*(t88-t617).*(t1487+t2219-t2864+dq6.*t7.*(t88-t617)).*4.000000000000028e-5;
et1307 = t13.*t831.*(t878-t1582+t2184+t7.*(t639-t1128-t2181+dq5.*t13.*(t86-t652))).*4.000000000000028e-5;
et1308 = t2601.*(t853+t983+t2264+t2503).*2.9e-4+t2330.*(t884+t1578-t2180+t14.*(t639-t1128-t2181+dq5.*t13.*(t86-t652))).*2.9e-4;
et1309 = t3426.*(t1386+t7.*(t88-t617)).*(-2.900000000000001e-4)+t3163.*(t8.*(t92-t663)+t15.*(t621-t864)).*2.94e-3;
et1310 = t1207.*t3162.*2.900000000000001e-4-t1697.*t3336.*2.94e-3;
et1311 = t1700.*t3617.*2.900000000000001e-4+t1776.*t3620.*2.900000000000001e-4;
et1312 = t2289.*t3312.*2.9e-4+t2654.*t3168.*2.9e-4;
et1313 = t2315.*t3618.*(-2.94e-3)-t2576.*t3437.*2.94e-3;
et1314 = t2627.*(t933+t1888+t2483+t8.*(t932+t942+t2215+t7.*(t882-t2179))).*2.94e-3+(t1529+t15.*(t92-t663)).*(t673+t692-t1123-t1805).*2.9e-4;
et1315 = (t648-t657).*(t958-t2263+dq7.*t1601+t15.*(t642+t896-t1137-t2220)).*2.900000000000001e-4+t3619.*(t908+t15.*(t921+t14.*(t86-t652))).*2.94e-3;
et1316 = (t651-t1053).*(t631-t885+t1132-t2224).*2.9e-4+t2074.*(t939+t1853-t2482+t15.*(t932+t942+t2215+t7.*(t882-t2179))).*2.900000000000001e-4;
et1317 = -t433+t754+t907.*1.9738e-1+t908.*2.324e-2+t911.*3.466000000000001e-2-t8.*(t921+t14.*(t86-t652)).*3.466000000000001e-2;
et1318 = t15.*(t921+t14.*(t86-t652)).*2.324e-2-t7.*(t86-t652).*1.9738e-1;
et1319 = t2444-t2840+t2842-t882.*(t614+t13.*(t86-t652)).*1.2e-4+t2179.*(t614+t13.*(t86-t652)).*1.2e-4;
et1320 = t573.*t1136.*(-2.0e-5)+t6.*t2370.*1.2e-4;
et1321 = t606.*t2165.*4.466636216449161e-20-t6.*t2949.*1.2e-4;
et1322 = t831.*t2182.*2.0e-5+t815.*t2828.*4.466636216449161e-20;
et1323 = (t86-t652).*(t639-t1128-t2181+dq5.*t13.*(t86-t652)).*(-4.466636216449161e-20)+t629.*(t92-t663).*1.2e-4;
et1324 = t1130.*(t92-t663).*1.2e-4+t2217.*(t88-t617).*2.0e-5;
et1325 = t2212.*(t653-t838).*(-1.2e-4)+dq5.*t6.*t609.*9.999999999999998e-6;
et1326 = dq5.*t6.*t846.*9.999999999999998e-6+dq5.*t6.*t847.*9.999999999999998e-6;
et1327 = t6.*t2816.*(t88-t617).*1.2e-4+dq5.*t13.*(t88-t617).*(t653-t838).*1.2e-4;
et1328 = t522+t523+t527+t721+t1269+t1957+t1960+t1963+t2006+t2375+t2379+t2503.*1.9738e-1+t2514.*2.324e-2+t2516.*3.466000000000001e-2+t2655-t3152.*3.466000000000001e-2;
et1329 = t3153.*2.324e-2;
et1330 = -t2844-t2914-t2922+t3052+t3229-t3264+t3269+t3280-t3284+t3295+t3301+t3369+t3556-t3559+t3433.*(t614+t13.*(t86-t652)).*9.999999999999998e-6;
et1331 = t2832.*(t639-t1128-t2181+dq5.*t13.*(t86-t652)).*9.999999999999998e-6+t2974.*(t92-t663).*9.999999999999998e-6;
et1332 = t3422.*(t653-t838).*9.999999999999998e-6;
et1333 = -t3291+t3365.*2.900000000000001e-4+t3527+t3642+t3654-t3662-t3665+t2654.*(t884+t1578-t2180+t14.*(t639-t1128-t2181+dq5.*t13.*(t86-t652))).*2.9e-4;
et1334 = t3336.*(t8.*(t92-t663)+t15.*(t621-t864)).*2.94e-3;
et1335 = t2735.*(t1529+t15.*(t92-t663)).*(-2.9e-4)-t3429.*(t1386+t7.*(t88-t617)).*2.900000000000001e-4;
et1336 = t3141.*(t8.*(t92-t663)+t15.*(t621-t864)).*2.94e-3+t1207.*t3159.*2.900000000000001e-4;
et1337 = t1700.*t3618.*2.9e-4+t1776.*t3619.*2.9e-4;
et1338 = t2315.*t3312.*(-2.900000000000001e-4)+t2601.*t3161.*2.9e-4;
et1339 = t2289.*t3617.*2.94e-3+t2330.*t3620.*2.94e-3;
et1340 = t2627.*t3444.*2.94e-3-t3336.*(t648-t657).*2.9e-4;
et1341 = (t908+t15.*(t921+t14.*(t86-t652))).*(t884+t1578-t2180+t14.*(t639-t1128-t2181+dq5.*t13.*(t86-t652))).*2.900000000000001e-4;
et1342 = t2654.*(t927-t935-t2183+t2206+dq6.*t14.*(t86-t652)).*(-2.9e-4);
et1343 = (t651-t1053).*(t958-t2263+dq7.*t1601+t15.*(t642+t896-t1137-t2220)).*2.94e-3-t2576.*(t987+t1806+t2261-t3154+t15.*t948).*2.94e-3;
et1344 = t1697.*(t631-t885+t1132-t2224).*2.900000000000001e-4-t2074.*(t926+t988+t1886+t2207+t15.*(-t928+t984+t992+t2187+t2240)).*2.900000000000001e-4;
et1345 = t13.*t609.*9.999999999999998e-6+t13.*t846.*9.999999999999998e-6;
et1346 = t13.*t847.*9.999999999999998e-6+t606.*t827.*4.466636216449161e-20+t815.*t1206.*4.466636216449161e-20;
et1347 = t1295.*(t86-t652).*(-4.466636216449161e-20)-t6.*(t88-t617).*(t653-t838).*1.2e-4;
et1348 = t6.*t831.*(t614+t13.*(t86-t652)).*1.2e-4-t6.*t573.*(t92-t663).*1.2e-4;
et1349 = t949.*(t614+t13.*(t86-t652))+t2179.*(t614+t13.*(t86-t652))+t6.*t2370-t6.*t2949+t629.*(t92-t663)+t1130.*(t92-t663)-t2212.*(t653-t838)+t6.*t2816.*(t88-t617)+dq5.*t13.*(t88-t617).*(t653-t838);
et1350 = (-t2447-t2783-t2839+t2841+t3126+t3143+t3232+t2165.*(t92-t663).*1.2e-4+t2828.*(t653-t838).*1.2e-4).*(-1.0./2.0);
et1351 = -t3291+t3365.*2.900000000000001e-4+t3527+t3642+t3654-t3662-t3665+t2654.*(t884+t1578-t2180+t14.*(t639-t1128-t2181+dq5.*t13.*(t86-t652))).*2.9e-4;
et1352 = t3336.*(t8.*(t92-t663)+t15.*(t621-t864)).*2.94e-3;
et1353 = t1791.*(-3.844e-2)+t2455-t2790+t2804+t51.*t606.*3.844e-2;
et1354 = t58.*t606.*3.844e-2+t573.*t1070.*2.24e-3;
et1355 = t831.*t2147.*(-2.24e-3)+t1066.*(t86-t652).*3.844e-2;
et1356 = t2163.*(t88-t617).*(-2.24e-3);
et1357 = t2466-t2653-t2799+t2811+t51.*t606.*8.8e-4+t58.*t606.*8.8e-4;
et1358 = t573.*t1070.*2.22e-3-t831.*t2147.*2.22e-3;
et1359 = t1066.*(t86-t652).*8.8e-4-t2163.*(t88-t617).*2.22e-3;
et1360 = t461+t515+t517+t797+t926.*2.324e-2+t930.*3.466000000000001e-2-t935.*1.9738e-1+t1096+t1886.*2.324e-2;
et1361 = t1888.*3.466000000000001e-2+t1942-t1959+t1993+t2206.*1.9738e-1+t2207.*2.324e-2+t2208.*3.466000000000001e-2-t2617;
et1362 = t8.*(-t928+t984+t992+t2187+t2240).*(-3.466000000000001e-2)+t15.*(-t928+t984+t992+t2187+t2240).*2.324e-2+dq6.*t14.*(t86-t652).*1.9738e-1;
et1363 = (t573.*t1070.*-2.0+t831.*t2147.*2.0+t2163.*(t88-t617).*2.0).*(t2341+t2445.*4.988e-2-t2463-t2612+t2624-t2796+t2813+t2900+t1066.*(t86-t652).*1.11e-3);
et1364 = 1.0./2.0;
et1365 = t522+t523+t527+t721+t1269+t1839+t1872+t1881+t1908+t1924+t2256.*4.9e-4-t2258.*2.019e-2+t2554+t2569+t2590-dq5.*t7.*t13.*(t88-t617).*4.9e-4;
et1366 = dq5.*t13.*t14.*(t88-t617).*2.019e-2;
et1367 = -t3294+t3365.*7.950000000000001e-3+t3528+t3648+t3658-t3660-t3663+t2654.*(t884+t1578-t2180+t14.*(t639-t1128-t2181+dq5.*t13.*(t86-t652))).*2.2e-4;
et1368 = t3336.*(t8.*(t92-t663)+t15.*(t621-t864)).*2.900000000000001e-4;
et1369 = t573.*t1070+t606.*t1069-t831.*t2147+t815.*t2164-t2163.*(t88-t617)+t2148.*(t86-t652);
et1370 = (t2341+t2445.*4.988e-2-t2463-t2612+t2624-t2796+t2813+t2900+t1066.*(t86-t652).*1.11e-3)./2.0;
et1371 = t2765+t2818-t2907+t3067+t3215+t3235-t3238-t3246+t3268-t3273+t3375+t3551-t3555+t3433.*(t614+t13.*(t86-t652)).*1.2e-4+t2147.*(t639-t1128-t2181+dq5.*t13.*(t86-t652)).*4.466636216449161e-20;
et1372 = t2832.*(t639-t1128-t2181+dq5.*t13.*(t86-t652)).*1.2e-4+t2974.*(t92-t663).*1.2e-4;
et1373 = t3422.*(t653-t838).*1.2e-4;
et1374 = (t569.*t573+t831.*t1066-t1040.*(t88-t617)).*(t2388+t2445.*1.11e-3-t2467+t2496-t2693-t2798+t2810+t2829+t1066.*(t86-t652).*1.144e-2);
et1375 = -1.0./2.0;
et1376 = t236+t237+t239+t463+t516+t518+t1772+t1962-t1976+t2173-t2614-t2637-t2647+t3009+dq7.*t1601.*2.324e-2+t15.*(t642+t896-t1137-t2220).*2.324e-2+dq7.*t8.*(t92-t663).*3.466000000000001e-2;
et1377 = dq7.*t15.*(t621-t864).*3.466000000000001e-2;
et1378 = t235-t238+t456+t457+t512-t691.*2.324e-2-t698.*3.466000000000001e-2+t705.*1.9738e-1+t1219.*1.9738e-1;
et1379 = t1220.*2.324e-2+t1226.*3.466000000000001e-2-t1734+t1760-t1798-t1812-t2073-t2085+t2171-t2753.*3.466000000000001e-2;
et1380 = t2754.*2.324e-2;
et1381 = t2455-t2790+t2804-t569.*t573.*8.8e-4+t573.*t1070.*1.12e-3;
et1382 = t606.*t1069.*1.12e-3-t831.*t1066.*8.8e-4;
et1383 = t831.*t2147.*(-1.12e-3)+t815.*t2164.*1.12e-3;
et1384 = t1040.*(t88-t617).*8.8e-4-t2163.*(t88-t617).*1.12e-3;
et1385 = t2148.*(t86-t652).*1.12e-3;
et1386 = t2315.*(t1386+t7.*(t88-t617)).*2.900000000000001e-4+t1207.*t1697.*2.900000000000001e-4;
et1387 = t1700.*t2601.*2.9e-4+t1776.*t2654.*2.9e-4;
et1388 = t2289.*t2576.*(-2.94e-3)-t2330.*t2627.*2.94e-3;
et1389 = (t1529+t15.*(t92-t663)).*(t648-t657).*(-2.9e-4)-(t8.*(t92-t663)+t15.*(t621-t864)).*(t651-t1053).*2.94e-3;
et1390 = t2074.*(t908+t15.*(t921+t14.*(t86-t652))).*2.900000000000001e-4;
et1391 = -t3289+t3365.*2.2e-4+t3526+t3644+t3655-t3661-t3664+t2654.*(t884+t1578-t2180+t14.*(t639-t1128-t2181+dq5.*t13.*(t86-t652))).*1.089e-2;
et1392 = t3336.*(t8.*(t92-t663)+t15.*(t621-t864)).*2.9e-4;
et1393 = t1776.*(t614+t13.*(t86-t652)).*3.0e-5+t2074.*(t921+t14.*(t86-t652)).*2.32e-3;
et1394 = t1738.*(t1386+t7.*(t88-t617)).*2.32e-3+t1024.*t1207.*2.32e-3;
et1395 = t1700.*(t653-t838).*3.0e-5-(t92-t663).*(t648-t657).*3.0e-5;
et1396 = t13.*t831.*t2035.*4.000000000000028e-5+t13.*t573.*(t621-t864).*4.000000000000028e-5;
et1397 = t13.*t2000.*(t88-t617).*(-4.000000000000028e-5);
et1398 = t3132.*(t1386+t7.*(t88-t617)).*4.000000000000028e-5+t877.*t2035.*2.81e-3;
et1399 = t948.*t2000.*(-2.81e-3)-t1207.*t2734.*4.000000000000028e-5;
et1400 = t2000.*t2217.*(-2.81e-3)+t2035.*t2182.*2.81e-3;
et1401 = t1700.*t2816.*5.0e-5+t1776.*t2832.*5.0e-5;
et1402 = t1738.*t3312.*4.000000000000028e-5-(t614+t13.*(t86-t652)).*(t927-t935-t2183+t2206+dq6.*t14.*(t86-t652)).*5.0e-5;
et1403 = t640.*(t621-t864).*2.81e-3-t1136.*(t621-t864).*2.81e-3;
et1404 = t2735.*(t92-t663).*(-5.0e-5)-t2196.*(t648-t657).*5.0e-5;
et1405 = t3161.*(t653-t838).*5.0e-5-t1024.*(t631-t885+t1132-t2224).*4.000000000000028e-5;
et1406 = t2074.*(-t928+t984+t992+t2187+t2240).*4.000000000000028e-5-(t921+t14.*(t86-t652)).*(t884+t1578-t2180+t14.*(t639-t1128-t2181+dq5.*t13.*(t86-t652))).*4.000000000000028e-5;
et1407 = t13.*t573.*(t642+t896-t1137-t2220).*2.81e-3+t13.*(t88-t617).*(t1487+t2219-t2864+dq6.*t7.*(t88-t617)).*2.81e-3;
et1408 = t13.*t831.*(t878-t1582+t2184+t7.*(t639-t1128-t2181+dq5.*t13.*(t86-t652))).*2.81e-3;
et1409 = t2074.*(t932+t942+t2215+t7.*(t882-t2179)).*(-4.000000000000028e-5)-t1776.*(t878-t1582+t2184+t7.*(t639-t1128-t2181+dq5.*t13.*(t86-t652))).*4.000000000000028e-5;
et1410 = t2832.*(t921+t14.*(t86-t652)).*2.81e-3+t3168.*(t614+t13.*(t86-t652)).*5.0e-5;
et1411 = t3131.*(t1386+t7.*(t88-t617)).*4.000000000000028e-5+(t653-t838).*(t853+t983+t2264+t2503).*5.0e-5;
et1412 = t1024.*t2196.*(-2.81e-3)-t1207.*t2732.*4.000000000000028e-5;
et1413 = t2000.*t2488.*(-2.81e-3)+t2035.*t2460.*2.81e-3;
et1414 = t1738.*t2816.*(-2.81e-3)+(t621-t864).*(t640-t1136).*2.81e-3;
et1415 = t1700.*(t1487+t2219-t2864+dq6.*t7.*(t88-t617)).*4.000000000000028e-5+(t92-t663).*(t673+t692-t1123-t1805).*5.0e-5;
et1416 = (t648-t657).*(t642+t896-t1137-t2220).*(-4.000000000000028e-5)+t13.*t573.*(t631-t885+t1132-t2224).*5.0e-5;
et1417 = t13.*t831.*(t884+t1578-t2180+t14.*(t639-t1128-t2181+dq5.*t13.*(t86-t652))).*5.0e-5-t13.*t3312.*(t88-t617).*5.0e-5;
et1418 = t609.*1.12e-3+t846.*1.12e-3;
et1419 = t847.*1.12e-3-t604.*t815.*3.844e-2;
et1420 = t572.*(t86-t652).*3.844e-2-t10.*t11.*t606.*3.844e-2;
et1421 = t2891+t2923+t2941+t3011-t3226+t3277-t3279-t3292+t3296-t3311+t3363+t3479.*1.0e-5+t3561+t3433.*(t614+t13.*(t86-t652)).*4.466636216449161e-20;
et1422 = t2147.*(t639-t1128-t2181+dq5.*t13.*(t86-t652)).*2.840000000000012e-3+t2832.*(t639-t1128-t2181+dq5.*t13.*(t86-t652)).*4.466636216449161e-20;
et1423 = t2974.*(t92-t663).*4.466636216449161e-20+t3422.*(t653-t838).*4.466636216449161e-20;
et1424 = t461+t515+t517+t797-t928.*4.9e-4+t935.*2.019e-2+t1096+t1867+t1928+t1931+t1932+t1940-t2206.*2.019e-2+t2240.*4.9e-4+t2522+t2541+t2561;
et1425 = (t436-t448-t452+t460+t537+t796+t1097-t1644-t1875+t1890-t2065+t2205+t2227+t2523-t2537-t2560+t2989+t14.*(t639-t1128-t2181+dq5.*t13.*(t86-t652)).*2.019e-2+dq5.*t6.*(t86-t652).*2.75e-2).*3.38795;
et1426 = -t433+t754-t907.*2.019e-2+t921.*4.9e-4+t13.*t831.*2.75e-2+t7.*(t86-t652).*2.019e-2;
et1427 = t14.*(t86-t652).*4.9e-4;
et1428 = t1776.*(t614+t13.*(t86-t652)).*5.000000000000004e-4+t2074.*(t921+t14.*(t86-t652)).*3.0e-5;
et1429 = t1738.*(t1386+t7.*(t88-t617)).*3.0e-5+t1024.*t1207.*3.0e-5;
et1430 = t1700.*(t653-t838).*5.000000000000004e-4-(t92-t663).*(t648-t657).*5.000000000000004e-4;
et1431 = t13.*t831.*t2035.*(-5.0e-5)-t13.*t573.*(t621-t864).*5.0e-5;
et1432 = t13.*t2000.*(t88-t617).*5.0e-5;
et1433 = t230+t431+t648.*1.9738e-1+t649.*2.324e-2+t651.*3.466000000000001e-2-t657.*1.9738e-1;
et1434 = t1053.*(-3.466000000000001e-2)+t1056.*2.324e-2;
et1435 = t2074.*(t932+t942+t2215+t7.*(t882-t2179)).*3.0e-5+t1776.*(t878-t1582+t2184+t7.*(t639-t1128-t2181+dq5.*t13.*(t86-t652))).*3.0e-5;
et1436 = t2832.*(t921+t14.*(t86-t652)).*5.0e-5+t3168.*(t614+t13.*(t86-t652)).*5.000000000000004e-4;
et1437 = t3131.*(t1386+t7.*(t88-t617)).*(-3.0e-5)+(t653-t838).*(t853+t983+t2264+t2503).*5.000000000000004e-4;
et1438 = t1024.*t2196.*(-5.0e-5)+t1207.*t2732.*3.0e-5;
et1439 = t2000.*t2488.*(-5.0e-5)+t2035.*t2460.*5.0e-5;
et1440 = t1738.*t2816.*(-5.0e-5)+(t621-t864).*(t640-t1136).*5.0e-5;
et1441 = t1700.*(t1487+t2219-t2864+dq6.*t7.*(t88-t617)).*(-3.0e-5)+(t92-t663).*(t673+t692-t1123-t1805).*5.000000000000004e-4;
et1442 = (t648-t657).*(t642+t896-t1137-t2220).*3.0e-5+t13.*t573.*(t631-t885+t1132-t2224).*5.000000000000004e-4;
et1443 = t13.*t831.*(t884+t1578-t2180+t14.*(t639-t1128-t2181+dq5.*t13.*(t86-t652))).*5.000000000000004e-4-t13.*t3312.*(t88-t617).*5.000000000000004e-4;
et1444 = t2601.*(t853+t983+t2264+t2503).*2.2e-4+t2330.*(t884+t1578-t2180+t14.*(t639-t1128-t2181+dq5.*t13.*(t86-t652))).*2.2e-4;
et1445 = t3426.*(t1386+t7.*(t88-t617)).*(-7.950000000000001e-3)+t3163.*(t8.*(t92-t663)+t15.*(t621-t864)).*2.900000000000001e-4;
et1446 = t1207.*t3162.*7.950000000000001e-3-t1697.*t3336.*2.900000000000001e-4;
et1447 = t1700.*t3617.*7.950000000000001e-3+t1776.*t3620.*7.950000000000001e-3;
et1448 = t2289.*t3312.*2.2e-4+t2654.*t3168.*2.2e-4;
et1449 = t2315.*t3618.*(-2.900000000000001e-4)-t2576.*t3437.*2.900000000000001e-4;
et1450 = t2627.*(t933+t1888+t2483+t8.*(t932+t942+t2215+t7.*(t882-t2179))).*2.900000000000001e-4+(t1529+t15.*(t92-t663)).*(t673+t692-t1123-t1805).*2.2e-4;
et1451 = (t648-t657).*(t958-t2263+dq7.*t1601+t15.*(t642+t896-t1137-t2220)).*7.950000000000001e-3+t3619.*(t908+t15.*(t921+t14.*(t86-t652))).*2.900000000000001e-4;
et1452 = (t651-t1053).*(t631-t885+t1132-t2224).*2.2e-4+t2074.*(t939+t1853-t2482+t15.*(t932+t942+t2215+t7.*(t882-t2179))).*7.950000000000001e-3;
et1453 = t2462-t2797+t2814-t569.*t573.*1.11e-3+t573.*t1070.*4.988e-2;
et1454 = t606.*t1069.*4.988e-2-t831.*t1066.*1.11e-3;
et1455 = t831.*t2147.*(-4.988e-2)+t815.*t2164.*4.988e-2;
et1456 = t1040.*(t88-t617).*1.11e-3-t2163.*(t88-t617).*4.988e-2;
et1457 = t2148.*(t86-t652).*4.988e-2;
et1458 = -t3196-t3253-t3262+t3406+t3452+t2074.*(t878-t1582+t2184+t7.*(t639-t1128-t2181+dq5.*t13.*(t86-t652))).*3.0e-5+t2196.*(t621-t864).*5.0e-5;
et1459 = t3312.*(t653-t838).*5.000000000000004e-4+t1207.*(t642+t896-t1137-t2220).*3.0e-5;
et1460 = t2074.*(t932+t942+t2215+t7.*(t882-t2179)).*2.32e-3+t1776.*(t878-t1582+t2184+t7.*(t639-t1128-t2181+dq5.*t13.*(t86-t652))).*2.32e-3;
et1461 = t2832.*(t921+t14.*(t86-t652)).*(-4.000000000000028e-5)+t3168.*(t614+t13.*(t86-t652)).*3.0e-5;
et1462 = t3131.*(t1386+t7.*(t88-t617)).*(-2.32e-3)+(t653-t838).*(t853+t983+t2264+t2503).*3.0e-5;
et1463 = t1024.*t2196.*4.000000000000028e-5+t1207.*t2732.*2.32e-3;
et1464 = t2000.*t2488.*4.000000000000028e-5-t2035.*t2460.*4.000000000000028e-5;
et1465 = t1738.*t2816.*4.000000000000028e-5-(t621-t864).*(t640-t1136).*4.000000000000028e-5;
et1466 = t1700.*(t1487+t2219-t2864+dq6.*t7.*(t88-t617)).*(-2.32e-3)+(t92-t663).*(t673+t692-t1123-t1805).*3.0e-5;
et1467 = (t648-t657).*(t642+t896-t1137-t2220).*2.32e-3+t13.*t573.*(t631-t885+t1132-t2224).*3.0e-5;
et1468 = t13.*t831.*(t884+t1578-t2180+t14.*(t639-t1128-t2181+dq5.*t13.*(t86-t652))).*3.0e-5-t13.*t3312.*(t88-t617).*3.0e-5;
et1469 = -t3289+t3365.*2.2e-4+t3526+t3644+t3655-t3661-t3664+t2654.*(t884+t1578-t2180+t14.*(t639-t1128-t2181+dq5.*t13.*(t86-t652))).*1.089e-2;
et1470 = t3336.*(t8.*(t92-t663)+t15.*(t621-t864)).*2.9e-4;
et1471 = t2735.*(t1529+t15.*(t92-t663)).*(-2.2e-4)-t3429.*(t1386+t7.*(t88-t617)).*7.950000000000001e-3;
et1472 = t3141.*(t8.*(t92-t663)+t15.*(t621-t864)).*2.900000000000001e-4+t1207.*t3159.*7.950000000000001e-3;
et1473 = t1700.*t3618.*2.2e-4+t1776.*t3619.*2.2e-4;
et1474 = t2315.*t3312.*(-7.950000000000001e-3)+t2601.*t3161.*2.2e-4;
et1475 = t2289.*t3617.*2.900000000000001e-4+t2330.*t3620.*2.900000000000001e-4;
et1476 = t2627.*t3444.*2.900000000000001e-4-t3336.*(t648-t657).*2.2e-4;
et1477 = (t908+t15.*(t921+t14.*(t86-t652))).*(t884+t1578-t2180+t14.*(t639-t1128-t2181+dq5.*t13.*(t86-t652))).*7.950000000000001e-3;
et1478 = t2654.*(t927-t935-t2183+t2206+dq6.*t14.*(t86-t652)).*(-2.2e-4);
et1479 = (t651-t1053).*(t958-t2263+dq7.*t1601+t15.*(t642+t896-t1137-t2220)).*2.900000000000001e-4-t2576.*(t987+t1806+t2261-t3154+t15.*t948).*2.900000000000001e-4;
et1480 = t1697.*(t631-t885+t1132-t2224).*7.950000000000001e-3-t2074.*(t926+t988+t1886+t2207+t15.*(-t928+t984+t992+t2187+t2240)).*7.950000000000001e-3;
et1481 = -t2711+t2801-t2954+t2956-t3179+t3181+t2165.*(t92-t663).*4.466636216449161e-20+t2816.*(t88-t617).*1.0e-5;
et1482 = t2828.*(t653-t838).*4.466636216449161e-20;
et1483 = t1776.*(t614+t13.*(t86-t652)).*(-5.0e-5)+t2074.*(t921+t14.*(t86-t652)).*4.000000000000028e-5;
et1484 = t1738.*(t1386+t7.*(t88-t617)).*4.000000000000028e-5+t1024.*t1207.*4.000000000000028e-5;
et1485 = t1700.*(t653-t838).*(-5.0e-5)+(t92-t663).*(t648-t657).*5.0e-5;
et1486 = t13.*t831.*t2035.*2.81e-3+t13.*t573.*(t621-t864).*2.81e-3;
et1487 = t13.*t2000.*(t88-t617).*(-2.81e-3);
et1488 = t13.*t2359+t13.*t2948+t13.*t2953-(t614+t13.*(t86-t652)).*(t882-t2179)+t1749.*(t92-t663)-t2477.*(t653-t838);
et1489 = (-t2447-t2783-t2839+t2841+t3126+t3143+t3232+t2165.*(t92-t663).*1.2e-4+t2828.*(t653-t838).*1.2e-4)./2.0;
et1490 = (t3829.*(et1169+et1170+et1171+et1172+et1173))./2.0+t3833.*(et1174+et1175).*3.5432e-1-(t3192.*(et1176+et1177+et1178+et1179))./2.0+(t3272.*(et1180+et1181+et1182+et1183+et1184+et1185+et1186+et1187+et1188))./2.0+((t1843+t2621+t2648+t573.*t1130-t831.*t2179-t2212.*(t88-t617)).*(et1189+et1190))./2.0+((t859-t1791+t1066.*(t86-t652)).*(et1191+et1192+et1193+et1194+et1195))./2.0+(t3843.*(t1700.*t2601+t1776.*t2654-(t1529+t15.*(t92-t663)).*(t648-t657)))./2.0-(t3844.*(t2289.*t2576+t2330.*t2627+(t8.*(t92-t663)+t15.*(t621-t864)).*(t651-t1053)))./2.0;
et1491 = (t3820.*(t2832.*(t921+t14.*(t86-t652))-t1024.*t2196-t2000.*t2488+t2035.*t2460-t1738.*t2816+(t621-t864).*(t640-t1136)))./2.0+et1196.*et1197-((t2056-t2360-t2788-t2807+t3051+t2962.*(t88-t617)).*(et1198+et1199+et1200))./2.0+t3790.*(et1201+et1202).*3.38795-(et1203+et1204).*(et1205+et1206).*3.5432e-1+et1207.*et1208;
et1492 = t3779.*(t33.*(-1.8866e-1)+t82.*1.8866e-1+t6.*t573.*5.000000000000001e-5+t13.*t573.*2.37e-3).*(-3.41e+2./1.0e+2);
et1493 = t3786.*(t86.*(-1.8866e-1)+t652.*1.8866e-1+t6.*t831.*5.000000000000001e-5+t13.*t831.*2.37e-3).*(-3.41e+2./1.0e+2)+t3798.*(et1209+et1210+et1211).*3.5432e-1;
et1494 = (et1212+et1213).*(t221.*(2.1e+1./5.0e+1)+t223.*(2.1e+1./5.0e+1)-t542+t547+t548-t554+t580+t581+t583+t800+t1424+t1726+t1856+t1898+t1934+t2042+t2198+t2231+t2253+t2558+t2581+t2587+t2602+t2991+t2997+t3066+t3075+t3082+t3495+t3498).*(-3.38795)+((t2370-t2949+t2816.*(t88-t617)).*(et1214+et1215+et1216+et1217+et1218+et1219+et1220+et1221))./2.0+((-t2961+t3358+t3312.*(t653-t838)).*(et1222+et1223+et1224+et1225+et1226+et1227+et1228+et1229+et1230+et1231+et1232))./2.0-(t3788.*(t573.*t1136.*-2.0+t831.*t2182.*2.0+t2217.*(t88-t617).*2.0+dq5.*t6.*t609+dq5.*t6.*t846+dq5.*t6.*t847))./2.0+(t3272.*(et1233+et1234+et1235+et1236+et1237+et1238+et1239+et1240))./2.0;
et1495 = ((t1218+t2357+t2372).*(t2365+t2445.*1.12e-3-t2456+t2536-t2653-t2789+t2803+t2868+t1066.*(t86-t652).*8.8e-4))./2.0;
et1496 = t3796.*(et1241+et1242).*3.5432e-1+(t3546.*(et1243+et1244+et1245))./2.0-(t3783.*(et1246+et1247+et1248+et1249+et1250))./2.0+((t3031+t2165.*(t92-t663)+t2828.*(t653-t838)).*(et1251+et1252+et1253+et1254+et1255+et1256+et1257))./2.0-((t2370-t2949+t2816.*(t88-t617)).*(et1258+et1259+et1260+et1261+et1262+et1263+et1264))./2.0-((-t3113+t3418+t2654.*(t884+t1578-t2180+t14.*(t639-t1128-t2181+dq5.*t13.*(t86-t652)))).*(et1265+et1266+et1267+et1268+et1269+et1270+et1271+et1272+et1273))./2.0;
et1497 = (-t3426.*(t1386+t7.*(t88-t617))+t1207.*t3162+t1700.*t3617+t1776.*t3620+(t648-t657).*(t958-t2263+dq7.*t1601+t15.*(t642+t896-t1137-t2220))+t2074.*(t939+t1853-t2482+t15.*(t932+t942+t2215+t7.*(t882-t2179)))).*(et1274+et1275).*(-1.0./2.0)-((t3168.*(t614+t13.*(t86-t652))+(t653-t838).*(t853+t983+t2264+t2503)+(t92-t663).*(t673+t692-t1123-t1805)+t13.*t573.*(t631-t885+t1132-t2224)+t13.*t831.*(t884+t1578-t2180+t14.*(t639-t1128-t2181+dq5.*t13.*(t86-t652)))-t13.*t3312.*(t88-t617)).*(et1276+et1277))./2.0;
et1498 = t3674.*(t235+t349+t456+t457+t512+t1667+t1702+t1710+t1718+t1720+t1802.*4.9e-4-t1805.*2.019e-2+t2072+t2111+t2125).*(-3.38795);
et1499 = t3776.*(t522+t523+t527+t721+t1269+t1839+t1872+t1881+t1908+t1924+t2501.*4.9e-4-t2503.*2.019e-2+t2554+t2569+t2590).*(-3.38795)+(t3845.*(t2315.*(t1386+t7.*(t88-t617))+t1207.*t1697+t2074.*(t908+t15.*(t921+t14.*(t86-t652)))))./2.0-((t2407+t2563+t3085-t3092-t3122+t2147.*(t639-t1128-t2181+dq5.*t13.*(t86-t652))).*(et1278+et1279+et1280+et1281))./2.0;
et1500 = (t3838.*(et1282+et1283+et1284+et1285+et1286))./2.0-(t3818.*(t3132.*(t1386+t7.*(t88-t617))-t1207.*t2734+t1738.*t3312-t1024.*(t631-t885+t1132-t2224)+t2074.*(-t928+t984+t992+t2187+t2240)-(t921+t14.*(t86-t652)).*(t884+t1578-t2180+t14.*(t639-t1128-t2181+dq5.*t13.*(t86-t652)))))./2.0+((-t3113+t3418+t2654.*(t884+t1578-t2180+t14.*(t639-t1128-t2181+dq5.*t13.*(t86-t652)))).*(et1287+et1288+et1289+et1290+et1291+et1292+et1293+et1294+et1295+et1296))./2.0;
et1501 = (t3377+t2074.*(t878-t1582+t2184+t7.*(t639-t1128-t2181+dq5.*t13.*(t86-t652)))+t1207.*(t642+t896-t1137-t2220)).*(et1297+et1298+et1299+et1300+et1301+et1302+et1303+et1304+et1305+et1306+et1307).*(-1.0./2.0)+(t3789.*(et1308+et1309+et1310+et1311+et1312+et1313+et1314+et1315+et1316))./2.0-t3835.*(et1317+et1318).*3.5432e-1+(t3788.*(-t606.*t2196+t831.*t2460-t815.*t2816+t573.*(t640-t1136)+t2488.*(t88-t617)+t2832.*(t86-t652)))./2.0-((t3031+t2165.*(t92-t663)+t2828.*(t653-t838)).*(et1319+et1320+et1321+et1322+et1323+et1324+et1325+et1326+et1327))./2.0-t3796.*(et1328+et1329).*3.5432e-1;
et1502 = (t3841.*(t1776.*(t614+t13.*(t86-t652))+t1700.*(t653-t838)-(t92-t663).*(t648-t657)))./2.0-(t3820.*(t881.*t2000+t877.*t2035-t2000.*t2217+t2035.*t2182+t640.*(t621-t864)-t1136.*(t621-t864)+t13.*t573.*(t642+t896-t1137-t2220)+t13.*(t88-t617).*(t1487+t2219-t2864+dq6.*t7.*(t88-t617))+t13.*t831.*(t878-t1582+t2184+t7.*(t639-t1128-t2181+dq5.*t13.*(t86-t652)))))./2.0;
et1503 = t3818.*(t2074.*(t932+t942+t2215+t7.*(t882-t2179))+t1776.*(t878-t1582+t2184+t7.*(t639-t1128-t2181+dq5.*t13.*(t86-t652)))-t3131.*(t1386+t7.*(t88-t617))+t1207.*t2732-t1700.*(t1487+t2219-t2864+dq6.*t7.*(t88-t617))+(t648-t657).*(t642+t896-t1137-t2220)).*(-1.0./2.0)+((t13.*t609+t13.*t846+t13.*t847).*(et1330+et1331+et1332))./2.0;
